simulink model "model"  (R2014a)
(part 1 of 5)
settings: Solver=VariableStepAuto  StartTime=0.0  StopTime=10.0  RelTol=1e-3
libraries: powerlib x1195
settings Model: Creator=lej  LastModifiedBy=leimhofe
settings DataIOCC: SaveFormat=Dataset
settings OptimizationCC: SimCompilerOptimization=off
settings DebuggingCC: MergeDetectMultiDrivingBlocksExec=error  SolverPrmCheckMsg=none  FrameProcessingCompatibilityMsg=error  AllowSymbolicDim=off
settings HardwareCC: ProdBitPerPointer=64  ProdLargestAtomicFloat=Float  ProdIntDivRoundTo=Zero  ProdEndianess=LittleEndian  ProdWordSize=64  ProdHWDeviceType=Intel->x86-64 (Windows64)
settings RTWCC: RTWCompilerOptimization=off
settings GRTTargetCC: GeneratePreprocessorConditionals=Use local settings
settings ConfigComp: CovMetricSettings=dw  CovHtmlReporting=on  CovSaveCumulativeToWorkspaceVar=on  CovSaveSingleToWorkspaceVar=on  CovExternalEMLEnable=off

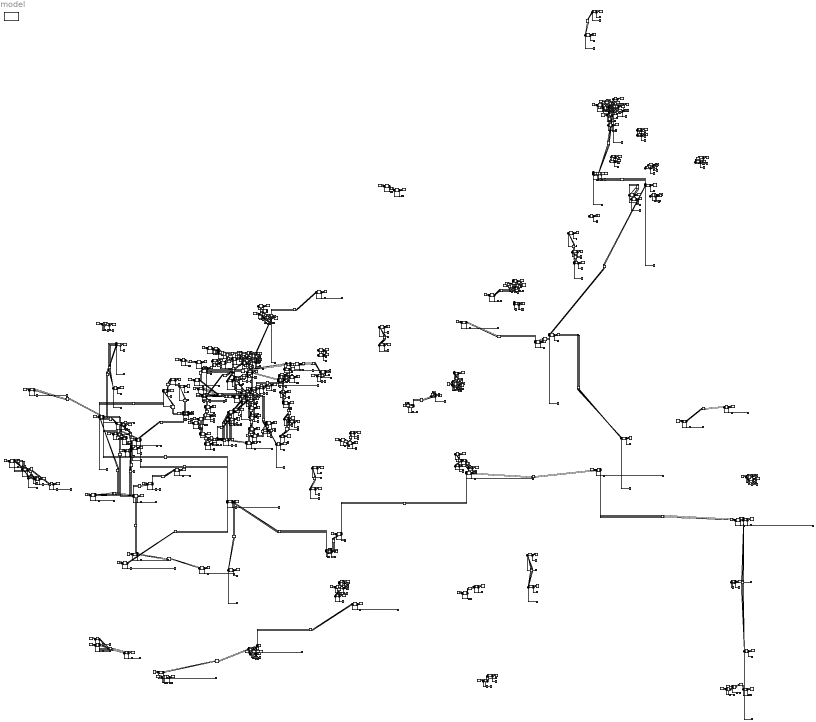
== system model ==
  note: 110000 Volts Power Line
  note: 220000 Volts Power Line
  note: 500000 Volts Power Line
  "110_кВ_\"Лесная_Тормозная\"_CN_242610017_110000_CN_242614771_110000" : powerlib/Elements/Distributed Parameters Line  Phases=3  Frequency=60  Resistance=[0.01273 0.3864]  Inductance="[0.9337e-3  4.1264e-3]"  Capacitance=[12.74e-9 7.751e-9]  Length=5.1805  x1=[0 0 0 0; 0.0001244 0 0 0; 0.0002488 0 0 0; 0.0003733 0 0 0; 0.0004977 0 0 0; 0.0006221 0 0 0]  x2=[0 0 0 0; 0.0001244 0 0 0; 0.0002488 0 0 0; 0.0003733 0 0 0; 0.0004977 0 0 0; 0.0006221 0 0 0]  x3=[0 0 0 0; 0.0001244 0 0 0; 0.0002488 0 0 0; 0.0003733 0 0 0; 0.0004977 0 0 0; 0.0006221 0 0 0]  x4=[0 0 0 0; 0.0001244 0 0 0; 0.0002488 0 0 0; 0.0003733 0 0 0; 0.0004977 0 0 0; 0.0006221 0 0 0]  x5=0  V1=ones(3,3)  V2=ones(3,3)  I1=ones(3,3)  I2=ones(3,3)  nHarmo=1  Measurements=None
  110_кВ_CN_138632781_110000_CN_138722426_110000 : powerlib/Elements/Distributed Parameters Line  Phases=3  Frequency=60  Resistance=[0.01273 0.3864]  Inductance="[0.9337e-3  4.1264e-3]"  Capacitance=[12.74e-9 7.751e-9]  Length=57.9129  x1=[0 0 0 0; 0.0001244 0 0 0; 0.0002488 0 0 0; 0.0003733 0 0 0; 0.0004977 0 0 0; 0.0006221 0 0 0]  x2=[0 0 0 0; 0.0001244 0 0 0; 0.0002488 0 0 0; 0.0003733 0 0 0; 0.0004977 0 0 0; 0.0006221 0 0 0]  x3=[0 0 0 0; 0.0001244 0 0 0; 0.0002488 0 0 0; 0.0003733 0 0 0; 0.0004977 0 0 0; 0.0006221 0 0 0]  x4=[0 0 0 0; 0.0001244 0 0 0; 0.0002488 0 0 0; 0.0003733 0 0 0; 0.0004977 0 0 0; 0.0006221 0 0 0]  x5=0  V1=ones(3,3)  V2=ones(3,3)  I1=ones(3,3)  I2=ones(3,3)  nHarmo=1  Measurements=None
  110_кВ_CN_138632781_110000_CN_140940409_110000 : powerlib/Elements/Distributed Parameters Line  Phases=3  Frequency=60  Resistance=[0.01273 0.3864]  Inductance="[0.9337e-3  4.1264e-3]"  Capacitance=[12.74e-9 7.751e-9]  Length=56.8666  x1=[0 0 0 0; 0.0001244 0 0 0; 0.0002488 0 0 0; 0.0003733 0 0 0; 0.0004977 0 0 0; 0.0006221 0 0 0]  x2=[0 0 0 0; 0.0001244 0 0 0; 0.0002488 0 0 0; 0.0003733 0 0 0; 0.0004977 0 0 0; 0.0006221 0 0 0]  x3=[0 0 0 0; 0.0001244 0 0 0; 0.0002488 0 0 0; 0.0003733 0 0 0; 0.0004977 0 0 0; 0.0006221 0 0 0]  x4=[0 0 0 0; 0.0001244 0 0 0; 0.0002488 0 0 0; 0.0003733 0 0 0; 0.0004977 0 0 0; 0.0006221 0 0 0]  x5=0  V1=ones(3,3)  V2=ones(3,3)  I1=ones(3,3)  I2=ones(3,3)  nHarmo=1  Measurements=None
  110_кВ_CN_138632781_110000_CN_140944227_110000 : powerlib/Elements/Distributed Parameters Line  Phases=3  Frequency=60  Resistance=[0.01273 0.3864]  Inductance="[0.9337e-3  4.1264e-3]"  Capacitance=[12.74e-9 7.751e-9]  Length=80.834  x1=[0 0 0 0; 0.0001244 0 0 0; 0.0002488 0 0 0; 0.0003733 0 0 0; 0.0004977 0 0 0; 0.0006221 0 0 0]  x2=[0 0 0 0; 0.0001244 0 0 0; 0.0002488 0 0 0; 0.0003733 0 0 0; 0.0004977 0 0 0; 0.0006221 0 0 0]  x3=[0 0 0 0; 0.0001244 0 0 0; 0.0002488 0 0 0; 0.0003733 0 0 0; 0.0004977 0 0 0; 0.0006221 0 0 0]  x4=[0 0 0 0; 0.0001244 0 0 0; 0.0002488 0 0 0; 0.0003733 0 0 0; 0.0004977 0 0 0; 0.0006221 0 0 0]  x5=0  V1=ones(3,3)  V2=ones(3,3)  I1=ones(3,3)  I2=ones(3,3)  nHarmo=1  Measurements=None
  110_кВ_CN_138632781_110000_CN_181334375_110000 : powerlib/Elements/Distributed Parameters Line  Phases=3  Frequency=60  Resistance=[0.01273 0.3864]  Inductance="[0.9337e-3  4.1264e-3]"  Capacitance=[12.74e-9 7.751e-9]  Length=34.1326  x1=[0 0 0 0; 0.0001244 0 0 0; 0.0002488 0 0 0; 0.0003733 0 0 0; 0.0004977 0 0 0; 0.0006221 0 0 0]  x2=[0 0 0 0; 0.0001244 0 0 0; 0.0002488 0 0 0; 0.0003733 0 0 0; 0.0004977 0 0 0; 0.0006221 0 0 0]  x3=[0 0 0 0; 0.0001244 0 0 0; 0.0002488 0 0 0; 0.0003733 0 0 0; 0.0004977 0 0 0; 0.0006221 0 0 0]  x4=[0 0 0 0; 0.0001244 0 0 0; 0.0002488 0 0 0; 0.0003733 0 0 0; 0.0004977 0 0 0; 0.0006221 0 0 0]  x5=0  V1=ones(3,3)  V2=ones(3,3)  I1=ones(3,3)  I2=ones(3,3)  nHarmo=1  Measurements=None
  G_104227388_НкТЭЦ_2 : powerlib/Electrical Sources/Three-Phase Source  Voltage=220000  PhaseAngle=0  Frequency=60  InternalConnection=Yg  SpecifyImpedance=on  Resistance=0.8929  Inductance=16.58e-3  ShortCircuitLevel=100e6  BaseVoltage=220000  XRratio=7  BusType=swing  Pref=0  Qref=0  Qmin=-inf  Qmax=inf
  G_104227390_ТЭЦ_2 : powerlib/Electrical Sources/Three-Phase Source  Voltage=110000  PhaseAngle=0  Frequency=60  InternalConnection=Yg  SpecifyImpedance=on  Resistance=0.8929  Inductance=16.58e-3  ShortCircuitLevel=100e6  BaseVoltage=110000  XRratio=7  BusType=swing  Pref=0  Qref=0  Qmin=-inf  Qmax=inf
  G_107881747_Йошкар_Олинская_ТЭЦ_(ТЭЦ_2) : powerlib/Electrical Sources/Three-Phase Source  Voltage=110000  PhaseAngle=0  Frequency=60  InternalConnection=Yg  SpecifyImpedance=on  Resistance=0.8929  Inductance=16.58e-3  ShortCircuitLevel=100e6  BaseVoltage=110000  XRratio=7  BusType=swing  Pref=195000000  Qref=0  Qmin=-inf  Qmax=inf
  G_220103258_Зауральская_ТЭЦ : powerlib/Electrical Sources/Three-Phase Source  Voltage=110000  PhaseAngle=0  Frequency=60  InternalConnection=Yg  SpecifyImpedance=on  Resistance=0.8929  Inductance=16.58e-3  ShortCircuitLevel=100e6  BaseVoltage=110000  XRratio=7  BusType=swing  Pref=0  Qref=0  Qmin=-inf  Qmax=inf
  G_245072101_Жигулёвская_ГЭС : powerlib/Electrical Sources/Three-Phase Source  Voltage=110000  PhaseAngle=0  Frequency=60  InternalConnection=Yg  SpecifyImpedance=on  Resistance=0.8929  Inductance=16.58e-3  ShortCircuitLevel=100e6  BaseVoltage=110000  XRratio=7  BusType=swing  Pref=2404000000  Qref=0  Qmin=-inf  Qmax=inf
  G_273327356_Воткинская_ГЭС : powerlib/Electrical Sources/Three-Phase Source  Voltage=110000  PhaseAngle=0  Frequency=60  InternalConnection=Yg  SpecifyImpedance=on  Resistance=0.8929  Inductance=16.58e-3  ShortCircuitLevel=100e6  BaseVoltage=110000  XRratio=7  BusType=swing  Pref=1020000000  Qref=0  Qmin=-inf  Qmax=inf
  G_48906740_Балаковская_АЭС : powerlib/Electrical Sources/Three-Phase Source  Voltage=500000  PhaseAngle=0  Frequency=60  InternalConnection=Yg  SpecifyImpedance=on  Resistance=0.8929  Inductance=16.58e-3  ShortCircuitLevel=100e6  BaseVoltage=500000  XRratio=7  BusType=swing  Pref=4000000000  Qref=0  Qmin=-inf  Qmax=inf
  G_62191058_Татарская_АЭС : powerlib/Electrical Sources/Three-Phase Source  Voltage=110000  PhaseAngle=0  Frequency=60  InternalConnection=Yg  SpecifyImpedance=on  Resistance=0.8929  Inductance=16.58e-3  ShortCircuitLevel=100e6  BaseVoltage=110000  XRratio=7  BusType=swing  Pref=0  Qref=0  Qmin=-inf  Qmax=inf
  G_83478009_Пермская_ГРЭС : powerlib/Electrical Sources/Three-Phase Source  Voltage=220000  PhaseAngle=0  Frequency=60  InternalConnection=Yg  SpecifyImpedance=on  Resistance=0.8929  Inductance=16.58e-3  ShortCircuitLevel=100e6  BaseVoltage=220000  XRratio=7  BusType=swing  Pref=2400000000  Qref=0  Qmin=-inf  Qmax=inf
  L_{51601242,51711248,53366641,53566695,55334100,55334115,56048772,57948286,58880346,67498838,70186926..70186927,82459148,90682372,90868997,93482493,93482528,94214974,94242892,97060032,97060037,97124768,97124903,97145033,100584516,102447718,103877395,103877470,104554513,106289362,106289442,107692183,107942401,107943661,108403292,108913072,109525394,109525404,109525418,109525439,110255218,110370987,112681450,113994637,115651649,116695174,116695201,120823877,121218185,136761822,137714986,138632781,138722426,140940409,140944227,145399632,157080628,158349331,160723975,161082145,165640869,171977680,172508720,172819864,176642248,176838936,176859804,180390411,180786877,181334375,183273018,190492574,191841753,192426717,192432406..192432407,193928464,194431022,197887411,198002186,207204995,207206840,207740804,208425687,211578632,218733056,218733818,218733820,219889824,222133214,226052064,226054226,226055229,226055643,227673096,229841888,234246987,236703070,238317576,238549570,241262030,242610017,242614771,242619649,242932802,242972920,242973735,243068515,243069892,243075861,243154612,243531233,243820930,244847744,245404985,247403714,250911823,252815157..252815158,262366241..262366242,277905349..277905350,279258960,279778884,279846258,279846262,279919300,279919302,279978581..279978583,279978585..279978588,280247938,280247940,280247942,280247955,280247957,280247962,280247964,280247969,281834842,281834847,281879365,281879368,283379848,286921936,287462706,290776375,290777752,291372085..291372086,292068563,292328535,305832833,307428692,308883878,310752804,311468947,313773131,313773134,315675920,319459210,319459220,320965592,327245366,327245371,327245584,329997654,330006647,330052123,337947383,351596015} (176 alike) : powerlib/Elements/Three-Phase Series RLC Load  LConnTagsString=A|B|C  Configuration=Y (grounded)  NominalVoltage=110000  NominalFrequency=60  ActivePower=100000  InductivePower=100  CapacitivePower=100  Measurements=None  LoadType=constant Z
  L_{48949159,51711046,62194541,72288676,82458858,89430545,92419131,93292147,93494543,93494546,93508340,95488500,95488527,96563667,96826924,103735794,113585698,121048356,128036424,132783542,137376045,158349339,171147802,211405161,224208787,224261932,229942593,232164616,240018999,274213600,274937610,274998912,276080500,305832836,305893253,306106528,327138157,327226015,327226025,327325460,327816066,328463572} (42 alike) : powerlib/Elements/Three-Phase Series RLC Load  LConnTagsString=A|B|C  Configuration=Y (grounded)  NominalVoltage=220000  NominalFrequency=60  ActivePower=100000  InductivePower=100  CapacitivePower=100  Measurements=None  LoadType=constant Z
  L_{53015400,82459105,82967790,88028486,90273320,92325642,99190583,110601218,113767652,114285735,131490223,131508245,136586702,150285837,169556579,193513250,219112646,219655813,227835712,229649869,363144177,376942192} (22 alike) : powerlib/Elements/Three-Phase Series RLC Load  LConnTagsString=A|B|C  Configuration=Y (grounded)  NominalVoltage=500000  NominalFrequency=60  ActivePower=100000  InductivePower=100  CapacitivePower=100  Measurements=None  LoadType=constant Z
  T_100584516__ : powerlib/Elements/Three-Phase Transformer (Two Windings)  Winding1Connection=Yg  UNITS=pu  NominalPower=[ 250e6 , 60 ]  Winding1=[110000,0.002,0.08]  Winding2Connection=Yg  Winding2=[110000,0.002,0.08]  SetSaturation=off  Rm=500  Lm=500  Saturation=[ 0,0 ; 0.0024,1.2 ; 1.0,1.52 ]  Hysteresis=off  DataFile='hysteresis'  SetInitialFlux=off  InitialFluxes=[ 0.8 , -0.8 , 0.7 ]  Measurements=None  MoreParameters=off  BreakLoop=off  DataType=off  TransfoNumber=1
  T_102447718__ : powerlib/Elements/Three-Phase Transformer (Two Windings)  Winding1Connection=Yg  UNITS=pu  NominalPower=[ 250e6 , 60 ]  Winding1=[110000,0.002,0.08]  Winding2Connection=Yg  Winding2=[110000,0.002,0.08]  SetSaturation=off  Rm=500  Lm=500  Saturation=[ 0,0 ; 0.0024,1.2 ; 1.0,1.52 ]  Hysteresis=off  DataFile='hysteresis'  SetInitialFlux=off  InitialFluxes=[ 0.8 , -0.8 , 0.7 ]  Measurements=None  MoreParameters=off  BreakLoop=off  DataType=off  TransfoNumber=1
  T_103735794_220000_Центролит : powerlib/Elements/Three-Phase Transformer (Two Windings)  Winding1Connection=Yg  UNITS=pu  NominalPower=[ 250e6 , 60 ]  Winding1=[220000,0.002,0.08]  Winding2Connection=Yg  Winding2=[220000,0.002,0.08]  SetSaturation=off  Rm=500  Lm=500  Saturation=[ 0,0 ; 0.0024,1.2 ; 1.0,1.52 ]  Hysteresis=off  DataFile='hysteresis'  SetInitialFlux=off  InitialFluxes=[ 0.8 , -0.8 , 0.7 ]  Measurements=None  MoreParameters=off  BreakLoop=off  DataType=off  TransfoNumber=1
  T_103877395__ : powerlib/Elements/Three-Phase Transformer (Two Windings)  Winding1Connection=Yg  UNITS=pu  NominalPower=[ 250e6 , 60 ]  Winding1=[110000,0.002,0.08]  Winding2Connection=Yg  Winding2=[110000,0.002,0.08]  SetSaturation=off  Rm=500  Lm=500  Saturation=[ 0,0 ; 0.0024,1.2 ; 1.0,1.52 ]  Hysteresis=off  DataFile='hysteresis'  SetInitialFlux=off  InitialFluxes=[ 0.8 , -0.8 , 0.7 ]  Measurements=None  MoreParameters=off  BreakLoop=off  DataType=off  TransfoNumber=1
  T_103877470__ : powerlib/Elements/Three-Phase Transformer (Two Windings)  Winding1Connection=Yg  UNITS=pu  NominalPower=[ 250e6 , 60 ]  Winding1=[110000,0.002,0.08]  Winding2Connection=Yg  Winding2=[110000,0.002,0.08]  SetSaturation=off  Rm=500  Lm=500  Saturation=[ 0,0 ; 0.0024,1.2 ; 1.0,1.52 ]  Hysteresis=off  DataFile='hysteresis'  SetInitialFlux=off  InitialFluxes=[ 0.8 , -0.8 , 0.7 ]  Measurements=None  MoreParameters=off  BreakLoop=off  DataType=off  TransfoNumber=1
  T_104554513__ : powerlib/Elements/Three-Phase Transformer (Two Windings)  Winding1Connection=Yg  UNITS=pu  NominalPower=[ 250e6 , 60 ]  Winding1=[110000,0.002,0.08]  Winding2Connection=Yg  Winding2=[110000,0.002,0.08]  SetSaturation=off  Rm=500  Lm=500  Saturation=[ 0,0 ; 0.0024,1.2 ; 1.0,1.52 ]  Hysteresis=off  DataFile='hysteresis'  SetInitialFlux=off  InitialFluxes=[ 0.8 , -0.8 , 0.7 ]  Measurements=None  MoreParameters=off  BreakLoop=off  DataType=off  TransfoNumber=1
  T_106289362__ : powerlib/Elements/Three-Phase Transformer (Two Windings)  Winding1Connection=Yg  UNITS=pu  NominalPower=[ 250e6 , 60 ]  Winding1=[110000,0.002,0.08]  Winding2Connection=Yg  Winding2=[110000,0.002,0.08]  SetSaturation=off  Rm=500  Lm=500  Saturation=[ 0,0 ; 0.0024,1.2 ; 1.0,1.52 ]  Hysteresis=off  DataFile='hysteresis'  SetInitialFlux=off  InitialFluxes=[ 0.8 , -0.8 , 0.7 ]  Measurements=None  MoreParameters=off  BreakLoop=off  DataType=off  TransfoNumber=1
  T_106289442__ : powerlib/Elements/Three-Phase Transformer (Two Windings)  Winding1Connection=Yg  UNITS=pu  NominalPower=[ 250e6 , 60 ]  Winding1=[110000,0.002,0.08]  Winding2Connection=Yg  Winding2=[110000,0.002,0.08]  SetSaturation=off  Rm=500  Lm=500  Saturation=[ 0,0 ; 0.0024,1.2 ; 1.0,1.52 ]  Hysteresis=off  DataFile='hysteresis'  SetInitialFlux=off  InitialFluxes=[ 0.8 , -0.8 , 0.7 ]  Measurements=None  MoreParameters=off  BreakLoop=off  DataType=off  TransfoNumber=1
  T_107692183_220000_ПС_Чигашево_220_110кВ : powerlib/Elements/Three-Phase Transformer (Two Windings)  Winding1Connection=Yg  UNITS=pu  NominalPower=[ 250e6 , 60 ]  Winding1=[220000,0.002,0.08]  Winding2Connection=Yg  Winding2=[110000,0.002,0.08]  SetSaturation=off  Rm=500  Lm=500  Saturation=[ 0,0 ; 0.0024,1.2 ; 1.0,1.52 ]  Hysteresis=off  DataFile='hysteresis'  SetInitialFlux=off  InitialFluxes=[ 0.8 , -0.8 , 0.7 ]  Measurements=None  MoreParameters=off  BreakLoop=off  DataType=off  TransfoNumber=1
  T_107942401__ : powerlib/Elements/Three-Phase Transformer (Two Windings)  Winding1Connection=Yg  UNITS=pu  NominalPower=[ 250e6 , 60 ]  Winding1=[110000,0.002,0.08]  Winding2Connection=Yg  Winding2=[110000,0.002,0.08]  SetSaturation=off  Rm=500  Lm=500  Saturation=[ 0,0 ; 0.0024,1.2 ; 1.0,1.52 ]  Hysteresis=off  DataFile='hysteresis'  SetInitialFlux=off  InitialFluxes=[ 0.8 , -0.8 , 0.7 ]  Measurements=None  MoreParameters=off  BreakLoop=off  DataType=off  TransfoNumber=1
  T_107943661_110000_Медведевский_электроучасток : powerlib/Elements/Three-Phase Transformer (Two Windings)  Winding1Connection=Yg  UNITS=pu  NominalPower=[ 250e6 , 60 ]  Winding1=[110000,0.002,0.08]  Winding2Connection=Yg  Winding2=[110000,0.002,0.08]  SetSaturation=off  Rm=500  Lm=500  Saturation=[ 0,0 ; 0.0024,1.2 ; 1.0,1.52 ]  Hysteresis=off  DataFile='hysteresis'  SetInitialFlux=off  InitialFluxes=[ 0.8 , -0.8 , 0.7 ]  Measurements=None  MoreParameters=off  BreakLoop=off  DataType=off  TransfoNumber=1
  T_108403292__ : powerlib/Elements/Three-Phase Transformer (Two Windings)  Winding1Connection=Yg  UNITS=pu  NominalPower=[ 250e6 , 60 ]  Winding1=[110000,0.002,0.08]  Winding2Connection=Yg  Winding2=[110000,0.002,0.08]  SetSaturation=off  Rm=500  Lm=500  Saturation=[ 0,0 ; 0.0024,1.2 ; 1.0,1.52 ]  Hysteresis=off  DataFile='hysteresis'  SetInitialFlux=off  InitialFluxes=[ 0.8 , -0.8 , 0.7 ]  Measurements=None  MoreParameters=off  BreakLoop=off  DataType=off  TransfoNumber=1
  T_108913072_110000;10000_Подстанция : powerlib/Elements/Three-Phase Transformer (Two Windings)  Winding1Connection=Yg  UNITS=pu  NominalPower=[ 250e6 , 60 ]  Winding1=[110000,0.002,0.08]  Winding2Connection=Yg  Winding2=[110000,0.002,0.08]  SetSaturation=off  Rm=500  Lm=500  Saturation=[ 0,0 ; 0.0024,1.2 ; 1.0,1.52 ]  Hysteresis=off  DataFile='hysteresis'  SetInitialFlux=off  InitialFluxes=[ 0.8 , -0.8 , 0.7 ]  Measurements=None  MoreParameters=off  BreakLoop=off  DataType=off  TransfoNumber=1
  T_109525394_220000_ПС_220_кВ_Калийная : powerlib/Elements/Three-Phase Transformer (Two Windings)  Winding1Connection=Yg  UNITS=pu  NominalPower=[ 250e6 , 60 ]  Winding1=[110000,0.002,0.08]  Winding2Connection=Yg  Winding2=[110000,0.002,0.08]  SetSaturation=off  Rm=500  Lm=500  Saturation=[ 0,0 ; 0.0024,1.2 ; 1.0,1.52 ]  Hysteresis=off  DataFile='hysteresis'  SetInitialFlux=off  InitialFluxes=[ 0.8 , -0.8 , 0.7 ]  Measurements=None  MoreParameters=off  BreakLoop=off  DataType=off  TransfoNumber=1
  T_109525404__ : powerlib/Elements/Three-Phase Transformer (Two Windings)  Winding1Connection=Yg  UNITS=pu  NominalPower=[ 250e6 , 60 ]  Winding1=[110000,0.002,0.08]  Winding2Connection=Yg  Winding2=[110000,0.002,0.08]  SetSaturation=off  Rm=500  Lm=500  Saturation=[ 0,0 ; 0.0024,1.2 ; 1.0,1.52 ]  Hysteresis=off  DataFile='hysteresis'  SetInitialFlux=off  InitialFluxes=[ 0.8 , -0.8 , 0.7 ]  Measurements=None  MoreParameters=off  BreakLoop=off  DataType=off  TransfoNumber=1
  T_109525418_220000_Подстанция_220_кВ_Титан : powerlib/Elements/Three-Phase Transformer (Two Windings)  Winding1Connection=Yg  UNITS=pu  NominalPower=[ 250e6 , 60 ]  Winding1=[110000,0.002,0.08]  Winding2Connection=Yg  Winding2=[110000,0.002,0.08]  SetSaturation=off  Rm=500  Lm=500  Saturation=[ 0,0 ; 0.0024,1.2 ; 1.0,1.52 ]  Hysteresis=off  DataFile='hysteresis'  SetInitialFlux=off  InitialFluxes=[ 0.8 , -0.8 , 0.7 ]  Measurements=None  MoreParameters=off  BreakLoop=off  DataType=off  TransfoNumber=1
  T_109525439__ : powerlib/Elements/Three-Phase Transformer (Two Windings)  Winding1Connection=Yg  UNITS=pu  NominalPower=[ 250e6 , 60 ]  Winding1=[110000,0.002,0.08]  Winding2Connection=Yg  Winding2=[110000,0.002,0.08]  SetSaturation=off  Rm=500  Lm=500  Saturation=[ 0,0 ; 0.0024,1.2 ; 1.0,1.52 ]  Hysteresis=off  DataFile='hysteresis'  SetInitialFlux=off  InitialFluxes=[ 0.8 , -0.8 , 0.7 ]  Measurements=None  MoreParameters=off  BreakLoop=off  DataType=off  TransfoNumber=1
  T_110255218__ПС_Кожино_110_35кВ : powerlib/Elements/Three-Phase Transformer (Two Windings)  Winding1Connection=Yg  UNITS=pu  NominalPower=[ 250e6 , 60 ]  Winding1=[110000,0.002,0.08]  Winding2Connection=Yg  Winding2=[110000,0.002,0.08]  SetSaturation=off  Rm=500  Lm=500  Saturation=[ 0,0 ; 0.0024,1.2 ; 1.0,1.52 ]  Hysteresis=off  DataFile='hysteresis'  SetInitialFlux=off  InitialFluxes=[ 0.8 , -0.8 , 0.7 ]  Measurements=None  MoreParameters=off  BreakLoop=off  DataType=off  TransfoNumber=1
  T_110370987__ПС_Краснооктябрьск_110_10кВ : powerlib/Elements/Three-Phase Transformer (Two Windings)  Winding1Connection=Yg  UNITS=pu  NominalPower=[ 250e6 , 60 ]  Winding1=[110000,0.002,0.08]  Winding2Connection=Yg  Winding2=[110000,0.002,0.08]  SetSaturation=off  Rm=500  Lm=500  Saturation=[ 0,0 ; 0.0024,1.2 ; 1.0,1.52 ]  Hysteresis=off  DataFile='hysteresis'  SetInitialFlux=off  InitialFluxes=[ 0.8 , -0.8 , 0.7 ]  Measurements=None  MoreParameters=off  BreakLoop=off  DataType=off  TransfoNumber=1
  T_110601218_500000_ : powerlib/Elements/Three-Phase Transformer (Two Windings)  Winding1Connection=Yg  UNITS=pu  NominalPower=[ 250e6 , 60 ]  Winding1=[500000,0.002,0.08]  Winding2Connection=Yg  Winding2=[500000,0.002,0.08]  SetSaturation=off  Rm=500  Lm=500  Saturation=[ 0,0 ; 0.0024,1.2 ; 1.0,1.52 ]  Hysteresis=off  DataFile='hysteresis'  SetInitialFlux=off  InitialFluxes=[ 0.8 , -0.8 , 0.7 ]  Measurements=None  MoreParameters=off  BreakLoop=off  DataType=off  TransfoNumber=1
  T_112681450_110000_ : powerlib/Elements/Three-Phase Transformer (Two Windings)  Winding1Connection=Yg  UNITS=pu  NominalPower=[ 250e6 , 60 ]  Winding1=[110000,0.002,0.08]  Winding2Connection=Yg  Winding2=[110000,0.002,0.08]  SetSaturation=off  Rm=500  Lm=500  Saturation=[ 0,0 ; 0.0024,1.2 ; 1.0,1.52 ]  Hysteresis=off  DataFile='hysteresis'  SetInitialFlux=off  InitialFluxes=[ 0.8 , -0.8 , 0.7 ]  Measurements=None  MoreParameters=off  BreakLoop=off  DataType=off  TransfoNumber=1
  T_113585698_220000_ПС_220кВ_Рузаевка : powerlib/Elements/Three-Phase Transformer (Two Windings)  Winding1Connection=Yg  UNITS=pu  NominalPower=[ 250e6 , 60 ]  Winding1=[220000,0.002,0.08]  Winding2Connection=Yg  Winding2=[220000,0.002,0.08]  SetSaturation=off  Rm=500  Lm=500  Saturation=[ 0,0 ; 0.0024,1.2 ; 1.0,1.52 ]  Hysteresis=off  DataFile='hysteresis'  SetInitialFlux=off  InitialFluxes=[ 0.8 , -0.8 , 0.7 ]  Measurements=None  MoreParameters=off  BreakLoop=off  DataType=off  TransfoNumber=1
  T_113767652_500000_ПС_Кропачево : powerlib/Elements/Three-Phase Transformer (Two Windings)  Winding1Connection=Yg  UNITS=pu  NominalPower=[ 250e6 , 60 ]  Winding1=[500000,0.002,0.08]  Winding2Connection=Yg  Winding2=[500000,0.002,0.08]  SetSaturation=off  Rm=500  Lm=500  Saturation=[ 0,0 ; 0.0024,1.2 ; 1.0,1.52 ]  Hysteresis=off  DataFile='hysteresis'  SetInitialFlux=off  InitialFluxes=[ 0.8 , -0.8 , 0.7 ]  Measurements=None  MoreParameters=off  BreakLoop=off  DataType=off  TransfoNumber=1
  T_113994637__ПС_Буинск : powerlib/Elements/Three-Phase Transformer (Two Windings)  Winding1Connection=Yg  UNITS=pu  NominalPower=[ 250e6 , 60 ]  Winding1=[110000,0.002,0.08]  Winding2Connection=Yg  Winding2=[110000,0.002,0.08]  SetSaturation=off  Rm=500  Lm=500  Saturation=[ 0,0 ; 0.0024,1.2 ; 1.0,1.52 ]  Hysteresis=off  DataFile='hysteresis'  SetInitialFlux=off  InitialFluxes=[ 0.8 , -0.8 , 0.7 ]  Measurements=None  MoreParameters=off  BreakLoop=off  DataType=off  TransfoNumber=1
  T_114285735_500000;220000;10000_ПС_Уфимская : powerlib/Elements/Three-Phase Transformer (Two Windings)  Winding1Connection=Yg  UNITS=pu  NominalPower=[ 250e6 , 60 ]  Winding1=[500000,0.002,0.08]  Winding2Connection=Yg  Winding2=[500000,0.002,0.08]  SetSaturation=off  Rm=500  Lm=500  Saturation=[ 0,0 ; 0.0024,1.2 ; 1.0,1.52 ]  Hysteresis=off  DataFile='hysteresis'  SetInitialFlux=off  InitialFluxes=[ 0.8 , -0.8 , 0.7 ]  Measurements=None  MoreParameters=off  BreakLoop=off  DataType=off  TransfoNumber=1
  T_115651649_110000;10000_ПС_110_10_кВ_Вурманкасы : powerlib/Elements/Three-Phase Transformer (Two Windings)  Winding1Connection=Yg  UNITS=pu  NominalPower=[ 250e6 , 60 ]  Winding1=[110000,0.002,0.08]  Winding2Connection=Yg  Winding2=[110000,0.002,0.08]  SetSaturation=off  Rm=500  Lm=500  Saturation=[ 0,0 ; 0.0024,1.2 ; 1.0,1.52 ]  Hysteresis=off  DataFile='hysteresis'  SetInitialFlux=off  InitialFluxes=[ 0.8 , -0.8 , 0.7 ]  Measurements=None  MoreParameters=off  BreakLoop=off  DataType=off  TransfoNumber=1
  T_116695174_110000_ПС_110_6_кВ_Инструментальная : powerlib/Elements/Three-Phase Transformer (Two Windings)  Winding1Connection=Yg  UNITS=pu  NominalPower=[ 250e6 , 60 ]  Winding1=[110000,0.002,0.08]  Winding2Connection=Yg  Winding2=[110000,0.002,0.08]  SetSaturation=off  Rm=500  Lm=500  Saturation=[ 0,0 ; 0.0024,1.2 ; 1.0,1.52 ]  Hysteresis=off  DataFile='hysteresis'  SetInitialFlux=off  InitialFluxes=[ 0.8 , -0.8 , 0.7 ]  Measurements=None  MoreParameters=off  BreakLoop=off  DataType=off  TransfoNumber=1
  T_116695201_110000_ПС_110_35_6_Воткинск : powerlib/Elements/Three-Phase Transformer (Two Windings)  Winding1Connection=Yg  UNITS=pu  NominalPower=[ 250e6 , 60 ]  Winding1=[110000,0.002,0.08]  Winding2Connection=Yg  Winding2=[110000,0.002,0.08]  SetSaturation=off  Rm=500  Lm=500  Saturation=[ 0,0 ; 0.0024,1.2 ; 1.0,1.52 ]  Hysteresis=off  DataFile='hysteresis'  SetInitialFlux=off  InitialFluxes=[ 0.8 , -0.8 , 0.7 ]  Measurements=None  MoreParameters=off  BreakLoop=off  DataType=off  TransfoNumber=1
  T_120823877__ПС_Федоровская : powerlib/Elements/Three-Phase Transformer (Two Windings)  Winding1Connection=Yg  UNITS=pu  NominalPower=[ 250e6 , 60 ]  Winding1=[110000,0.002,0.08]  Winding2Connection=Yg  Winding2=[110000,0.002,0.08]  SetSaturation=off  Rm=500  Lm=500  Saturation=[ 0,0 ; 0.0024,1.2 ; 1.0,1.52 ]  Hysteresis=off  DataFile='hysteresis'  SetInitialFlux=off  InitialFluxes=[ 0.8 , -0.8 , 0.7 ]  Measurements=None  MoreParameters=off  BreakLoop=off  DataType=off  TransfoNumber=1
  "T_121048356_220000_ПС_220кВ_\"Бобыльская\"" : powerlib/Elements/Three-Phase Transformer (Two Windings)  Winding1Connection=Yg  UNITS=pu  NominalPower=[ 250e6 , 60 ]  Winding1=[220000,0.002,0.08]  Winding2Connection=Yg  Winding2=[220000,0.002,0.08]  SetSaturation=off  Rm=500  Lm=500  Saturation=[ 0,0 ; 0.0024,1.2 ; 1.0,1.52 ]  Hysteresis=off  DataFile='hysteresis'  SetInitialFlux=off  InitialFluxes=[ 0.8 , -0.8 , 0.7 ]  Measurements=None  MoreParameters=off  BreakLoop=off  DataType=off  TransfoNumber=1
  T_121218185_220000;110000;10000_ПС_220_110_10_кВ_Тюрлема : powerlib/Elements/Three-Phase Transformer (Two Windings)  Winding1Connection=Yg  UNITS=pu  NominalPower=[ 250e6 , 60 ]  Winding1=[220000,0.002,0.08]  Winding2Connection=Yg  Winding2=[110000,0.002,0.08]  SetSaturation=off  Rm=500  Lm=500  Saturation=[ 0,0 ; 0.0024,1.2 ; 1.0,1.52 ]  Hysteresis=off  DataFile='hysteresis'  SetInitialFlux=off  InitialFluxes=[ 0.8 , -0.8 , 0.7 ]  Measurements=None  MoreParameters=off  BreakLoop=off  DataType=off  TransfoNumber=1
  T_128036424_500000;220000_Северная : powerlib/Elements/Three-Phase Transformer (Two Windings)  Winding1Connection=Yg  UNITS=pu  NominalPower=[ 250e6 , 60 ]  Winding1=[500000,0.002,0.08]  Winding2Connection=Yg  Winding2=[220000,0.002,0.08]  SetSaturation=off  Rm=500  Lm=500  Saturation=[ 0,0 ; 0.0024,1.2 ; 1.0,1.52 ]  Hysteresis=off  DataFile='hysteresis'  SetInitialFlux=off  InitialFluxes=[ 0.8 , -0.8 , 0.7 ]  Measurements=None  MoreParameters=off  BreakLoop=off  DataType=off  TransfoNumber=1
  T_131490223__ПС_Вешкайма : powerlib/Elements/Three-Phase Transformer (Two Windings)  Winding1Connection=Yg  UNITS=pu  NominalPower=[ 250e6 , 60 ]  Winding1=[500000,0.002,0.08]  Winding2Connection=Yg  Winding2=[500000,0.002,0.08]  SetSaturation=off  Rm=500  Lm=500  Saturation=[ 0,0 ; 0.0024,1.2 ; 1.0,1.52 ]  Hysteresis=off  DataFile='hysteresis'  SetInitialFlux=off  InitialFluxes=[ 0.8 , -0.8 , 0.7 ]  Measurements=None  MoreParameters=off  BreakLoop=off  DataType=off  TransfoNumber=1
  T_131508245_500000_ПС_Ключики : powerlib/Elements/Three-Phase Transformer (Two Windings)  Winding1Connection=Yg  UNITS=pu  NominalPower=[ 250e6 , 60 ]  Winding1=[500000,0.002,0.08]  Winding2Connection=Yg  Winding2=[500000,0.002,0.08]  SetSaturation=off  Rm=500  Lm=500  Saturation=[ 0,0 ; 0.0024,1.2 ; 1.0,1.52 ]  Hysteresis=off  DataFile='hysteresis'  SetInitialFlux=off  InitialFluxes=[ 0.8 , -0.8 , 0.7 ]  Measurements=None  MoreParameters=off  BreakLoop=off  DataType=off  TransfoNumber=1
  T_132783542_220000_ПС_Волжская : powerlib/Elements/Three-Phase Transformer (Two Windings)  Winding1Connection=Yg  UNITS=pu  NominalPower=[ 250e6 , 60 ]  Winding1=[220000,0.002,0.08]  Winding2Connection=Yg  Winding2=[220000,0.002,0.08]  SetSaturation=off  Rm=500  Lm=500  Saturation=[ 0,0 ; 0.0024,1.2 ; 1.0,1.52 ]  Hysteresis=off  DataFile='hysteresis'  SetInitialFlux=off  InitialFluxes=[ 0.8 , -0.8 , 0.7 ]  Measurements=None  MoreParameters=off  BreakLoop=off  DataType=off  TransfoNumber=1
  T_136586702_500000;220000;110000_ПС_Азот : powerlib/Elements/Three-Phase Transformer (Two Windings)  Winding1Connection=Yg  UNITS=pu  NominalPower=[ 250e6 , 60 ]  Winding1=[500000,0.002,0.08]  Winding2Connection=Yg  Winding2=[500000,0.002,0.08]  SetSaturation=off  Rm=500  Lm=500  Saturation=[ 0,0 ; 0.0024,1.2 ; 1.0,1.52 ]  Hysteresis=off  DataFile='hysteresis'  SetInitialFlux=off  InitialFluxes=[ 0.8 , -0.8 , 0.7 ]  Measurements=None  MoreParameters=off  BreakLoop=off  DataType=off  TransfoNumber=1
  T_136761822_110000_ : powerlib/Elements/Three-Phase Transformer (Two Windings)  Winding1Connection=Yg  UNITS=pu  NominalPower=[ 250e6 , 60 ]  Winding1=[110000,0.002,0.08]  Winding2Connection=Yg  Winding2=[110000,0.002,0.08]  SetSaturation=off  Rm=500  Lm=500  Saturation=[ 0,0 ; 0.0024,1.2 ; 1.0,1.52 ]  Hysteresis=off  DataFile='hysteresis'  SetInitialFlux=off  InitialFluxes=[ 0.8 , -0.8 , 0.7 ]  Measurements=None  MoreParameters=off  BreakLoop=off  DataType=off  TransfoNumber=1
  T_137376045__ : powerlib/Elements/Three-Phase Transformer (Two Windings)  Winding1Connection=Yg  UNITS=pu  NominalPower=[ 250e6 , 60 ]  Winding1=[220000,0.002,0.08]  Winding2Connection=Yg  Winding2=[220000,0.002,0.08]  SetSaturation=off  Rm=500  Lm=500  Saturation=[ 0,0 ; 0.0024,1.2 ; 1.0,1.52 ]  Hysteresis=off  DataFile='hysteresis'  SetInitialFlux=off  InitialFluxes=[ 0.8 , -0.8 , 0.7 ]  Measurements=None  MoreParameters=off  BreakLoop=off  DataType=off  TransfoNumber=1
  T_137714986__ : powerlib/Elements/Three-Phase Transformer (Two Windings)  Winding1Connection=Yg  UNITS=pu  NominalPower=[ 250e6 , 60 ]  Winding1=[110000,0.002,0.08]  Winding2Connection=Yg  Winding2=[110000,0.002,0.08]  SetSaturation=off  Rm=500  Lm=500  Saturation=[ 0,0 ; 0.0024,1.2 ; 1.0,1.52 ]  Hysteresis=off  DataFile='hysteresis'  SetInitialFlux=off  InitialFluxes=[ 0.8 , -0.8 , 0.7 ]  Measurements=None  MoreParameters=off  BreakLoop=off  DataType=off  TransfoNumber=1
  "T_138632781_220000;110000;10000_ПС_220_110_10_кВ_\"Сасово\"" : powerlib/Elements/Three-Phase Transformer (Two Windings)  Winding1Connection=Yg  UNITS=pu  NominalPower=[ 250e6 , 60 ]  Winding1=[110000,0.002,0.08]  Winding2Connection=Yg  Winding2=[110000,0.002,0.08]  SetSaturation=off  Rm=500  Lm=500  Saturation=[ 0,0 ; 0.0024,1.2 ; 1.0,1.52 ]  Hysteresis=off  DataFile='hysteresis'  SetInitialFlux=off  InitialFluxes=[ 0.8 , -0.8 , 0.7 ]  Measurements=None  MoreParameters=off  BreakLoop=off  DataType=off  TransfoNumber=1
  "T_138722426__ПС_110_10кВ_\"Вад\"" : powerlib/Elements/Three-Phase Transformer (Two Windings)  Winding1Connection=Yg  UNITS=pu  NominalPower=[ 250e6 , 60 ]  Winding1=[110000,0.002,0.08]  Winding2Connection=Yg  Winding2=[110000,0.002,0.08]  SetSaturation=off  Rm=500  Lm=500  Saturation=[ 0,0 ; 0.0024,1.2 ; 1.0,1.52 ]  Hysteresis=off  DataFile='hysteresis'  SetInitialFlux=off  InitialFluxes=[ 0.8 , -0.8 , 0.7 ]  Measurements=None  MoreParameters=off  BreakLoop=off  DataType=off  TransfoNumber=1
  "T_140940409_110000;10000_ПС_110_10_кВ_\"Свобода\"" : powerlib/Elements/Three-Phase Transformer (Two Windings)  Winding1Connection=Yg  UNITS=pu  NominalPower=[ 250e6 , 60 ]  Winding1=[110000,0.002,0.08]  Winding2Connection=Yg  Winding2=[110000,0.002,0.08]  SetSaturation=off  Rm=500  Lm=500  Saturation=[ 0,0 ; 0.0024,1.2 ; 1.0,1.52 ]  Hysteresis=off  DataFile='hysteresis'  SetInitialFlux=off  InitialFluxes=[ 0.8 , -0.8 , 0.7 ]  Measurements=None  MoreParameters=off  BreakLoop=off  DataType=off  TransfoNumber=1
  T_140944227__ : powerlib/Elements/Three-Phase Transformer (Two Windings)  Winding1Connection=Yg  UNITS=pu  NominalPower=[ 250e6 , 60 ]  Winding1=[110000,0.002,0.08]  Winding2Connection=Yg  Winding2=[110000,0.002,0.08]  SetSaturation=off  Rm=500  Lm=500  Saturation=[ 0,0 ; 0.0024,1.2 ; 1.0,1.52 ]  Hysteresis=off  DataFile='hysteresis'  SetInitialFlux=off  InitialFluxes=[ 0.8 , -0.8 , 0.7 ]  Measurements=None  MoreParameters=off  BreakLoop=off  DataType=off  TransfoNumber=1
  T_145399632__ : powerlib/Elements/Three-Phase Transformer (Two Windings)  Winding1Connection=Yg  UNITS=pu  NominalPower=[ 250e6 , 60 ]  Winding1=[110000,0.002,0.08]  Winding2Connection=Yg  Winding2=[110000,0.002,0.08]  SetSaturation=off  Rm=500  Lm=500  Saturation=[ 0,0 ; 0.0024,1.2 ; 1.0,1.52 ]  Hysteresis=off  DataFile='hysteresis'  SetInitialFlux=off  InitialFluxes=[ 0.8 , -0.8 , 0.7 ]  Measurements=None  MoreParameters=off  BreakLoop=off  DataType=off  TransfoNumber=1
  T_150285837_500000;220000;110000_ПС_Бекетово : powerlib/Elements/Three-Phase Transformer (Two Windings)  Winding1Connection=Yg  UNITS=pu  NominalPower=[ 250e6 , 60 ]  Winding1=[500000,0.002,0.08]  Winding2Connection=Yg  Winding2=[500000,0.002,0.08]  SetSaturation=off  Rm=500  Lm=500  Saturation=[ 0,0 ; 0.0024,1.2 ; 1.0,1.52 ]  Hysteresis=off  DataFile='hysteresis'  SetInitialFlux=off  InitialFluxes=[ 0.8 , -0.8 , 0.7 ]  Measurements=None  MoreParameters=off  BreakLoop=off  DataType=off  TransfoNumber=1
  T_157080628__ : powerlib/Elements/Three-Phase Transformer (Two Windings)  Winding1Connection=Yg  UNITS=pu  NominalPower=[ 250e6 , 60 ]  Winding1=[110000,0.002,0.08]  Winding2Connection=Yg  Winding2=[110000,0.002,0.08]  SetSaturation=off  Rm=500  Lm=500  Saturation=[ 0,0 ; 0.0024,1.2 ; 1.0,1.52 ]  Hysteresis=off  DataFile='hysteresis'  SetInitialFlux=off  InitialFluxes=[ 0.8 , -0.8 , 0.7 ]  Measurements=None  MoreParameters=off  BreakLoop=off  DataType=off  TransfoNumber=1
  T_158349331__ : powerlib/Elements/Three-Phase Transformer (Two Windings)  Winding1Connection=Yg  UNITS=pu  NominalPower=[ 250e6 , 60 ]  Winding1=[110000,0.002,0.08]  Winding2Connection=Yg  Winding2=[110000,0.002,0.08]  SetSaturation=off  Rm=500  Lm=500  Saturation=[ 0,0 ; 0.0024,1.2 ; 1.0,1.52 ]  Hysteresis=off  DataFile='hysteresis'  SetInitialFlux=off  InitialFluxes=[ 0.8 , -0.8 , 0.7 ]  Measurements=None  MoreParameters=off  BreakLoop=off  DataType=off  TransfoNumber=1
  T_158349339_220000_Подстанция_220_кВ_Космос : powerlib/Elements/Three-Phase Transformer (Two Windings)  Winding1Connection=Yg  UNITS=pu  NominalPower=[ 250e6 , 60 ]  Winding1=[220000,0.002,0.08]  Winding2Connection=Yg  Winding2=[220000,0.002,0.08]  SetSaturation=off  Rm=500  Lm=500  Saturation=[ 0,0 ; 0.0024,1.2 ; 1.0,1.52 ]  Hysteresis=off  DataFile='hysteresis'  SetInitialFlux=off  InitialFluxes=[ 0.8 , -0.8 , 0.7 ]  Measurements=None  MoreParameters=off  BreakLoop=off  DataType=off  TransfoNumber=1
  T_160723975_110000;35000;10000_ПС_110_35_10_кВ_Чапаевская : powerlib/Elements/Three-Phase Transformer (Two Windings)  Winding1Connection=Yg  UNITS=pu  NominalPower=[ 250e6 , 60 ]  Winding1=[110000,0.002,0.08]  Winding2Connection=Yg  Winding2=[110000,0.002,0.08]  SetSaturation=off  Rm=500  Lm=500  Saturation=[ 0,0 ; 0.0024,1.2 ; 1.0,1.52 ]  Hysteresis=off  DataFile='hysteresis'  SetInitialFlux=off  InitialFluxes=[ 0.8 , -0.8 , 0.7 ]  Measurements=None  MoreParameters=off  BreakLoop=off  DataType=off  TransfoNumber=1
  T_161082145_220000_ПС_220_кВ_Томыловская : powerlib/Elements/Three-Phase Transformer (Two Windings)  Winding1Connection=Yg  UNITS=pu  NominalPower=[ 250e6 , 60 ]  Winding1=[220000,0.002,0.08]  Winding2Connection=Yg  Winding2=[110000,0.002,0.08]  SetSaturation=off  Rm=500  Lm=500  Saturation=[ 0,0 ; 0.0024,1.2 ; 1.0,1.52 ]  Hysteresis=off  DataFile='hysteresis'  SetInitialFlux=off  InitialFluxes=[ 0.8 , -0.8 , 0.7 ]  Measurements=None  MoreParameters=off  BreakLoop=off  DataType=off  TransfoNumber=1
  T_165640869__ : powerlib/Elements/Three-Phase Transformer (Two Windings)  Winding1Connection=Yg  UNITS=pu  NominalPower=[ 250e6 , 60 ]  Winding1=[110000,0.002,0.08]  Winding2Connection=Yg  Winding2=[110000,0.002,0.08]  SetSaturation=off  Rm=500  Lm=500  Saturation=[ 0,0 ; 0.0024,1.2 ; 1.0,1.52 ]  Hysteresis=off  DataFile='hysteresis'  SetInitialFlux=off  InitialFluxes=[ 0.8 , -0.8 , 0.7 ]  Measurements=None  MoreParameters=off  BreakLoop=off  DataType=off  TransfoNumber=1
  T_169556579__ПC_Приваловская_500_кВ : powerlib/Elements/Three-Phase Transformer (Two Windings)  Winding1Connection=Yg  UNITS=pu  NominalPower=[ 250e6 , 60 ]  Winding1=[500000,0.002,0.08]  Winding2Connection=Yg  Winding2=[500000,0.002,0.08]  SetSaturation=off  Rm=500  Lm=500  Saturation=[ 0,0 ; 0.0024,1.2 ; 1.0,1.52 ]  Hysteresis=off  DataFile='hysteresis'  SetInitialFlux=off  InitialFluxes=[ 0.8 , -0.8 , 0.7 ]  Measurements=None  MoreParameters=off  BreakLoop=off  DataType=off  TransfoNumber=1
  T_171147802__ : powerlib/Elements/Three-Phase Transformer (Two Windings)  Winding1Connection=Yg  UNITS=pu  NominalPower=[ 250e6 , 60 ]  Winding1=[220000,0.002,0.08]  Winding2Connection=Yg  Winding2=[220000,0.002,0.08]  SetSaturation=off  Rm=500  Lm=500  Saturation=[ 0,0 ; 0.0024,1.2 ; 1.0,1.52 ]  Hysteresis=off  DataFile='hysteresis'  SetInitialFlux=off  InitialFluxes=[ 0.8 , -0.8 , 0.7 ]  Measurements=None  MoreParameters=off  BreakLoop=off  DataType=off  TransfoNumber=1
  T_171977680__ПС_Апастово : powerlib/Elements/Three-Phase Transformer (Two Windings)  Winding1Connection=Yg  UNITS=pu  NominalPower=[ 250e6 , 60 ]  Winding1=[110000,0.002,0.08]  Winding2Connection=Yg  Winding2=[110000,0.002,0.08]  SetSaturation=off  Rm=500  Lm=500  Saturation=[ 0,0 ; 0.0024,1.2 ; 1.0,1.52 ]  Hysteresis=off  DataFile='hysteresis'  SetInitialFlux=off  InitialFluxes=[ 0.8 , -0.8 , 0.7 ]  Measurements=None  MoreParameters=off  BreakLoop=off  DataType=off  TransfoNumber=1
  T_172508720_110000_ПС_110_10_Успенка : powerlib/Elements/Three-Phase Transformer (Two Windings)  Winding1Connection=Yg  UNITS=pu  NominalPower=[ 250e6 , 60 ]  Winding1=[110000,0.002,0.08]  Winding2Connection=Yg  Winding2=[110000,0.002,0.08]  SetSaturation=off  Rm=500  Lm=500  Saturation=[ 0,0 ; 0.0024,1.2 ; 1.0,1.52 ]  Hysteresis=off  DataFile='hysteresis'  SetInitialFlux=off  InitialFluxes=[ 0.8 , -0.8 , 0.7 ]  Measurements=None  MoreParameters=off  BreakLoop=off  DataType=off  TransfoNumber=1
  T_172819864__Содовая_1_110_35_6 : powerlib/Elements/Three-Phase Transformer (Two Windings)  Winding1Connection=Yg  UNITS=pu  NominalPower=[ 250e6 , 60 ]  Winding1=[110000,0.002,0.08]  Winding2Connection=Yg  Winding2=[110000,0.002,0.08]  SetSaturation=off  Rm=500  Lm=500  Saturation=[ 0,0 ; 0.0024,1.2 ; 1.0,1.52 ]  Hysteresis=off  DataFile='hysteresis'  SetInitialFlux=off  InitialFluxes=[ 0.8 , -0.8 , 0.7 ]  Measurements=None  MoreParameters=off  BreakLoop=off  DataType=off  TransfoNumber=1
  T_176642248__Елшанка_2 : powerlib/Elements/Three-Phase Transformer (Two Windings)  Winding1Connection=Yg  UNITS=pu  NominalPower=[ 250e6 , 60 ]  Winding1=[110000,0.002,0.08]  Winding2Connection=Yg  Winding2=[110000,0.002,0.08]  SetSaturation=off  Rm=500  Lm=500  Saturation=[ 0,0 ; 0.0024,1.2 ; 1.0,1.52 ]  Hysteresis=off  DataFile='hysteresis'  SetInitialFlux=off  InitialFluxes=[ 0.8 , -0.8 , 0.7 ]  Measurements=None  MoreParameters=off  BreakLoop=off  DataType=off  TransfoNumber=1
  T_176838936__ПС_Каратун : powerlib/Elements/Three-Phase Transformer (Two Windings)  Winding1Connection=Yg  UNITS=pu  NominalPower=[ 250e6 , 60 ]  Winding1=[110000,0.002,0.08]  Winding2Connection=Yg  Winding2=[110000,0.002,0.08]  SetSaturation=off  Rm=500  Lm=500  Saturation=[ 0,0 ; 0.0024,1.2 ; 1.0,1.52 ]  Hysteresis=off  DataFile='hysteresis'  SetInitialFlux=off  InitialFluxes=[ 0.8 , -0.8 , 0.7 ]  Measurements=None  MoreParameters=off  BreakLoop=off  DataType=off  TransfoNumber=1
  T_176859804__Жасминная : powerlib/Elements/Three-Phase Transformer (Two Windings)  Winding1Connection=Yg  UNITS=pu  NominalPower=[ 250e6 , 60 ]  Winding1=[110000,0.002,0.08]  Winding2Connection=Yg  Winding2=[110000,0.002,0.08]  SetSaturation=off  Rm=500  Lm=500  Saturation=[ 0,0 ; 0.0024,1.2 ; 1.0,1.52 ]  Hysteresis=off  DataFile='hysteresis'  SetInitialFlux=off  InitialFluxes=[ 0.8 , -0.8 , 0.7 ]  Measurements=None  MoreParameters=off  BreakLoop=off  DataType=off  TransfoNumber=1
  T_180390411__ПС_Бугульма : powerlib/Elements/Three-Phase Transformer (Two Windings)  Winding1Connection=Yg  UNITS=pu  NominalPower=[ 250e6 , 60 ]  Winding1=[110000,0.002,0.08]  Winding2Connection=Yg  Winding2=[110000,0.002,0.08]  SetSaturation=off  Rm=500  Lm=500  Saturation=[ 0,0 ; 0.0024,1.2 ; 1.0,1.52 ]  Hysteresis=off  DataFile='hysteresis'  SetInitialFlux=off  InitialFluxes=[ 0.8 , -0.8 , 0.7 ]  Measurements=None  MoreParameters=off  BreakLoop=off  DataType=off  TransfoNumber=1
  T_180786877__ПС_Алат : powerlib/Elements/Three-Phase Transformer (Two Windings)  Winding1Connection=Yg  UNITS=pu  NominalPower=[ 250e6 , 60 ]  Winding1=[110000,0.002,0.08]  Winding2Connection=Yg  Winding2=[110000,0.002,0.08]  SetSaturation=off  Rm=500  Lm=500  Saturation=[ 0,0 ; 0.0024,1.2 ; 1.0,1.52 ]  Hysteresis=off  DataFile='hysteresis'  SetInitialFlux=off  InitialFluxes=[ 0.8 , -0.8 , 0.7 ]  Measurements=None  MoreParameters=off  BreakLoop=off  DataType=off  TransfoNumber=1
  "T_181334375__ПС_110_10кВ_\"Кустаревка\"" : powerlib/Elements/Three-Phase Transformer (Two Windings)  Winding1Connection=Yg  UNITS=pu  NominalPower=[ 250e6 , 60 ]  Winding1=[110000,0.002,0.08]  Winding2Connection=Yg  Winding2=[110000,0.002,0.08]  SetSaturation=off  Rm=500  Lm=500  Saturation=[ 0,0 ; 0.0024,1.2 ; 1.0,1.52 ]  Hysteresis=off  DataFile='hysteresis'  SetInitialFlux=off  InitialFluxes=[ 0.8 , -0.8 , 0.7 ]  Measurements=None  MoreParameters=off  BreakLoop=off  DataType=off  TransfoNumber=1
  T_183273018__ПС_Салманы : powerlib/Elements/Three-Phase Transformer (Two Windings)  Winding1Connection=Yg  UNITS=pu  NominalPower=[ 250e6 , 60 ]  Winding1=[110000,0.002,0.08]  Winding2Connection=Yg  Winding2=[110000,0.002,0.08]  SetSaturation=off  Rm=500  Lm=500  Saturation=[ 0,0 ; 0.0024,1.2 ; 1.0,1.52 ]  Hysteresis=off  DataFile='hysteresis'  SetInitialFlux=off  InitialFluxes=[ 0.8 , -0.8 , 0.7 ]  Measurements=None  MoreParameters=off  BreakLoop=off  DataType=off  TransfoNumber=1
  T_190492574__ : powerlib/Elements/Three-Phase Transformer (Two Windings)  Winding1Connection=Yg  UNITS=pu  NominalPower=[ 250e6 , 60 ]  Winding1=[110000,0.002,0.08]  Winding2Connection=Yg  Winding2=[110000,0.002,0.08]  SetSaturation=off  Rm=500  Lm=500  Saturation=[ 0,0 ; 0.0024,1.2 ; 1.0,1.52 ]  Hysteresis=off  DataFile='hysteresis'  SetInitialFlux=off  InitialFluxes=[ 0.8 , -0.8 , 0.7 ]  Measurements=None  MoreParameters=off  BreakLoop=off  DataType=off  TransfoNumber=1
  T_191841753__ПС_Свияжск : powerlib/Elements/Three-Phase Transformer (Two Windings)  Winding1Connection=Yg  UNITS=pu  NominalPower=[ 250e6 , 60 ]  Winding1=[110000,0.002,0.08]  Winding2Connection=Yg  Winding2=[110000,0.002,0.08]  SetSaturation=off  Rm=500  Lm=500  Saturation=[ 0,0 ; 0.0024,1.2 ; 1.0,1.52 ]  Hysteresis=off  DataFile='hysteresis'  SetInitialFlux=off  InitialFluxes=[ 0.8 , -0.8 , 0.7 ]  Measurements=None  MoreParameters=off  BreakLoop=off  DataType=off  TransfoNumber=1
  T_192426717_110000_ПС_Люзень : powerlib/Elements/Three-Phase Transformer (Two Windings)  Winding1Connection=Yg  UNITS=pu  NominalPower=[ 250e6 , 60 ]  Winding1=[110000,0.002,0.08]  Winding2Connection=Yg  Winding2=[110000,0.002,0.08]  SetSaturation=off  Rm=500  Lm=500  Saturation=[ 0,0 ; 0.0024,1.2 ; 1.0,1.52 ]  Hysteresis=off  DataFile='hysteresis'  SetInitialFlux=off  InitialFluxes=[ 0.8 , -0.8 , 0.7 ]  Measurements=None  MoreParameters=off  BreakLoop=off  DataType=off  TransfoNumber=1
  T_192432406__ : powerlib/Elements/Three-Phase Transformer (Two Windings)  Winding1Connection=Yg  UNITS=pu  NominalPower=[ 250e6 , 60 ]  Winding1=[110000,0.002,0.08]  Winding2Connection=Yg  Winding2=[110000,0.002,0.08]  SetSaturation=off  Rm=500  Lm=500  Saturation=[ 0,0 ; 0.0024,1.2 ; 1.0,1.52 ]  Hysteresis=off  DataFile='hysteresis'  SetInitialFlux=off  InitialFluxes=[ 0.8 , -0.8 , 0.7 ]  Measurements=None  MoreParameters=off  BreakLoop=off  DataType=off  TransfoNumber=1
  T_192432407__ : powerlib/Elements/Three-Phase Transformer (Two Windings)  Winding1Connection=Yg  UNITS=pu  NominalPower=[ 250e6 , 60 ]  Winding1=[110000,0.002,0.08]  Winding2Connection=Yg  Winding2=[110000,0.002,0.08]  SetSaturation=off  Rm=500  Lm=500  Saturation=[ 0,0 ; 0.0024,1.2 ; 1.0,1.52 ]  Hysteresis=off  DataFile='hysteresis'  SetInitialFlux=off  InitialFluxes=[ 0.8 , -0.8 , 0.7 ]  Measurements=None  MoreParameters=off  BreakLoop=off  DataType=off  TransfoNumber=1
  T_193513250__ : powerlib/Elements/Three-Phase Transformer (Two Windings)  Winding1Connection=Yg  UNITS=pu  NominalPower=[ 250e6 , 60 ]  Winding1=[500000,0.002,0.08]  Winding2Connection=Yg  Winding2=[500000,0.002,0.08]  SetSaturation=off  Rm=500  Lm=500  Saturation=[ 0,0 ; 0.0024,1.2 ; 1.0,1.52 ]  Hysteresis=off  DataFile='hysteresis'  SetInitialFlux=off  InitialFluxes=[ 0.8 , -0.8 , 0.7 ]  Measurements=None  MoreParameters=off  BreakLoop=off  DataType=off  TransfoNumber=1
  T_193928464__ПС_КПД : powerlib/Elements/Three-Phase Transformer (Two Windings)  Winding1Connection=Yg  UNITS=pu  NominalPower=[ 250e6 , 60 ]  Winding1=[110000,0.002,0.08]  Winding2Connection=Yg  Winding2=[110000,0.002,0.08]  SetSaturation=off  Rm=500  Lm=500  Saturation=[ 0,0 ; 0.0024,1.2 ; 1.0,1.52 ]  Hysteresis=off  DataFile='hysteresis'  SetInitialFlux=off  InitialFluxes=[ 0.8 , -0.8 , 0.7 ]  Measurements=None  MoreParameters=off  BreakLoop=off  DataType=off  TransfoNumber=1
  T_194431022_110000;35000;10000_ПС_110_35_10_кВ_Яльчики : powerlib/Elements/Three-Phase Transformer (Two Windings)  Winding1Connection=Yg  UNITS=pu  NominalPower=[ 250e6 , 60 ]  Winding1=[110000,0.002,0.08]  Winding2Connection=Yg  Winding2=[110000,0.002,0.08]  SetSaturation=off  Rm=500  Lm=500  Saturation=[ 0,0 ; 0.0024,1.2 ; 1.0,1.52 ]  Hysteresis=off  DataFile='hysteresis'  SetInitialFlux=off  InitialFluxes=[ 0.8 , -0.8 , 0.7 ]  Measurements=None  MoreParameters=off  BreakLoop=off  DataType=off  TransfoNumber=1
  T_197887411_110000;35000;10000_ПС_110_35_10_кВ_Атлашево : powerlib/Elements/Three-Phase Transformer (Two Windings)  Winding1Connection=Yg  UNITS=pu  NominalPower=[ 250e6 , 60 ]  Winding1=[110000,0.002,0.08]  Winding2Connection=Yg  Winding2=[110000,0.002,0.08]  SetSaturation=off  Rm=500  Lm=500  Saturation=[ 0,0 ; 0.0024,1.2 ; 1.0,1.52 ]  Hysteresis=off  DataFile='hysteresis'  SetInitialFlux=off  InitialFluxes=[ 0.8 , -0.8 , 0.7 ]  Measurements=None  MoreParameters=off  BreakLoop=off  DataType=off  TransfoNumber=1
  T_198002186_110000;10000_ПС_110_10_кВ_Бройлерная : powerlib/Elements/Three-Phase Transformer (Two Windings)  Winding1Connection=Yg  UNITS=pu  NominalPower=[ 250e6 , 60 ]  Winding1=[110000,0.002,0.08]  Winding2Connection=Yg  Winding2=[110000,0.002,0.08]  SetSaturation=off  Rm=500  Lm=500  Saturation=[ 0,0 ; 0.0024,1.2 ; 1.0,1.52 ]  Hysteresis=off  DataFile='hysteresis'  SetInitialFlux=off  InitialFluxes=[ 0.8 , -0.8 , 0.7 ]  Measurements=None  MoreParameters=off  BreakLoop=off  DataType=off  TransfoNumber=1
  T_207204995_220000;110000;6000_ПС_Венец_220_110_6_кВ : powerlib/Elements/Three-Phase Transformer (Two Windings)  Winding1Connection=Yg  UNITS=pu  NominalPower=[ 250e6 , 60 ]  Winding1=[220000,0.002,0.08]  Winding2Connection=Yg  Winding2=[110000,0.002,0.08]  SetSaturation=off  Rm=500  Lm=500  Saturation=[ 0,0 ; 0.0024,1.2 ; 1.0,1.52 ]  Hysteresis=off  DataFile='hysteresis'  SetInitialFlux=off  InitialFluxes=[ 0.8 , -0.8 , 0.7 ]  Measurements=None  MoreParameters=off  BreakLoop=off  DataType=off  TransfoNumber=1
  T_207206840__Тяговая_подстанция : powerlib/Elements/Three-Phase Transformer (Two Windings)  Winding1Connection=Yg  UNITS=pu  NominalPower=[ 250e6 , 60 ]  Winding1=[110000,0.002,0.08]  Winding2Connection=Yg  Winding2=[110000,0.002,0.08]  SetSaturation=off  Rm=500  Lm=500  Saturation=[ 0,0 ; 0.0024,1.2 ; 1.0,1.52 ]  Hysteresis=off  DataFile='hysteresis'  SetInitialFlux=off  InitialFluxes=[ 0.8 , -0.8 , 0.7 ]  Measurements=None  MoreParameters=off  BreakLoop=off  DataType=off  TransfoNumber=1
  T_207740804_110000;10000_ПС_110_10_кВ_Дружба : powerlib/Elements/Three-Phase Transformer (Two Windings)  Winding1Connection=Yg  UNITS=pu  NominalPower=[ 250e6 , 60 ]  Winding1=[110000,0.002,0.08]  Winding2Connection=Yg  Winding2=[110000,0.002,0.08]  SetSaturation=off  Rm=500  Lm=500  Saturation=[ 0,0 ; 0.0024,1.2 ; 1.0,1.52 ]  Hysteresis=off  DataFile='hysteresis'  SetInitialFlux=off  InitialFluxes=[ 0.8 , -0.8 , 0.7 ]  Measurements=None  MoreParameters=off  BreakLoop=off  DataType=off  TransfoNumber=1
  T_208425687_110000;35000;10000_ПС_110_35_10_кВ_Комсомольская : powerlib/Elements/Three-Phase Transformer (Two Windings)  Winding1Connection=Yg  UNITS=pu  NominalPower=[ 250e6 , 60 ]  Winding1=[110000,0.002,0.08]  Winding2Connection=Yg  Winding2=[110000,0.002,0.08]  SetSaturation=off  Rm=500  Lm=500  Saturation=[ 0,0 ; 0.0024,1.2 ; 1.0,1.52 ]  Hysteresis=off  DataFile='hysteresis'  SetInitialFlux=off  InitialFluxes=[ 0.8 , -0.8 , 0.7 ]  Measurements=None  MoreParameters=off  BreakLoop=off  DataType=off  TransfoNumber=1
  T_211405161_220000_Пенза_1 : powerlib/Elements/Three-Phase Transformer (Two Windings)  Winding1Connection=Yg  UNITS=pu  NominalPower=[ 250e6 , 60 ]  Winding1=[220000,0.002,0.08]  Winding2Connection=Yg  Winding2=[220000,0.002,0.08]  SetSaturation=off  Rm=500  Lm=500  Saturation=[ 0,0 ; 0.0024,1.2 ; 1.0,1.52 ]  Hysteresis=off  DataFile='hysteresis'  SetInitialFlux=off  InitialFluxes=[ 0.8 , -0.8 , 0.7 ]  Measurements=None  MoreParameters=off  BreakLoop=off  DataType=off  TransfoNumber=1
  T_211578632_110000_ПС_СИЛЬВИНИТ : powerlib/Elements/Three-Phase Transformer (Two Windings)  Winding1Connection=Yg  UNITS=pu  NominalPower=[ 250e6 , 60 ]  Winding1=[110000,0.002,0.08]  Winding2Connection=Yg  Winding2=[110000,0.002,0.08]  SetSaturation=off  Rm=500  Lm=500  Saturation=[ 0,0 ; 0.0024,1.2 ; 1.0,1.52 ]  Hysteresis=off  DataFile='hysteresis'  SetInitialFlux=off  InitialFluxes=[ 0.8 , -0.8 , 0.7 ]  Measurements=None  MoreParameters=off  BreakLoop=off  DataType=off  TransfoNumber=1
  T_218733056__ : powerlib/Elements/Three-Phase Transformer (Two Windings)  Winding1Connection=Yg  UNITS=pu  NominalPower=[ 250e6 , 60 ]  Winding1=[110000,0.002,0.08]  Winding2Connection=Yg  Winding2=[110000,0.002,0.08]  SetSaturation=off  Rm=500  Lm=500  Saturation=[ 0,0 ; 0.0024,1.2 ; 1.0,1.52 ]  Hysteresis=off  DataFile='hysteresis'  SetInitialFlux=off  InitialFluxes=[ 0.8 , -0.8 , 0.7 ]  Measurements=None  MoreParameters=off  BreakLoop=off  DataType=off  TransfoNumber=1
  T_218733818__ : powerlib/Elements/Three-Phase Transformer (Two Windings)  Winding1Connection=Yg  UNITS=pu  NominalPower=[ 250e6 , 60 ]  Winding1=[110000,0.002,0.08]  Winding2Connection=Yg  Winding2=[110000,0.002,0.08]  SetSaturation=off  Rm=500  Lm=500  Saturation=[ 0,0 ; 0.0024,1.2 ; 1.0,1.52 ]  Hysteresis=off  DataFile='hysteresis'  SetInitialFlux=off  InitialFluxes=[ 0.8 , -0.8 , 0.7 ]  Measurements=None  MoreParameters=off  BreakLoop=off  DataType=off  TransfoNumber=1
  T_218733820__ : powerlib/Elements/Three-Phase Transformer (Two Windings)  Winding1Connection=Yg  UNITS=pu  NominalPower=[ 250e6 , 60 ]  Winding1=[110000,0.002,0.08]  Winding2Connection=Yg  Winding2=[110000,0.002,0.08]  SetSaturation=off  Rm=500  Lm=500  Saturation=[ 0,0 ; 0.0024,1.2 ; 1.0,1.52 ]  Hysteresis=off  DataFile='hysteresis'  SetInitialFlux=off  InitialFluxes=[ 0.8 , -0.8 , 0.7 ]  Measurements=None  MoreParameters=off  BreakLoop=off  DataType=off  TransfoNumber=1
  T_219112646__ : powerlib/Elements/Three-Phase Transformer (Two Windings)  Winding1Connection=Yg  UNITS=pu  NominalPower=[ 250e6 , 60 ]  Winding1=[500000,0.002,0.08]  Winding2Connection=Yg  Winding2=[500000,0.002,0.08]  SetSaturation=off  Rm=500  Lm=500  Saturation=[ 0,0 ; 0.0024,1.2 ; 1.0,1.52 ]  Hysteresis=off  DataFile='hysteresis'  SetInitialFlux=off  InitialFluxes=[ 0.8 , -0.8 , 0.7 ]  Measurements=None  MoreParameters=off  BreakLoop=off  DataType=off  TransfoNumber=1
  T_219655813_500000;220000;110000_ПС_Буйская : powerlib/Elements/Three-Phase Transformer (Two Windings)  Winding1Connection=Yg  UNITS=pu  NominalPower=[ 250e6 , 60 ]  Winding1=[500000,0.002,0.08]  Winding2Connection=Yg  Winding2=[500000,0.002,0.08]  SetSaturation=off  Rm=500  Lm=500  Saturation=[ 0,0 ; 0.0024,1.2 ; 1.0,1.52 ]  Hysteresis=off  DataFile='hysteresis'  SetInitialFlux=off  InitialFluxes=[ 0.8 , -0.8 , 0.7 ]  Measurements=None  MoreParameters=off  BreakLoop=off  DataType=off  TransfoNumber=1
  T_219889824_110000;35000;6000_ПС_110_35_6_кВ_Алатырь : powerlib/Elements/Three-Phase Transformer (Two Windings)  Winding1Connection=Yg  UNITS=pu  NominalPower=[ 250e6 , 60 ]  Winding1=[110000,0.002,0.08]  Winding2Connection=Yg  Winding2=[110000,0.002,0.08]  SetSaturation=off  Rm=500  Lm=500  Saturation=[ 0,0 ; 0.0024,1.2 ; 1.0,1.52 ]  Hysteresis=off  DataFile='hysteresis'  SetInitialFlux=off  InitialFluxes=[ 0.8 , -0.8 , 0.7 ]  Measurements=None  MoreParameters=off  BreakLoop=off  DataType=off  TransfoNumber=1
  T_222133214_110000;10000_ПС_110_10_кВ_Семеновская : powerlib/Elements/Three-Phase Transformer (Two Windings)  Winding1Connection=Yg  UNITS=pu  NominalPower=[ 250e6 , 60 ]  Winding1=[110000,0.002,0.08]  Winding2Connection=Yg  Winding2=[110000,0.002,0.08]  SetSaturation=off  Rm=500  Lm=500  Saturation=[ 0,0 ; 0.0024,1.2 ; 1.0,1.52 ]  Hysteresis=off  DataFile='hysteresis'  SetInitialFlux=off  InitialFluxes=[ 0.8 , -0.8 , 0.7 ]  Measurements=None  MoreParameters=off  BreakLoop=off  DataType=off  TransfoNumber=1
  T_224208787_220000_ПС_Дубники : powerlib/Elements/Three-Phase Transformer (Two Windings)  Winding1Connection=Yg  UNITS=pu  NominalPower=[ 250e6 , 60 ]  Winding1=[220000,0.002,0.08]  Winding2Connection=Yg  Winding2=[220000,0.002,0.08]  SetSaturation=off  Rm=500  Lm=500  Saturation=[ 0,0 ; 0.0024,1.2 ; 1.0,1.52 ]  Hysteresis=off  DataFile='hysteresis'  SetInitialFlux=off  InitialFluxes=[ 0.8 , -0.8 , 0.7 ]  Measurements=None  MoreParameters=off  BreakLoop=off  DataType=off  TransfoNumber=1
  T_224261932__Аткарская : powerlib/Elements/Three-Phase Transformer (Two Windings)  Winding1Connection=Yg  UNITS=pu  NominalPower=[ 250e6 , 60 ]  Winding1=[220000,0.002,0.08]  Winding2Connection=Yg  Winding2=[220000,0.002,0.08]  SetSaturation=off  Rm=500  Lm=500  Saturation=[ 0,0 ; 0.0024,1.2 ; 1.0,1.52 ]  Hysteresis=off  DataFile='hysteresis'  SetInitialFlux=off  InitialFluxes=[ 0.8 , -0.8 , 0.7 ]  Measurements=None  MoreParameters=off  BreakLoop=off  DataType=off  TransfoNumber=1
  T_226052064_110000;10000_ПС_110_10_кВ_Шоркистры : powerlib/Elements/Three-Phase Transformer (Two Windings)  Winding1Connection=Yg  UNITS=pu  NominalPower=[ 250e6 , 60 ]  Winding1=[110000,0.002,0.08]  Winding2Connection=Yg  Winding2=[110000,0.002,0.08]  SetSaturation=off  Rm=500  Lm=500  Saturation=[ 0,0 ; 0.0024,1.2 ; 1.0,1.52 ]  Hysteresis=off  DataFile='hysteresis'  SetInitialFlux=off  InitialFluxes=[ 0.8 , -0.8 , 0.7 ]  Measurements=None  MoreParameters=off  BreakLoop=off  DataType=off  TransfoNumber=1
  T_226054226_110000;10000_ПС_110_10_кВ_Кибечи : powerlib/Elements/Three-Phase Transformer (Two Windings)  Winding1Connection=Yg  UNITS=pu  NominalPower=[ 250e6 , 60 ]  Winding1=[110000,0.002,0.08]  Winding2Connection=Yg  Winding2=[110000,0.002,0.08]  SetSaturation=off  Rm=500  Lm=500  Saturation=[ 0,0 ; 0.0024,1.2 ; 1.0,1.52 ]  Hysteresis=off  DataFile='hysteresis'  SetInitialFlux=off  InitialFluxes=[ 0.8 , -0.8 , 0.7 ]  Measurements=None  MoreParameters=off  BreakLoop=off  DataType=off  TransfoNumber=1
  T_226055229_110000;10000_ПС_110_10_кВ_Козловка : powerlib/Elements/Three-Phase Transformer (Two Windings)  Winding1Connection=Yg  UNITS=pu  NominalPower=[ 250e6 , 60 ]  Winding1=[110000,0.002,0.08]  Winding2Connection=Yg  Winding2=[110000,0.002,0.08]  SetSaturation=off  Rm=500  Lm=500  Saturation=[ 0,0 ; 0.0024,1.2 ; 1.0,1.52 ]  Hysteresis=off  DataFile='hysteresis'  SetInitialFlux=off  InitialFluxes=[ 0.8 , -0.8 , 0.7 ]  Measurements=None  MoreParameters=off  BreakLoop=off  DataType=off  TransfoNumber=1
  T_226055643__ : powerlib/Elements/Three-Phase Transformer (Two Windings)  Winding1Connection=Yg  UNITS=pu  NominalPower=[ 250e6 , 60 ]  Winding1=[110000,0.002,0.08]  Winding2Connection=Yg  Winding2=[110000,0.002,0.08]  SetSaturation=off  Rm=500  Lm=500  Saturation=[ 0,0 ; 0.0024,1.2 ; 1.0,1.52 ]  Hysteresis=off  DataFile='hysteresis'  SetInitialFlux=off  InitialFluxes=[ 0.8 , -0.8 , 0.7 ]  Measurements=None  MoreParameters=off  BreakLoop=off  DataType=off  TransfoNumber=1
  T_227673096_110000;10000_ПС_110_10кВ_Алтышево : powerlib/Elements/Three-Phase Transformer (Two Windings)  Winding1Connection=Yg  UNITS=pu  NominalPower=[ 250e6 , 60 ]  Winding1=[110000,0.002,0.08]  Winding2Connection=Yg  Winding2=[110000,0.002,0.08]  SetSaturation=off  Rm=500  Lm=500  Saturation=[ 0,0 ; 0.0024,1.2 ; 1.0,1.52 ]  Hysteresis=off  DataFile='hysteresis'  SetInitialFlux=off  InitialFluxes=[ 0.8 , -0.8 , 0.7 ]  Measurements=None  MoreParameters=off  BreakLoop=off  DataType=off  TransfoNumber=1
  T_227835712_500000;220000_ПС_500_кВ_Красноармейская : powerlib/Elements/Three-Phase Transformer (Two Windings)  Winding1Connection=Yg  UNITS=pu  NominalPower=[ 250e6 , 60 ]  Winding1=[500000,0.002,0.08]  Winding2Connection=Yg  Winding2=[500000,0.002,0.08]  SetSaturation=off  Rm=500  Lm=500  Saturation=[ 0,0 ; 0.0024,1.2 ; 1.0,1.52 ]  Hysteresis=off  DataFile='hysteresis'  SetInitialFlux=off  InitialFluxes=[ 0.8 , -0.8 , 0.7 ]  Measurements=None  MoreParameters=off  BreakLoop=off  DataType=off  TransfoNumber=1
  T_229649869_500000_ПС_500_кВ_Удмуртская : powerlib/Elements/Three-Phase Transformer (Two Windings)  Winding1Connection=Yg  UNITS=pu  NominalPower=[ 250e6 , 60 ]  Winding1=[500000,0.002,0.08]  Winding2Connection=Yg  Winding2=[500000,0.002,0.08]  SetSaturation=off  Rm=500  Lm=500  Saturation=[ 0,0 ; 0.0024,1.2 ; 1.0,1.52 ]  Hysteresis=off  DataFile='hysteresis'  SetInitialFlux=off  InitialFluxes=[ 0.8 , -0.8 , 0.7 ]  Measurements=None  MoreParameters=off  BreakLoop=off  DataType=off  TransfoNumber=1
  T_229841888__ПС_Нурлаты : powerlib/Elements/Three-Phase Transformer (Two Windings)  Winding1Connection=Yg  UNITS=pu  NominalPower=[ 250e6 , 60 ]  Winding1=[110000,0.002,0.08]  Winding2Connection=Yg  Winding2=[110000,0.002,0.08]  SetSaturation=off  Rm=500  Lm=500  Saturation=[ 0,0 ; 0.0024,1.2 ; 1.0,1.52 ]  Hysteresis=off  DataFile='hysteresis'  SetInitialFlux=off  InitialFluxes=[ 0.8 , -0.8 , 0.7 ]  Measurements=None  MoreParameters=off  BreakLoop=off  DataType=off  TransfoNumber=1
  T_229942593__ : powerlib/Elements/Three-Phase Transformer (Two Windings)  Winding1Connection=Yg  UNITS=pu  NominalPower=[ 250e6 , 60 ]  Winding1=[220000,0.002,0.08]  Winding2Connection=Yg  Winding2=[220000,0.002,0.08]  SetSaturation=off  Rm=500  Lm=500  Saturation=[ 0,0 ; 0.0024,1.2 ; 1.0,1.52 ]  Hysteresis=off  DataFile='hysteresis'  SetInitialFlux=off  InitialFluxes=[ 0.8 , -0.8 , 0.7 ]  Measurements=None  MoreParameters=off  BreakLoop=off  DataType=off  TransfoNumber=1
  T_232164616__ : powerlib/Elements/Three-Phase Transformer (Two Windings)  Winding1Connection=Yg  UNITS=pu  NominalPower=[ 250e6 , 60 ]  Winding1=[220000,0.002,0.08]  Winding2Connection=Yg  Winding2=[220000,0.002,0.08]  SetSaturation=off  Rm=500  Lm=500  Saturation=[ 0,0 ; 0.0024,1.2 ; 1.0,1.52 ]  Hysteresis=off  DataFile='hysteresis'  SetInitialFlux=off  InitialFluxes=[ 0.8 , -0.8 , 0.7 ]  Measurements=None  MoreParameters=off  BreakLoop=off  DataType=off  TransfoNumber=1
  T_234246987_110000;10000_ПС_110_10_кВ_Луч : powerlib/Elements/Three-Phase Transformer (Two Windings)  Winding1Connection=Yg  UNITS=pu  NominalPower=[ 250e6 , 60 ]  Winding1=[110000,0.002,0.08]  Winding2Connection=Yg  Winding2=[110000,0.002,0.08]  SetSaturation=off  Rm=500  Lm=500  Saturation=[ 0,0 ; 0.0024,1.2 ; 1.0,1.52 ]  Hysteresis=off  DataFile='hysteresis'  SetInitialFlux=off  InitialFluxes=[ 0.8 , -0.8 , 0.7 ]  Measurements=None  MoreParameters=off  BreakLoop=off  DataType=off  TransfoNumber=1
  T_236703070__ПС_Дубъязы : powerlib/Elements/Three-Phase Transformer (Two Windings)  Winding1Connection=Yg  UNITS=pu  NominalPower=[ 250e6 , 60 ]  Winding1=[110000,0.002,0.08]  Winding2Connection=Yg  Winding2=[110000,0.002,0.08]  SetSaturation=off  Rm=500  Lm=500  Saturation=[ 0,0 ; 0.0024,1.2 ; 1.0,1.52 ]  Hysteresis=off  DataFile='hysteresis'  SetInitialFlux=off  InitialFluxes=[ 0.8 , -0.8 , 0.7 ]  Measurements=None  MoreParameters=off  BreakLoop=off  DataType=off  TransfoNumber=1
  T_238317576__ : powerlib/Elements/Three-Phase Transformer (Two Windings)  Winding1Connection=Yg  UNITS=pu  NominalPower=[ 250e6 , 60 ]  Winding1=[110000,0.002,0.08]  Winding2Connection=Yg  Winding2=[110000,0.002,0.08]  SetSaturation=off  Rm=500  Lm=500  Saturation=[ 0,0 ; 0.0024,1.2 ; 1.0,1.52 ]  Hysteresis=off  DataFile='hysteresis'  SetInitialFlux=off  InitialFluxes=[ 0.8 , -0.8 , 0.7 ]  Measurements=None  MoreParameters=off  BreakLoop=off  DataType=off  TransfoNumber=1
  T_238549570__ПС_Алкино : powerlib/Elements/Three-Phase Transformer (Two Windings)  Winding1Connection=Yg  UNITS=pu  NominalPower=[ 250e6 , 60 ]  Winding1=[110000,0.002,0.08]  Winding2Connection=Yg  Winding2=[110000,0.002,0.08]  SetSaturation=off  Rm=500  Lm=500  Saturation=[ 0,0 ; 0.0024,1.2 ; 1.0,1.52 ]  Hysteresis=off  DataFile='hysteresis'  SetInitialFlux=off  InitialFluxes=[ 0.8 , -0.8 , 0.7 ]  Measurements=None  MoreParameters=off  BreakLoop=off  DataType=off  TransfoNumber=1
  T_240018999__ : powerlib/Elements/Three-Phase Transformer (Two Windings)  Winding1Connection=Yg  UNITS=pu  NominalPower=[ 250e6 , 60 ]  Winding1=[220000,0.002,0.08]  Winding2Connection=Yg  Winding2=[220000,0.002,0.08]  SetSaturation=off  Rm=500  Lm=500  Saturation=[ 0,0 ; 0.0024,1.2 ; 1.0,1.52 ]  Hysteresis=off  DataFile='hysteresis'  SetInitialFlux=off  InitialFluxes=[ 0.8 , -0.8 , 0.7 ]  Measurements=None  MoreParameters=off  BreakLoop=off  DataType=off  TransfoNumber=1
  T_241262030_110000;35000;10000_ПС_110_35_10_кВ_Цивильск : powerlib/Elements/Three-Phase Transformer (Two Windings)  Winding1Connection=Yg  UNITS=pu  NominalPower=[ 250e6 , 60 ]  Winding1=[110000,0.002,0.08]  Winding2Connection=Yg  Winding2=[110000,0.002,0.08]  SetSaturation=off  Rm=500  Lm=500  Saturation=[ 0,0 ; 0.0024,1.2 ; 1.0,1.52 ]  Hysteresis=off  DataFile='hysteresis'  SetInitialFlux=off  InitialFluxes=[ 0.8 , -0.8 , 0.7 ]  Measurements=None  MoreParameters=off  BreakLoop=off  DataType=off  TransfoNumber=1
  T_242610017_110000;35000;10000_ПС_110_35_10_кВ_Лесная : powerlib/Elements/Three-Phase Transformer (Two Windings)  Winding1Connection=Yg  UNITS=pu  NominalPower=[ 250e6 , 60 ]  Winding1=[110000,0.002,0.08]  Winding2Connection=Yg  Winding2=[110000,0.002,0.08]  SetSaturation=off  Rm=500  Lm=500  Saturation=[ 0,0 ; 0.0024,1.2 ; 1.0,1.52 ]  Hysteresis=off  DataFile='hysteresis'  SetInitialFlux=off  InitialFluxes=[ 0.8 , -0.8 , 0.7 ]  Measurements=None  MoreParameters=off  BreakLoop=off  DataType=off  TransfoNumber=1
  T_242614771_110000;6000_ПС_110_6_кВ_Тормозная : powerlib/Elements/Three-Phase Transformer (Two Windings)  Winding1Connection=Yg  UNITS=pu  NominalPower=[ 250e6 , 60 ]  Winding1=[110000,0.002,0.08]  Winding2Connection=Yg  Winding2=[110000,0.002,0.08]  SetSaturation=off  Rm=500  Lm=500  Saturation=[ 0,0 ; 0.0024,1.2 ; 1.0,1.52 ]  Hysteresis=off  DataFile='hysteresis'  SetInitialFlux=off  InitialFluxes=[ 0.8 , -0.8 , 0.7 ]  Measurements=None  MoreParameters=off  BreakLoop=off  DataType=off  TransfoNumber=1
  T_242619649_110000;10000_ПС_110_10_кВ_Чагаси : powerlib/Elements/Three-Phase Transformer (Two Windings)  Winding1Connection=Yg  UNITS=pu  NominalPower=[ 250e6 , 60 ]  Winding1=[110000,0.002,0.08]  Winding2Connection=Yg  Winding2=[110000,0.002,0.08]  SetSaturation=off  Rm=500  Lm=500  Saturation=[ 0,0 ; 0.0024,1.2 ; 1.0,1.52 ]  Hysteresis=off  DataFile='hysteresis'  SetInitialFlux=off  InitialFluxes=[ 0.8 , -0.8 , 0.7 ]  Measurements=None  MoreParameters=off  BreakLoop=off  DataType=off  TransfoNumber=1
  T_242932802_110000;10000_ПС_110_10_кВ_Оросительная : powerlib/Elements/Three-Phase Transformer (Two Windings)  Winding1Connection=Yg  UNITS=pu  NominalPower=[ 250e6 , 60 ]  Winding1=[110000,0.002,0.08]  Winding2Connection=Yg  Winding2=[110000,0.002,0.08]  SetSaturation=off  Rm=500  Lm=500  Saturation=[ 0,0 ; 0.0024,1.2 ; 1.0,1.52 ]  Hysteresis=off  DataFile='hysteresis'  SetInitialFlux=off  InitialFluxes=[ 0.8 , -0.8 , 0.7 ]  Measurements=None  MoreParameters=off  BreakLoop=off  DataType=off  TransfoNumber=1
  T_242972920_110000;10000_ПС_110_10_кВ_Заволжская : powerlib/Elements/Three-Phase Transformer (Two Windings)  Winding1Connection=Yg  UNITS=pu  NominalPower=[ 250e6 , 60 ]  Winding1=[110000,0.002,0.08]  Winding2Connection=Yg  Winding2=[110000,0.002,0.08]  SetSaturation=off  Rm=500  Lm=500  Saturation=[ 0,0 ; 0.0024,1.2 ; 1.0,1.52 ]  Hysteresis=off  DataFile='hysteresis'  SetInitialFlux=off  InitialFluxes=[ 0.8 , -0.8 , 0.7 ]  Measurements=None  MoreParameters=off  BreakLoop=off  DataType=off  TransfoNumber=1
  T_242973735_110000;10000_ПС_110_10_кВ_Яндоба : powerlib/Elements/Three-Phase Transformer (Two Windings)  Winding1Connection=Yg  UNITS=pu  NominalPower=[ 250e6 , 60 ]  Winding1=[110000,0.002,0.08]  Winding2Connection=Yg  Winding2=[110000,0.002,0.08]  SetSaturation=off  Rm=500  Lm=500  Saturation=[ 0,0 ; 0.0024,1.2 ; 1.0,1.52 ]  Hysteresis=off  DataFile='hysteresis'  SetInitialFlux=off  InitialFluxes=[ 0.8 , -0.8 , 0.7 ]  Measurements=None  MoreParameters=off  BreakLoop=off  DataType=off  TransfoNumber=1
  T_243068515_110000;10000_ПС_110_10_кВ_Маяк : powerlib/Elements/Three-Phase Transformer (Two Windings)  Winding1Connection=Yg  UNITS=pu  NominalPower=[ 250e6 , 60 ]  Winding1=[110000,0.002,0.08]  Winding2Connection=Yg  Winding2=[110000,0.002,0.08]  SetSaturation=off  Rm=500  Lm=500  Saturation=[ 0,0 ; 0.0024,1.2 ; 1.0,1.52 ]  Hysteresis=off  DataFile='hysteresis'  SetInitialFlux=off  InitialFluxes=[ 0.8 , -0.8 , 0.7 ]  Measurements=None  MoreParameters=off  BreakLoop=off  DataType=off  TransfoNumber=1
  T_243069892_110000;35000;10000_ПС_110_35_10_кВ_Урмары : powerlib/Elements/Three-Phase Transformer (Two Windings)  Winding1Connection=Yg  UNITS=pu  NominalPower=[ 250e6 , 60 ]  Winding1=[110000,0.002,0.08]  Winding2Connection=Yg  Winding2=[110000,0.002,0.08]  SetSaturation=off  Rm=500  Lm=500  Saturation=[ 0,0 ; 0.0024,1.2 ; 1.0,1.52 ]  Hysteresis=off  DataFile='hysteresis'  SetInitialFlux=off  InitialFluxes=[ 0.8 , -0.8 , 0.7 ]  Measurements=None  MoreParameters=off  BreakLoop=off  DataType=off  TransfoNumber=1
  T_243075861_110000;6000_ПС_110_6_кВ_Южная : powerlib/Elements/Three-Phase Transformer (Two Windings)  Winding1Connection=Yg  UNITS=pu  NominalPower=[ 250e6 , 60 ]  Winding1=[110000,0.002,0.08]  Winding2Connection=Yg  Winding2=[110000,0.002,0.08]  SetSaturation=off  Rm=500  Lm=500  Saturation=[ 0,0 ; 0.0024,1.2 ; 1.0,1.52 ]  Hysteresis=off  DataFile='hysteresis'  SetInitialFlux=off  InitialFluxes=[ 0.8 , -0.8 , 0.7 ]  Measurements=None  MoreParameters=off  BreakLoop=off  DataType=off  TransfoNumber=1
  T_243154612__ : powerlib/Elements/Three-Phase Transformer (Two Windings)  Winding1Connection=Yg  UNITS=pu  NominalPower=[ 250e6 , 60 ]  Winding1=[110000,0.002,0.08]  Winding2Connection=Yg  Winding2=[110000,0.002,0.08]  SetSaturation=off  Rm=500  Lm=500  Saturation=[ 0,0 ; 0.0024,1.2 ; 1.0,1.52 ]  Hysteresis=off  DataFile='hysteresis'  SetInitialFlux=off  InitialFluxes=[ 0.8 , -0.8 , 0.7 ]  Measurements=None  MoreParameters=off  BreakLoop=off  DataType=off  TransfoNumber=1
  T_243531233__ПС_Малмыж : powerlib/Elements/Three-Phase Transformer (Two Windings)  Winding1Connection=Yg  UNITS=pu  NominalPower=[ 250e6 , 60 ]  Winding1=[110000,0.002,0.08]  Winding2Connection=Yg  Winding2=[110000,0.002,0.08]  SetSaturation=off  Rm=500  Lm=500  Saturation=[ 0,0 ; 0.0024,1.2 ; 1.0,1.52 ]  Hysteresis=off  DataFile='hysteresis'  SetInitialFlux=off  InitialFluxes=[ 0.8 , -0.8 , 0.7 ]  Measurements=None  MoreParameters=off  BreakLoop=off  DataType=off  TransfoNumber=1
  T_243820930__ : powerlib/Elements/Three-Phase Transformer (Two Windings)  Winding1Connection=Yg  UNITS=pu  NominalPower=[ 250e6 , 60 ]  Winding1=[110000,0.002,0.08]  Winding2Connection=Yg  Winding2=[110000,0.002,0.08]  SetSaturation=off  Rm=500  Lm=500  Saturation=[ 0,0 ; 0.0024,1.2 ; 1.0,1.52 ]  Hysteresis=off  DataFile='hysteresis'  SetInitialFlux=off  InitialFluxes=[ 0.8 , -0.8 , 0.7 ]  Measurements=None  MoreParameters=off  BreakLoop=off  DataType=off  TransfoNumber=1
  T_244847744__ : powerlib/Elements/Three-Phase Transformer (Two Windings)  Winding1Connection=Yg  UNITS=pu  NominalPower=[ 250e6 , 60 ]  Winding1=[110000,0.002,0.08]  Winding2Connection=Yg  Winding2=[110000,0.002,0.08]  SetSaturation=off  Rm=500  Lm=500  Saturation=[ 0,0 ; 0.0024,1.2 ; 1.0,1.52 ]  Hysteresis=off  DataFile='hysteresis'  SetInitialFlux=off  InitialFluxes=[ 0.8 , -0.8 , 0.7 ]  Measurements=None  MoreParameters=off  BreakLoop=off  DataType=off  TransfoNumber=1
  T_245404985_110000_ПС_Уньва : powerlib/Elements/Three-Phase Transformer (Two Windings)  Winding1Connection=Yg  UNITS=pu  NominalPower=[ 250e6 , 60 ]  Winding1=[110000,0.002,0.08]  Winding2Connection=Yg  Winding2=[110000,0.002,0.08]  SetSaturation=off  Rm=500  Lm=500  Saturation=[ 0,0 ; 0.0024,1.2 ; 1.0,1.52 ]  Hysteresis=off  DataFile='hysteresis'  SetInitialFlux=off  InitialFluxes=[ 0.8 , -0.8 , 0.7 ]  Measurements=None  MoreParameters=off  BreakLoop=off  DataType=off  TransfoNumber=1
  T_247403714__ПС_Сардек : powerlib/Elements/Three-Phase Transformer (Two Windings)  Winding1Connection=Yg  UNITS=pu  NominalPower=[ 250e6 , 60 ]  Winding1=[110000,0.002,0.08]  Winding2Connection=Yg  Winding2=[110000,0.002,0.08]  SetSaturation=off  Rm=500  Lm=500  Saturation=[ 0,0 ; 0.0024,1.2 ; 1.0,1.52 ]  Hysteresis=off  DataFile='hysteresis'  SetInitialFlux=off  InitialFluxes=[ 0.8 , -0.8 , 0.7 ]  Measurements=None  MoreParameters=off  BreakLoop=off  DataType=off  TransfoNumber=1
  T_250911823__ПС_Б_Матаки : powerlib/Elements/Three-Phase Transformer (Two Windings)  Winding1Connection=Yg  UNITS=pu  NominalPower=[ 250e6 , 60 ]  Winding1=[110000,0.002,0.08]  Winding2Connection=Yg  Winding2=[110000,0.002,0.08]  SetSaturation=off  Rm=500  Lm=500  Saturation=[ 0,0 ; 0.0024,1.2 ; 1.0,1.52 ]  Hysteresis=off  DataFile='hysteresis'  SetInitialFlux=off  InitialFluxes=[ 0.8 , -0.8 , 0.7 ]  Measurements=None  MoreParameters=off  BreakLoop=off  DataType=off  TransfoNumber=1
  T_252815157__ : powerlib/Elements/Three-Phase Transformer (Two Windings)  Winding1Connection=Yg  UNITS=pu  NominalPower=[ 250e6 , 60 ]  Winding1=[110000,0.002,0.08]  Winding2Connection=Yg  Winding2=[110000,0.002,0.08]  SetSaturation=off  Rm=500  Lm=500  Saturation=[ 0,0 ; 0.0024,1.2 ; 1.0,1.52 ]  Hysteresis=off  DataFile='hysteresis'  SetInitialFlux=off  InitialFluxes=[ 0.8 , -0.8 , 0.7 ]  Measurements=None  MoreParameters=off  BreakLoop=off  DataType=off  TransfoNumber=1
  T_252815158_110000;35000;10000_ : powerlib/Elements/Three-Phase Transformer (Two Windings)  Winding1Connection=Yg  UNITS=pu  NominalPower=[ 250e6 , 60 ]  Winding1=[110000,0.002,0.08]  Winding2Connection=Yg  Winding2=[110000,0.002,0.08]  SetSaturation=off  Rm=500  Lm=500  Saturation=[ 0,0 ; 0.0024,1.2 ; 1.0,1.52 ]  Hysteresis=off  DataFile='hysteresis'  SetInitialFlux=off  InitialFluxes=[ 0.8 , -0.8 , 0.7 ]  Measurements=None  MoreParameters=off  BreakLoop=off  DataType=off  TransfoNumber=1
  T_262366241_110000;10000_ПС_110_10_кВ_Сугуты : powerlib/Elements/Three-Phase Transformer (Two Windings)  Winding1Connection=Yg  UNITS=pu  NominalPower=[ 250e6 , 60 ]  Winding1=[110000,0.002,0.08]  Winding2Connection=Yg  Winding2=[110000,0.002,0.08]  SetSaturation=off  Rm=500  Lm=500  Saturation=[ 0,0 ; 0.0024,1.2 ; 1.0,1.52 ]  Hysteresis=off  DataFile='hysteresis'  SetInitialFlux=off  InitialFluxes=[ 0.8 , -0.8 , 0.7 ]  Measurements=None  MoreParameters=off  BreakLoop=off  DataType=off  TransfoNumber=1
  T_262366242_110000;35000;10000_ПС_110_35_10_кВ_Батырево : powerlib/Elements/Three-Phase Transformer (Two Windings)  Winding1Connection=Yg  UNITS=pu  NominalPower=[ 250e6 , 60 ]  Winding1=[110000,0.002,0.08]  Winding2Connection=Yg  Winding2=[110000,0.002,0.08]  SetSaturation=off  Rm=500  Lm=500  Saturation=[ 0,0 ; 0.0024,1.2 ; 1.0,1.52 ]  Hysteresis=off  DataFile='hysteresis'  SetInitialFlux=off  InitialFluxes=[ 0.8 , -0.8 , 0.7 ]  Measurements=None  MoreParameters=off  BreakLoop=off  DataType=off  TransfoNumber=1
  T_274213600_220000_ПС_Студенец : powerlib/Elements/Three-Phase Transformer (Two Windings)  Winding1Connection=Yg  UNITS=pu  NominalPower=[ 250e6 , 60 ]  Winding1=[220000,0.002,0.08]  Winding2Connection=Yg  Winding2=[220000,0.002,0.08]  SetSaturation=off  Rm=500  Lm=500  Saturation=[ 0,0 ; 0.0024,1.2 ; 1.0,1.52 ]  Hysteresis=off  DataFile='hysteresis'  SetInitialFlux=off  InitialFluxes=[ 0.8 , -0.8 , 0.7 ]  Measurements=None  MoreParameters=off  BreakLoop=off  DataType=off  TransfoNumber=1
  T_274937610_220000_ПС_220_кВ_Головная : powerlib/Elements/Three-Phase Transformer (Two Windings)  Winding1Connection=Yg  UNITS=pu  NominalPower=[ 250e6 , 60 ]  Winding1=[220000,0.002,0.08]  Winding2Connection=Yg  Winding2=[220000,0.002,0.08]  SetSaturation=off  Rm=500  Lm=500  Saturation=[ 0,0 ; 0.0024,1.2 ; 1.0,1.52 ]  Hysteresis=off  DataFile='hysteresis'  SetInitialFlux=off  InitialFluxes=[ 0.8 , -0.8 , 0.7 ]  Measurements=None  MoreParameters=off  BreakLoop=off  DataType=off  TransfoNumber=1
  T_274998912_220000_Мокша : powerlib/Elements/Three-Phase Transformer (Two Windings)  Winding1Connection=Yg  UNITS=pu  NominalPower=[ 250e6 , 60 ]  Winding1=[220000,0.002,0.08]  Winding2Connection=Yg  Winding2=[220000,0.002,0.08]  SetSaturation=off  Rm=500  Lm=500  Saturation=[ 0,0 ; 0.0024,1.2 ; 1.0,1.52 ]  Hysteresis=off  DataFile='hysteresis'  SetInitialFlux=off  InitialFluxes=[ 0.8 , -0.8 , 0.7 ]  Measurements=None  MoreParameters=off  BreakLoop=off  DataType=off  TransfoNumber=1
  T_276080500_220000_Комсомольская : powerlib/Elements/Three-Phase Transformer (Two Windings)  Winding1Connection=Yg  UNITS=pu  NominalPower=[ 250e6 , 60 ]  Winding1=[220000,0.002,0.08]  Winding2Connection=Yg  Winding2=[220000,0.002,0.08]  SetSaturation=off  Rm=500  Lm=500  Saturation=[ 0,0 ; 0.0024,1.2 ; 1.0,1.52 ]  Hysteresis=off  DataFile='hysteresis'  SetInitialFlux=off  InitialFluxes=[ 0.8 , -0.8 , 0.7 ]  Measurements=None  MoreParameters=off  BreakLoop=off  DataType=off  TransfoNumber=1
  T_277905349_110000;10000_Андреевка : powerlib/Elements/Three-Phase Transformer (Two Windings)  Winding1Connection=Yg  UNITS=pu  NominalPower=[ 250e6 , 60 ]  Winding1=[110000,0.002,0.08]  Winding2Connection=Yg  Winding2=[110000,0.002,0.08]  SetSaturation=off  Rm=500  Lm=500  Saturation=[ 0,0 ; 0.0024,1.2 ; 1.0,1.52 ]  Hysteresis=off  DataFile='hysteresis'  SetInitialFlux=off  InitialFluxes=[ 0.8 , -0.8 , 0.7 ]  Measurements=None  MoreParameters=off  BreakLoop=off  DataType=off  TransfoNumber=1
  T_277905350_220000;110000_Сергач : powerlib/Elements/Three-Phase Transformer (Two Windings)  Winding1Connection=Yg  UNITS=pu  NominalPower=[ 250e6 , 60 ]  Winding1=[220000,0.002,0.08]  Winding2Connection=Yg  Winding2=[110000,0.002,0.08]  SetSaturation=off  Rm=500  Lm=500  Saturation=[ 0,0 ; 0.0024,1.2 ; 1.0,1.52 ]  Hysteresis=off  DataFile='hysteresis'  SetInitialFlux=off  InitialFluxes=[ 0.8 , -0.8 , 0.7 ]  Measurements=None  MoreParameters=off  BreakLoop=off  DataType=off  TransfoNumber=1
  T_279258960_110000;35000;10000_ПС_110_35_10_кВ_Красноармейская : powerlib/Elements/Three-Phase Transformer (Two Windings)  Winding1Connection=Yg  UNITS=pu  NominalPower=[ 250e6 , 60 ]  Winding1=[110000,0.002,0.08]  Winding2Connection=Yg  Winding2=[110000,0.002,0.08]  SetSaturation=off  Rm=500  Lm=500  Saturation=[ 0,0 ; 0.0024,1.2 ; 1.0,1.52 ]  Hysteresis=off  DataFile='hysteresis'  SetInitialFlux=off  InitialFluxes=[ 0.8 , -0.8 , 0.7 ]  Measurements=None  MoreParameters=off  BreakLoop=off  DataType=off  TransfoNumber=1
  T_279778884_110000;10000_ПС_110_10_кВ_Слава : powerlib/Elements/Three-Phase Transformer (Two Windings)  Winding1Connection=Yg  UNITS=pu  NominalPower=[ 250e6 , 60 ]  Winding1=[110000,0.002,0.08]  Winding2Connection=Yg  Winding2=[110000,0.002,0.08]  SetSaturation=off  Rm=500  Lm=500  Saturation=[ 0,0 ; 0.0024,1.2 ; 1.0,1.52 ]  Hysteresis=off  DataFile='hysteresis'  SetInitialFlux=off  InitialFluxes=[ 0.8 , -0.8 , 0.7 ]  Measurements=None  MoreParameters=off  BreakLoop=off  DataType=off  TransfoNumber=1
  T_279846258_110000;10000_ПС_110_10_кВ_Ачаксы : powerlib/Elements/Three-Phase Transformer (Two Windings)  Winding1Connection=Yg  UNITS=pu  NominalPower=[ 250e6 , 60 ]  Winding1=[110000,0.002,0.08]  Winding2Connection=Yg  Winding2=[110000,0.002,0.08]  SetSaturation=off  Rm=500  Lm=500  Saturation=[ 0,0 ; 0.0024,1.2 ; 1.0,1.52 ]  Hysteresis=off  DataFile='hysteresis'  SetInitialFlux=off  InitialFluxes=[ 0.8 , -0.8 , 0.7 ]  Measurements=None  MoreParameters=off  BreakLoop=off  DataType=off  TransfoNumber=1
  T_279846262_110000;10000_ПС_110_10_кВ_Атнашево : powerlib/Elements/Three-Phase Transformer (Two Windings)  Winding1Connection=Yg  UNITS=pu  NominalPower=[ 250e6 , 60 ]  Winding1=[110000,0.002,0.08]  Winding2Connection=Yg  Winding2=[110000,0.002,0.08]  SetSaturation=off  Rm=500  Lm=500  Saturation=[ 0,0 ; 0.0024,1.2 ; 1.0,1.52 ]  Hysteresis=off  DataFile='hysteresis'  SetInitialFlux=off  InitialFluxes=[ 0.8 , -0.8 , 0.7 ]  Measurements=None  MoreParameters=off  BreakLoop=off  DataType=off  TransfoNumber=1
  T_279919300_110000;35000;10000_ПС_110_35_10_кВ_Шемурша : powerlib/Elements/Three-Phase Transformer (Two Windings)  Winding1Connection=Yg  UNITS=pu  NominalPower=[ 250e6 , 60 ]  Winding1=[110000,0.002,0.08]  Winding2Connection=Yg  Winding2=[110000,0.002,0.08]  SetSaturation=off  Rm=500  Lm=500  Saturation=[ 0,0 ; 0.0024,1.2 ; 1.0,1.52 ]  Hysteresis=off  DataFile='hysteresis'  SetInitialFlux=off  InitialFluxes=[ 0.8 , -0.8 , 0.7 ]  Measurements=None  MoreParameters=off  BreakLoop=off  DataType=off  TransfoNumber=1
  T_279919302_110000;10000_ПС_110_10_кВ_Первомайская : powerlib/Elements/Three-Phase Transformer (Two Windings)  Winding1Connection=Yg  UNITS=pu  NominalPower=[ 250e6 , 60 ]  Winding1=[110000,0.002,0.08]  Winding2Connection=Yg  Winding2=[110000,0.002,0.08]  SetSaturation=off  Rm=500  Lm=500  Saturation=[ 0,0 ; 0.0024,1.2 ; 1.0,1.52 ]  Hysteresis=off  DataFile='hysteresis'  SetInitialFlux=off  InitialFluxes=[ 0.8 , -0.8 , 0.7 ]  Measurements=None  MoreParameters=off  BreakLoop=off  DataType=off  TransfoNumber=1
  T_279978581_110000;10000_ПС_110_10_кВ_Кувакино : powerlib/Elements/Three-Phase Transformer (Two Windings)  Winding1Connection=Yg  UNITS=pu  NominalPower=[ 250e6 , 60 ]  Winding1=[110000,0.002,0.08]  Winding2Connection=Yg  Winding2=[110000,0.002,0.08]  SetSaturation=off  Rm=500  Lm=500  Saturation=[ 0,0 ; 0.0024,1.2 ; 1.0,1.52 ]  Hysteresis=off  DataFile='hysteresis'  SetInitialFlux=off  InitialFluxes=[ 0.8 , -0.8 , 0.7 ]  Measurements=None  MoreParameters=off  BreakLoop=off  DataType=off  TransfoNumber=1
  T_279978582_110000;35000;10000_ПС_110_35_10_кВ_Порецкая : powerlib/Elements/Three-Phase Transformer (Two Windings)  Winding1Connection=Yg  UNITS=pu  NominalPower=[ 250e6 , 60 ]  Winding1=[110000,0.002,0.08]  Winding2Connection=Yg  Winding2=[110000,0.002,0.08]  SetSaturation=off  Rm=500  Lm=500  Saturation=[ 0,0 ; 0.0024,1.2 ; 1.0,1.52 ]  Hysteresis=off  DataFile='hysteresis'  SetInitialFlux=off  InitialFluxes=[ 0.8 , -0.8 , 0.7 ]  Measurements=None  MoreParameters=off  BreakLoop=off  DataType=off  TransfoNumber=1
  T_279978583_110000;10000_ПС_110_10_кВ_Кожевенная : powerlib/Elements/Three-Phase Transformer (Two Windings)  Winding1Connection=Yg  UNITS=pu  NominalPower=[ 250e6 , 60 ]  Winding1=[110000,0.002,0.08]  Winding2Connection=Yg  Winding2=[110000,0.002,0.08]  SetSaturation=off  Rm=500  Lm=500  Saturation=[ 0,0 ; 0.0024,1.2 ; 1.0,1.52 ]  Hysteresis=off  DataFile='hysteresis'  SetInitialFlux=off  InitialFluxes=[ 0.8 , -0.8 , 0.7 ]  Measurements=None  MoreParameters=off  BreakLoop=off  DataType=off  TransfoNumber=1
  T_279978585_110000;10000_ПС_110_10_кВ_Буинск : powerlib/Elements/Three-Phase Transformer (Two Windings)  Winding1Connection=Yg  UNITS=pu  NominalPower=[ 250e6 , 60 ]  Winding1=[110000,0.002,0.08]  Winding2Connection=Yg  Winding2=[110000,0.002,0.08]  SetSaturation=off  Rm=500  Lm=500  Saturation=[ 0,0 ; 0.0024,1.2 ; 1.0,1.52 ]  Hysteresis=off  DataFile='hysteresis'  SetInitialFlux=off  InitialFluxes=[ 0.8 , -0.8 , 0.7 ]  Measurements=None  MoreParameters=off  BreakLoop=off  DataType=off  TransfoNumber=1
  T_279978586_110000;10000_ПС_110_10_кВ_Ибреси : powerlib/Elements/Three-Phase Transformer (Two Windings)  Winding1Connection=Yg  UNITS=pu  NominalPower=[ 250e6 , 60 ]  Winding1=[110000,0.002,0.08]  Winding2Connection=Yg  Winding2=[110000,0.002,0.08]  SetSaturation=off  Rm=500  Lm=500  Saturation=[ 0,0 ; 0.0024,1.2 ; 1.0,1.52 ]  Hysteresis=off  DataFile='hysteresis'  SetInitialFlux=off  InitialFluxes=[ 0.8 , -0.8 , 0.7 ]  Measurements=None  MoreParameters=off  BreakLoop=off  DataType=off  TransfoNumber=1
  T_279978587_110000;10000_ПС_110_10_кВ_Рассвет : powerlib/Elements/Three-Phase Transformer (Two Windings)  Winding1Connection=Yg  UNITS=pu  NominalPower=[ 250e6 , 60 ]  Winding1=[110000,0.002,0.08]  Winding2Connection=Yg  Winding2=[110000,0.002,0.08]  SetSaturation=off  Rm=500  Lm=500  Saturation=[ 0,0 ; 0.0024,1.2 ; 1.0,1.52 ]  Hysteresis=off  DataFile='hysteresis'  SetInitialFlux=off  InitialFluxes=[ 0.8 , -0.8 , 0.7 ]  Measurements=None  MoreParameters=off  BreakLoop=off  DataType=off  TransfoNumber=1
  T_279978588_110000;10000_ПС_110_10_кВ_Алгаши : powerlib/Elements/Three-Phase Transformer (Two Windings)  Winding1Connection=Yg  UNITS=pu  NominalPower=[ 250e6 , 60 ]  Winding1=[110000,0.002,0.08]  Winding2Connection=Yg  Winding2=[110000,0.002,0.08]  SetSaturation=off  Rm=500  Lm=500  Saturation=[ 0,0 ; 0.0024,1.2 ; 1.0,1.52 ]  Hysteresis=off  DataFile='hysteresis'  SetInitialFlux=off  InitialFluxes=[ 0.8 , -0.8 , 0.7 ]  Measurements=None  MoreParameters=off  BreakLoop=off  DataType=off  TransfoNumber=1
  T_280247938__ : powerlib/Elements/Three-Phase Transformer (Two Windings)  Winding1Connection=Yg  UNITS=pu  NominalPower=[ 250e6 , 60 ]  Winding1=[110000,0.002,0.08]  Winding2Connection=Yg  Winding2=[110000,0.002,0.08]  SetSaturation=off  Rm=500  Lm=500  Saturation=[ 0,0 ; 0.0024,1.2 ; 1.0,1.52 ]  Hysteresis=off  DataFile='hysteresis'  SetInitialFlux=off  InitialFluxes=[ 0.8 , -0.8 , 0.7 ]  Measurements=None  MoreParameters=off  BreakLoop=off  DataType=off  TransfoNumber=1
  T_280247940_110000;10000_ПС_110_10_кВ_Саланчики : powerlib/Elements/Three-Phase Transformer (Two Windings)  Winding1Connection=Yg  UNITS=pu  NominalPower=[ 250e6 , 60 ]  Winding1=[110000,0.002,0.08]  Winding2Connection=Yg  Winding2=[110000,0.002,0.08]  SetSaturation=off  Rm=500  Lm=500  Saturation=[ 0,0 ; 0.0024,1.2 ; 1.0,1.52 ]  Hysteresis=off  DataFile='hysteresis'  SetInitialFlux=off  InitialFluxes=[ 0.8 , -0.8 , 0.7 ]  Measurements=None  MoreParameters=off  BreakLoop=off  DataType=off  TransfoNumber=1
  T_280247942_110000;35000;10000_ПС_110_35_10_кВ_Красночетайская : powerlib/Elements/Three-Phase Transformer (Two Windings)  Winding1Connection=Yg  UNITS=pu  NominalPower=[ 250e6 , 60 ]  Winding1=[110000,0.002,0.08]  Winding2Connection=Yg  Winding2=[110000,0.002,0.08]  SetSaturation=off  Rm=500  Lm=500  Saturation=[ 0,0 ; 0.0024,1.2 ; 1.0,1.52 ]  Hysteresis=off  DataFile='hysteresis'  SetInitialFlux=off  InitialFluxes=[ 0.8 , -0.8 , 0.7 ]  Measurements=None  MoreParameters=off  BreakLoop=off  DataType=off  TransfoNumber=1
  T_280247955_110000;35000;10000_ПС_110_35_10_кВ_Кукшум : powerlib/Elements/Three-Phase Transformer (Two Windings)  Winding1Connection=Yg  UNITS=pu  NominalPower=[ 250e6 , 60 ]  Winding1=[110000,0.002,0.08]  Winding2Connection=Yg  Winding2=[110000,0.002,0.08]  SetSaturation=off  Rm=500  Lm=500  Saturation=[ 0,0 ; 0.0024,1.2 ; 1.0,1.52 ]  Hysteresis=off  DataFile='hysteresis'  SetInitialFlux=off  InitialFluxes=[ 0.8 , -0.8 , 0.7 ]  Measurements=None  MoreParameters=off  BreakLoop=off  DataType=off  TransfoNumber=1
  T_280247957_110000;35000;10000_ПС_110_35_10_кВ_ЯМЗ : powerlib/Elements/Three-Phase Transformer (Two Windings)  Winding1Connection=Yg  UNITS=pu  NominalPower=[ 250e6 , 60 ]  Winding1=[110000,0.002,0.08]  Winding2Connection=Yg  Winding2=[110000,0.002,0.08]  SetSaturation=off  Rm=500  Lm=500  Saturation=[ 0,0 ; 0.0024,1.2 ; 1.0,1.52 ]  Hysteresis=off  DataFile='hysteresis'  SetInitialFlux=off  InitialFluxes=[ 0.8 , -0.8 , 0.7 ]  Measurements=None  MoreParameters=off  BreakLoop=off  DataType=off  TransfoNumber=1
  T_280247962_110000;10000_ПС_110_10_кВ_Нискасы : powerlib/Elements/Three-Phase Transformer (Two Windings)  Winding1Connection=Yg  UNITS=pu  NominalPower=[ 250e6 , 60 ]  Winding1=[110000,0.002,0.08]  Winding2Connection=Yg  Winding2=[110000,0.002,0.08]  SetSaturation=off  Rm=500  Lm=500  Saturation=[ 0,0 ; 0.0024,1.2 ; 1.0,1.52 ]  Hysteresis=off  DataFile='hysteresis'  SetInitialFlux=off  InitialFluxes=[ 0.8 , -0.8 , 0.7 ]  Measurements=None  MoreParameters=off  BreakLoop=off  DataType=off  TransfoNumber=1
  T_280247964_110000;10000_ПС_110_10_кВ_Сундырь : powerlib/Elements/Three-Phase Transformer (Two Windings)  Winding1Connection=Yg  UNITS=pu  NominalPower=[ 250e6 , 60 ]  Winding1=[110000,0.002,0.08]  Winding2Connection=Yg  Winding2=[110000,0.002,0.08]  SetSaturation=off  Rm=500  Lm=500  Saturation=[ 0,0 ; 0.0024,1.2 ; 1.0,1.52 ]  Hysteresis=off  DataFile='hysteresis'  SetInitialFlux=off  InitialFluxes=[ 0.8 , -0.8 , 0.7 ]  Measurements=None  MoreParameters=off  BreakLoop=off  DataType=off  TransfoNumber=1
  T_280247969_110000;35000;10000_ПС_110_35_10_кВ_Моргауши : powerlib/Elements/Three-Phase Transformer (Two Windings)  Winding1Connection=Yg  UNITS=pu  NominalPower=[ 250e6 , 60 ]  Winding1=[110000,0.002,0.08]  Winding2Connection=Yg  Winding2=[110000,0.002,0.08]  SetSaturation=off  Rm=500  Lm=500  Saturation=[ 0,0 ; 0.0024,1.2 ; 1.0,1.52 ]  Hysteresis=off  DataFile='hysteresis'  SetInitialFlux=off  InitialFluxes=[ 0.8 , -0.8 , 0.7 ]  Measurements=None  MoreParameters=off  BreakLoop=off  DataType=off  TransfoNumber=1
  T_281834842_110000;35000;10000_ПС_110_35_10_кВ_Катраси : powerlib/Elements/Three-Phase Transformer (Two Windings)  Winding1Connection=Yg  UNITS=pu  NominalPower=[ 250e6 , 60 ]  Winding1=[110000,0.002,0.08]  Winding2Connection=Yg  Winding2=[110000,0.002,0.08]  SetSaturation=off  Rm=500  Lm=500  Saturation=[ 0,0 ; 0.0024,1.2 ; 1.0,1.52 ]  Hysteresis=off  DataFile='hysteresis'  SetInitialFlux=off  InitialFluxes=[ 0.8 , -0.8 , 0.7 ]  Measurements=None  MoreParameters=off  BreakLoop=off  DataType=off  TransfoNumber=1
  T_281834847_110000;35000;10000_ПС_110_35_10_кВ_Кугеси : powerlib/Elements/Three-Phase Transformer (Two Windings)  Winding1Connection=Yg  UNITS=pu  NominalPower=[ 250e6 , 60 ]  Winding1=[110000,0.002,0.08]  Winding2Connection=Yg  Winding2=[110000,0.002,0.08]  SetSaturation=off  Rm=500  Lm=500  Saturation=[ 0,0 ; 0.0024,1.2 ; 1.0,1.52 ]  Hysteresis=off  DataFile='hysteresis'  SetInitialFlux=off  InitialFluxes=[ 0.8 , -0.8 , 0.7 ]  Measurements=None  MoreParameters=off  BreakLoop=off  DataType=off  TransfoNumber=1
  T_281879365_110000;10000_ПС_110_10_кВ_Светлая : powerlib/Elements/Three-Phase Transformer (Two Windings)  Winding1Connection=Yg  UNITS=pu  NominalPower=[ 250e6 , 60 ]  Winding1=[110000,0.002,0.08]  Winding2Connection=Yg  Winding2=[110000,0.002,0.08]  SetSaturation=off  Rm=500  Lm=500  Saturation=[ 0,0 ; 0.0024,1.2 ; 1.0,1.52 ]  Hysteresis=off  DataFile='hysteresis'  SetInitialFlux=off  InitialFluxes=[ 0.8 , -0.8 , 0.7 ]  Measurements=None  MoreParameters=off  BreakLoop=off  DataType=off  TransfoNumber=1
  T_281879368_110000;10000_ПС_110_10_кВ_Радуга : powerlib/Elements/Three-Phase Transformer (Two Windings)  Winding1Connection=Yg  UNITS=pu  NominalPower=[ 250e6 , 60 ]  Winding1=[110000,0.002,0.08]  Winding2Connection=Yg  Winding2=[110000,0.002,0.08]  SetSaturation=off  Rm=500  Lm=500  Saturation=[ 0,0 ; 0.0024,1.2 ; 1.0,1.52 ]  Hysteresis=off  DataFile='hysteresis'  SetInitialFlux=off  InitialFluxes=[ 0.8 , -0.8 , 0.7 ]  Measurements=None  MoreParameters=off  BreakLoop=off  DataType=off  TransfoNumber=1
  T_283379848_220000_ПС_220_кВ_Сива : powerlib/Elements/Three-Phase Transformer (Two Windings)  Winding1Connection=Yg  UNITS=pu  NominalPower=[ 250e6 , 60 ]  Winding1=[110000,0.002,0.08]  Winding2Connection=Yg  Winding2=[110000,0.002,0.08]  SetSaturation=off  Rm=500  Lm=500  Saturation=[ 0,0 ; 0.0024,1.2 ; 1.0,1.52 ]  Hysteresis=off  DataFile='hysteresis'  SetInitialFlux=off  InitialFluxes=[ 0.8 , -0.8 , 0.7 ]  Measurements=None  MoreParameters=off  BreakLoop=off  DataType=off  TransfoNumber=1
  T_286921936__ : powerlib/Elements/Three-Phase Transformer (Two Windings)  Winding1Connection=Yg  UNITS=pu  NominalPower=[ 250e6 , 60 ]  Winding1=[110000,0.002,0.08]  Winding2Connection=Yg  Winding2=[110000,0.002,0.08]  SetSaturation=off  Rm=500  Lm=500  Saturation=[ 0,0 ; 0.0024,1.2 ; 1.0,1.52 ]  Hysteresis=off  DataFile='hysteresis'  SetInitialFlux=off  InitialFluxes=[ 0.8 , -0.8 , 0.7 ]  Measurements=None  MoreParameters=off  BreakLoop=off  DataType=off  TransfoNumber=1
  T_287462706_110000_110_КВ_Тёплая_Гора : powerlib/Elements/Three-Phase Transformer (Two Windings)  Winding1Connection=Yg  UNITS=pu  NominalPower=[ 250e6 , 60 ]  Winding1=[110000,0.002,0.08]  Winding2Connection=Yg  Winding2=[110000,0.002,0.08]  SetSaturation=off  Rm=500  Lm=500  Saturation=[ 0,0 ; 0.0024,1.2 ; 1.0,1.52 ]  Hysteresis=off  DataFile='hysteresis'  SetInitialFlux=off  InitialFluxes=[ 0.8 , -0.8 , 0.7 ]  Measurements=None  MoreParameters=off  BreakLoop=off  DataType=off  TransfoNumber=1
  T_290776375_110000_ПС_ЗАГОТОВКА : powerlib/Elements/Three-Phase Transformer (Two Windings)  Winding1Connection=Yg  UNITS=pu  NominalPower=[ 250e6 , 60 ]  Winding1=[110000,0.002,0.08]  Winding2Connection=Yg  Winding2=[110000,0.002,0.08]  SetSaturation=off  Rm=500  Lm=500  Saturation=[ 0,0 ; 0.0024,1.2 ; 1.0,1.52 ]  Hysteresis=off  DataFile='hysteresis'  SetInitialFlux=off  InitialFluxes=[ 0.8 , -0.8 , 0.7 ]  Measurements=None  MoreParameters=off  BreakLoop=off  DataType=off  TransfoNumber=1
  T_290777752_110000_ГРЕМЯЧАЯ_I : powerlib/Elements/Three-Phase Transformer (Two Windings)  Winding1Connection=Yg  UNITS=pu  NominalPower=[ 250e6 , 60 ]  Winding1=[110000,0.002,0.08]  Winding2Connection=Yg  Winding2=[110000,0.002,0.08]  SetSaturation=off  Rm=500  Lm=500  Saturation=[ 0,0 ; 0.0024,1.2 ; 1.0,1.52 ]  Hysteresis=off  DataFile='hysteresis'  SetInitialFlux=off  InitialFluxes=[ 0.8 , -0.8 , 0.7 ]  Measurements=None  MoreParameters=off  BreakLoop=off  DataType=off  TransfoNumber=1
  T_291372085_110000_пс_Кутамыш : powerlib/Elements/Three-Phase Transformer (Two Windings)  Winding1Connection=Yg  UNITS=pu  NominalPower=[ 250e6 , 60 ]  Winding1=[110000,0.002,0.08]  Winding2Connection=Yg  Winding2=[110000,0.002,0.08]  SetSaturation=off  Rm=500  Lm=500  Saturation=[ 0,0 ; 0.0024,1.2 ; 1.0,1.52 ]  Hysteresis=off  DataFile='hysteresis'  SetInitialFlux=off  InitialFluxes=[ 0.8 , -0.8 , 0.7 ]  Measurements=None  MoreParameters=off  BreakLoop=off  DataType=off  TransfoNumber=1
  T_291372086_110000_пс_Села_110_10кВ : powerlib/Elements/Three-Phase Transformer (Two Windings)  Winding1Connection=Yg  UNITS=pu  NominalPower=[ 250e6 , 60 ]  Winding1=[110000,0.002,0.08]  Winding2Connection=Yg  Winding2=[110000,0.002,0.08]  SetSaturation=off  Rm=500  Lm=500  Saturation=[ 0,0 ; 0.0024,1.2 ; 1.0,1.52 ]  Hysteresis=off  DataFile='hysteresis'  SetInitialFlux=off  InitialFluxes=[ 0.8 , -0.8 , 0.7 ]  Measurements=None  MoreParameters=off  BreakLoop=off  DataType=off  TransfoNumber=1
  T_292068563_110000;35000;10000_ПС_110_35_10_кВ_Еласы : powerlib/Elements/Three-Phase Transformer (Two Windings)  Winding1Connection=Yg  UNITS=pu  NominalPower=[ 250e6 , 60 ]  Winding1=[110000,0.002,0.08]  Winding2Connection=Yg  Winding2=[110000,0.002,0.08]  SetSaturation=off  Rm=500  Lm=500  Saturation=[ 0,0 ; 0.0024,1.2 ; 1.0,1.52 ]  Hysteresis=off  DataFile='hysteresis'  SetInitialFlux=off  InitialFluxes=[ 0.8 , -0.8 , 0.7 ]  Measurements=None  MoreParameters=off  BreakLoop=off  DataType=off  TransfoNumber=1
  T_292328535_110000;10000_ПС_110_10_кВ_Виловатово : powerlib/Elements/Three-Phase Transformer (Two Windings)  Winding1Connection=Yg  UNITS=pu  NominalPower=[ 250e6 , 60 ]  Winding1=[110000,0.002,0.08]  Winding2Connection=Yg  Winding2=[110000,0.002,0.08]  SetSaturation=off  Rm=500  Lm=500  Saturation=[ 0,0 ; 0.0024,1.2 ; 1.0,1.52 ]  Hysteresis=off  DataFile='hysteresis'  SetInitialFlux=off  InitialFluxes=[ 0.8 , -0.8 , 0.7 ]  Measurements=None  MoreParameters=off  BreakLoop=off  DataType=off  TransfoNumber=1
  "T_305832833_110000_ПС_110_10кВ_\"Мадаево\"" : powerlib/Elements/Three-Phase Transformer (Two Windings)  Winding1Connection=Yg  UNITS=pu  NominalPower=[ 250e6 , 60 ]  Winding1=[110000,0.002,0.08]  Winding2Connection=Yg  Winding2=[110000,0.002,0.08]  SetSaturation=off  Rm=500  Lm=500  Saturation=[ 0,0 ; 0.0024,1.2 ; 1.0,1.52 ]  Hysteresis=off  DataFile='hysteresis'  SetInitialFlux=off  InitialFluxes=[ 0.8 , -0.8 , 0.7 ]  Measurements=None  MoreParameters=off  BreakLoop=off  DataType=off  TransfoNumber=1
  T_305832836_220000_Лукояновская : powerlib/Elements/Three-Phase Transformer (Two Windings)  Winding1Connection=Yg  UNITS=pu  NominalPower=[ 250e6 , 60 ]  Winding1=[220000,0.002,0.08]  Winding2Connection=Yg  Winding2=[220000,0.002,0.08]  SetSaturation=off  Rm=500  Lm=500  Saturation=[ 0,0 ; 0.0024,1.2 ; 1.0,1.52 ]  Hysteresis=off  DataFile='hysteresis'  SetInitialFlux=off  InitialFluxes=[ 0.8 , -0.8 , 0.7 ]  Measurements=None  MoreParameters=off  BreakLoop=off  DataType=off  TransfoNumber=1
  T_305893253_220000;10000_ПС_Абашево_220_10_кВ : powerlib/Elements/Three-Phase Transformer (Two Windings)  Winding1Connection=Yg  UNITS=pu  NominalPower=[ 250e6 , 60 ]  Winding1=[220000,0.002,0.08]  Winding2Connection=Yg  Winding2=[220000,0.002,0.08]  SetSaturation=off  Rm=500  Lm=500  Saturation=[ 0,0 ; 0.0024,1.2 ; 1.0,1.52 ]  Hysteresis=off  DataFile='hysteresis'  SetInitialFlux=off  InitialFluxes=[ 0.8 , -0.8 , 0.7 ]  Measurements=None  MoreParameters=off  BreakLoop=off  DataType=off  TransfoNumber=1
  T_306106528__Екатериновка_газовая : powerlib/Elements/Three-Phase Transformer (Two Windings)  Winding1Connection=Yg  UNITS=pu  NominalPower=[ 250e6 , 60 ]  Winding1=[220000,0.002,0.08]  Winding2Connection=Yg  Winding2=[220000,0.002,0.08]  SetSaturation=off  Rm=500  Lm=500  Saturation=[ 0,0 ; 0.0024,1.2 ; 1.0,1.52 ]  Hysteresis=off  DataFile='hysteresis'  SetInitialFlux=off  InitialFluxes=[ 0.8 , -0.8 , 0.7 ]  Measurements=None  MoreParameters=off  BreakLoop=off  DataType=off  TransfoNumber=1
  T_307428692__Сибирь : powerlib/Elements/Three-Phase Transformer (Two Windings)  Winding1Connection=Yg  UNITS=pu  NominalPower=[ 250e6 , 60 ]  Winding1=[110000,0.002,0.08]  Winding2Connection=Yg  Winding2=[110000,0.002,0.08]  SetSaturation=off  Rm=500  Lm=500  Saturation=[ 0,0 ; 0.0024,1.2 ; 1.0,1.52 ]  Hysteresis=off  DataFile='hysteresis'  SetInitialFlux=off  InitialFluxes=[ 0.8 , -0.8 , 0.7 ]  Measurements=None  MoreParameters=off  BreakLoop=off  DataType=off  TransfoNumber=1
  T_308883878__ : powerlib/Elements/Three-Phase Transformer (Two Windings)  Winding1Connection=Yg  UNITS=pu  NominalPower=[ 250e6 , 60 ]  Winding1=[110000,0.002,0.08]  Winding2Connection=Yg  Winding2=[110000,0.002,0.08]  SetSaturation=off  Rm=500  Lm=500  Saturation=[ 0,0 ; 0.0024,1.2 ; 1.0,1.52 ]  Hysteresis=off  DataFile='hysteresis'  SetInitialFlux=off  InitialFluxes=[ 0.8 , -0.8 , 0.7 ]  Measurements=None  MoreParameters=off  BreakLoop=off  DataType=off  TransfoNumber=1
  T_310752804_110000;35000;10000_ПС_«Чапаевская»_110_35_10_кВ : powerlib/Elements/Three-Phase Transformer (Two Windings)  Winding1Connection=Yg  UNITS=pu  NominalPower=[ 250e6 , 60 ]  Winding1=[110000,0.002,0.08]  Winding2Connection=Yg  Winding2=[110000,0.002,0.08]  SetSaturation=off  Rm=500  Lm=500  Saturation=[ 0,0 ; 0.0024,1.2 ; 1.0,1.52 ]  Hysteresis=off  DataFile='hysteresis'  SetInitialFlux=off  InitialFluxes=[ 0.8 , -0.8 , 0.7 ]  Measurements=None  MoreParameters=off  BreakLoop=off  DataType=off  TransfoNumber=1
  T_311468947__ОРУ_ТЭЦ_3 : powerlib/Elements/Three-Phase Transformer (Two Windings)  Winding1Connection=Yg  UNITS=pu  NominalPower=[ 250e6 , 60 ]  Winding1=[110000,0.002,0.08]  Winding2Connection=Yg  Winding2=[110000,0.002,0.08]  SetSaturation=off  Rm=500  Lm=500  Saturation=[ 0,0 ; 0.0024,1.2 ; 1.0,1.52 ]  Hysteresis=off  DataFile='hysteresis'  SetInitialFlux=off  InitialFluxes=[ 0.8 , -0.8 , 0.7 ]  Measurements=None  MoreParameters=off  BreakLoop=off  DataType=off  TransfoNumber=1
  T_313773131__ : powerlib/Elements/Three-Phase Transformer (Two Windings)  Winding1Connection=Yg  UNITS=pu  NominalPower=[ 250e6 , 60 ]  Winding1=[110000,0.002,0.08]  Winding2Connection=Yg  Winding2=[110000,0.002,0.08]  SetSaturation=off  Rm=500  Lm=500  Saturation=[ 0,0 ; 0.0024,1.2 ; 1.0,1.52 ]  Hysteresis=off  DataFile='hysteresis'  SetInitialFlux=off  InitialFluxes=[ 0.8 , -0.8 , 0.7 ]  Measurements=None  MoreParameters=off  BreakLoop=off  DataType=off  TransfoNumber=1
  T_313773134_110000;35000;6000_ПС_110_35_6_кВ_Порт : powerlib/Elements/Three-Phase Transformer (Two Windings)  Winding1Connection=Yg  UNITS=pu  NominalPower=[ 250e6 , 60 ]  Winding1=[110000,0.002,0.08]  Winding2Connection=Yg  Winding2=[110000,0.002,0.08]  SetSaturation=off  Rm=500  Lm=500  Saturation=[ 0,0 ; 0.0024,1.2 ; 1.0,1.52 ]  Hysteresis=off  DataFile='hysteresis'  SetInitialFlux=off  InitialFluxes=[ 0.8 , -0.8 , 0.7 ]  Measurements=None  MoreParameters=off  BreakLoop=off  DataType=off  TransfoNumber=1
  T_315675920_110000;10000_ПС_Покров_Майдан_110_10_кВ : powerlib/Elements/Three-Phase Transformer (Two Windings)  Winding1Connection=Yg  UNITS=pu  NominalPower=[ 250e6 , 60 ]  Winding1=[110000,0.002,0.08]  Winding2Connection=Yg  Winding2=[110000,0.002,0.08]  SetSaturation=off  Rm=500  Lm=500  Saturation=[ 0,0 ; 0.0024,1.2 ; 1.0,1.52 ]  Hysteresis=off  DataFile='hysteresis'  SetInitialFlux=off  InitialFluxes=[ 0.8 , -0.8 , 0.7 ]  Measurements=None  MoreParameters=off  BreakLoop=off  DataType=off  TransfoNumber=1
  T_319459210__ : powerlib/Elements/Three-Phase Transformer (Two Windings)  Winding1Connection=Yg  UNITS=pu  NominalPower=[ 250e6 , 60 ]  Winding1=[110000,0.002,0.08]  Winding2Connection=Yg  Winding2=[110000,0.002,0.08]  SetSaturation=off  Rm=500  Lm=500  Saturation=[ 0,0 ; 0.0024,1.2 ; 1.0,1.52 ]  Hysteresis=off  DataFile='hysteresis'  SetInitialFlux=off  InitialFluxes=[ 0.8 , -0.8 , 0.7 ]  Measurements=None  MoreParameters=off  BreakLoop=off  DataType=off  TransfoNumber=1
  T_319459220_110000;10000_Перемская : powerlib/Elements/Three-Phase Transformer (Two Windings)  Winding1Connection=Yg  UNITS=pu  NominalPower=[ 250e6 , 60 ]  Winding1=[110000,0.002,0.08]  Winding2Connection=Yg  Winding2=[110000,0.002,0.08]  SetSaturation=off  Rm=500  Lm=500  Saturation=[ 0,0 ; 0.0024,1.2 ; 1.0,1.52 ]  Hysteresis=off  DataFile='hysteresis'  SetInitialFlux=off  InitialFluxes=[ 0.8 , -0.8 , 0.7 ]  Measurements=None  MoreParameters=off  BreakLoop=off  DataType=off  TransfoNumber=1
  T_320965592__ : powerlib/Elements/Three-Phase Transformer (Two Windings)  Winding1Connection=Yg  UNITS=pu  NominalPower=[ 250e6 , 60 ]  Winding1=[110000,0.002,0.08]  Winding2Connection=Yg  Winding2=[110000,0.002,0.08]  SetSaturation=off  Rm=500  Lm=500  Saturation=[ 0,0 ; 0.0024,1.2 ; 1.0,1.52 ]  Hysteresis=off  DataFile='hysteresis'  SetInitialFlux=off  InitialFluxes=[ 0.8 , -0.8 , 0.7 ]  Measurements=None  MoreParameters=off  BreakLoop=off  DataType=off  TransfoNumber=1
  "T_327138157_220000_ПС_220кВ_\"Пильна\"" : powerlib/Elements/Three-Phase Transformer (Two Windings)  Winding1Connection=Yg  UNITS=pu  NominalPower=[ 250e6 , 60 ]  Winding1=[220000,0.002,0.08]  Winding2Connection=Yg  Winding2=[220000,0.002,0.08]  SetSaturation=off  Rm=500  Lm=500  Saturation=[ 0,0 ; 0.0024,1.2 ; 1.0,1.52 ]  Hysteresis=off  DataFile='hysteresis'  SetInitialFlux=off  InitialFluxes=[ 0.8 , -0.8 , 0.7 ]  Measurements=None  MoreParameters=off  BreakLoop=off  DataType=off  TransfoNumber=1
  T_327226015_220000_Починковская_2 : powerlib/Elements/Three-Phase Transformer (Two Windings)  Winding1Connection=Yg  UNITS=pu  NominalPower=[ 250e6 , 60 ]  Winding1=[220000,0.002,0.08]  Winding2Connection=Yg  Winding2=[220000,0.002,0.08]  SetSaturation=off  Rm=500  Lm=500  Saturation=[ 0,0 ; 0.0024,1.2 ; 1.0,1.52 ]  Hysteresis=off  DataFile='hysteresis'  SetInitialFlux=off  InitialFluxes=[ 0.8 , -0.8 , 0.7 ]  Measurements=None  MoreParameters=off  BreakLoop=off  DataType=off  TransfoNumber=1
  T_327226025_220000_Починковская_1 : powerlib/Elements/Three-Phase Transformer (Two Windings)  Winding1Connection=Yg  UNITS=pu  NominalPower=[ 250e6 , 60 ]  Winding1=[220000,0.002,0.08]  Winding2Connection=Yg  Winding2=[220000,0.002,0.08]  SetSaturation=off  Rm=500  Lm=500  Saturation=[ 0,0 ; 0.0024,1.2 ; 1.0,1.52 ]  Hysteresis=off  DataFile='hysteresis'  SetInitialFlux=off  InitialFluxes=[ 0.8 , -0.8 , 0.7 ]  Measurements=None  MoreParameters=off  BreakLoop=off  DataType=off  TransfoNumber=1
  "T_327245366_110000_ПС_110_10кВ_\"Разино\"" : powerlib/Elements/Three-Phase Transformer (Two Windings)  Winding1Connection=Yg  UNITS=pu  NominalPower=[ 250e6 , 60 ]  Winding1=[110000,0.002,0.08]  Winding2Connection=Yg  Winding2=[110000,0.002,0.08]  SetSaturation=off  Rm=500  Lm=500  Saturation=[ 0,0 ; 0.0024,1.2 ; 1.0,1.52 ]  Hysteresis=off  DataFile='hysteresis'  SetInitialFlux=off  InitialFluxes=[ 0.8 , -0.8 , 0.7 ]  Measurements=None  MoreParameters=off  BreakLoop=off  DataType=off  TransfoNumber=1
  "T_327245371_110000_ПС_110_35_10кВ_\"Починки_110\"" : powerlib/Elements/Three-Phase Transformer (Two Windings)  Winding1Connection=Yg  UNITS=pu  NominalPower=[ 250e6 , 60 ]  Winding1=[110000,0.002,0.08]  Winding2Connection=Yg  Winding2=[110000,0.002,0.08]  SetSaturation=off  Rm=500  Lm=500  Saturation=[ 0,0 ; 0.0024,1.2 ; 1.0,1.52 ]  Hysteresis=off  DataFile='hysteresis'  SetInitialFlux=off  InitialFluxes=[ 0.8 , -0.8 , 0.7 ]  Measurements=None  MoreParameters=off  BreakLoop=off  DataType=off  TransfoNumber=1
  "T_327245584_110000_ПС_110_10кВ_\"Лукоянов_110\"" : powerlib/Elements/Three-Phase Transformer (Two Windings)  Winding1Connection=Yg  UNITS=pu  NominalPower=[ 250e6 , 60 ]  Winding1=[110000,0.002,0.08]  Winding2Connection=Yg  Winding2=[110000,0.002,0.08]  SetSaturation=off  Rm=500  Lm=500  Saturation=[ 0,0 ; 0.0024,1.2 ; 1.0,1.52 ]  Hysteresis=off  DataFile='hysteresis'  SetInitialFlux=off  InitialFluxes=[ 0.8 , -0.8 , 0.7 ]  Measurements=None  MoreParameters=off  BreakLoop=off  DataType=off  TransfoNumber=1
  T_327325460_220000_Кудьма : powerlib/Elements/Three-Phase Transformer (Two Windings)  Winding1Connection=Yg  UNITS=pu  NominalPower=[ 250e6 , 60 ]  Winding1=[220000,0.002,0.08]  Winding2Connection=Yg  Winding2=[220000,0.002,0.08]  SetSaturation=off  Rm=500  Lm=500  Saturation=[ 0,0 ; 0.0024,1.2 ; 1.0,1.52 ]  Hysteresis=off  DataFile='hysteresis'  SetInitialFlux=off  InitialFluxes=[ 0.8 , -0.8 , 0.7 ]  Measurements=None  MoreParameters=off  BreakLoop=off  DataType=off  TransfoNumber=1
  T_327816066_220000_Кузнецк : powerlib/Elements/Three-Phase Transformer (Two Windings)  Winding1Connection=Yg  UNITS=pu  NominalPower=[ 250e6 , 60 ]  Winding1=[220000,0.002,0.08]  Winding2Connection=Yg  Winding2=[220000,0.002,0.08]  SetSaturation=off  Rm=500  Lm=500  Saturation=[ 0,0 ; 0.0024,1.2 ; 1.0,1.52 ]  Hysteresis=off  DataFile='hysteresis'  SetInitialFlux=off  InitialFluxes=[ 0.8 , -0.8 , 0.7 ]  Measurements=None  MoreParameters=off  BreakLoop=off  DataType=off  TransfoNumber=1
  T_328463572__ : powerlib/Elements/Three-Phase Transformer (Two Windings)  Winding1Connection=Yg  UNITS=pu  NominalPower=[ 250e6 , 60 ]  Winding1=[220000,0.002,0.08]  Winding2Connection=Yg  Winding2=[220000,0.002,0.08]  SetSaturation=off  Rm=500  Lm=500  Saturation=[ 0,0 ; 0.0024,1.2 ; 1.0,1.52 ]  Hysteresis=off  DataFile='hysteresis'  SetInitialFlux=off  InitialFluxes=[ 0.8 , -0.8 , 0.7 ]  Measurements=None  MoreParameters=off  BreakLoop=off  DataType=off  TransfoNumber=1
  T_329997654_110000_ : powerlib/Elements/Three-Phase Transformer (Two Windings)  Winding1Connection=Yg  UNITS=pu  NominalPower=[ 250e6 , 60 ]  Winding1=[110000,0.002,0.08]  Winding2Connection=Yg  Winding2=[110000,0.002,0.08]  SetSaturation=off  Rm=500  Lm=500  Saturation=[ 0,0 ; 0.0024,1.2 ; 1.0,1.52 ]  Hysteresis=off  DataFile='hysteresis'  SetInitialFlux=off  InitialFluxes=[ 0.8 , -0.8 , 0.7 ]  Measurements=None  MoreParameters=off  BreakLoop=off  DataType=off  TransfoNumber=1
  T_330006647_110000_ : powerlib/Elements/Three-Phase Transformer (Two Windings)  Winding1Connection=Yg  UNITS=pu  NominalPower=[ 250e6 , 60 ]  Winding1=[110000,0.002,0.08]  Winding2Connection=Yg  Winding2=[110000,0.002,0.08]  SetSaturation=off  Rm=500  Lm=500  Saturation=[ 0,0 ; 0.0024,1.2 ; 1.0,1.52 ]  Hysteresis=off  DataFile='hysteresis'  SetInitialFlux=off  InitialFluxes=[ 0.8 , -0.8 , 0.7 ]  Measurements=None  MoreParameters=off  BreakLoop=off  DataType=off  TransfoNumber=1
  T_330052123_110000_ПС_110_6_кВ_Прудовая : powerlib/Elements/Three-Phase Transformer (Two Windings)  Winding1Connection=Yg  UNITS=pu  NominalPower=[ 250e6 , 60 ]  Winding1=[110000,0.002,0.08]  Winding2Connection=Yg  Winding2=[110000,0.002,0.08]  SetSaturation=off  Rm=500  Lm=500  Saturation=[ 0,0 ; 0.0024,1.2 ; 1.0,1.52 ]  Hysteresis=off  DataFile='hysteresis'  SetInitialFlux=off  InitialFluxes=[ 0.8 , -0.8 , 0.7 ]  Measurements=None  MoreParameters=off  BreakLoop=off  DataType=off  TransfoNumber=1
  T_337947383__ : powerlib/Elements/Three-Phase Transformer (Two Windings)  Winding1Connection=Yg  UNITS=pu  NominalPower=[ 250e6 , 60 ]  Winding1=[110000,0.002,0.08]  Winding2Connection=Yg  Winding2=[110000,0.002,0.08]  SetSaturation=off  Rm=500  Lm=500  Saturation=[ 0,0 ; 0.0024,1.2 ; 1.0,1.52 ]  Hysteresis=off  DataFile='hysteresis'  SetInitialFlux=off  InitialFluxes=[ 0.8 , -0.8 , 0.7 ]  Measurements=None  MoreParameters=off  BreakLoop=off  DataType=off  TransfoNumber=1
  T_351596015__ПС_Ромодан : powerlib/Elements/Three-Phase Transformer (Two Windings)  Winding1Connection=Yg  UNITS=pu  NominalPower=[ 250e6 , 60 ]  Winding1=[110000,0.002,0.08]  Winding2Connection=Yg  Winding2=[110000,0.002,0.08]  SetSaturation=off  Rm=500  Lm=500  Saturation=[ 0,0 ; 0.0024,1.2 ; 1.0,1.52 ]  Hysteresis=off  DataFile='hysteresis'  SetInitialFlux=off  InitialFluxes=[ 0.8 , -0.8 , 0.7 ]  Measurements=None  MoreParameters=off  BreakLoop=off  DataType=off  TransfoNumber=1
  T_363144177__ОРУ_500_кВ_ИрГРЭС___1 : powerlib/Elements/Three-Phase Transformer (Two Windings)  Winding1Connection=Yg  UNITS=pu  NominalPower=[ 250e6 , 60 ]  Winding1=[500000,0.002,0.08]  Winding2Connection=Yg  Winding2=[500000,0.002,0.08]  SetSaturation=off  Rm=500  Lm=500  Saturation=[ 0,0 ; 0.0024,1.2 ; 1.0,1.52 ]  Hysteresis=off  DataFile='hysteresis'  SetInitialFlux=off  InitialFluxes=[ 0.8 , -0.8 , 0.7 ]  Measurements=None  MoreParameters=off  BreakLoop=off  DataType=off  TransfoNumber=1
  T_376942192__ : powerlib/Elements/Three-Phase Transformer (Two Windings)  Winding1Connection=Yg  UNITS=pu  NominalPower=[ 250e6 , 60 ]  Winding1=[500000,0.002,0.08]  Winding2Connection=Yg  Winding2=[500000,0.002,0.08]  SetSaturation=off  Rm=500  Lm=500  Saturation=[ 0,0 ; 0.0024,1.2 ; 1.0,1.52 ]  Hysteresis=off  DataFile='hysteresis'  SetInitialFlux=off  InitialFluxes=[ 0.8 , -0.8 , 0.7 ]  Measurements=None  MoreParameters=off  BreakLoop=off  DataType=off  TransfoNumber=1
  T_48949159_220000;35000_ : powerlib/Elements/Three-Phase Transformer (Two Windings)  Winding1Connection=Yg  UNITS=pu  NominalPower=[ 250e6 , 60 ]  Winding1=[220000,0.002,0.08]  Winding2Connection=Yg  Winding2=[220000,0.002,0.08]  SetSaturation=off  Rm=500  Lm=500  Saturation=[ 0,0 ; 0.0024,1.2 ; 1.0,1.52 ]  Hysteresis=off  DataFile='hysteresis'  SetInitialFlux=off  InitialFluxes=[ 0.8 , -0.8 , 0.7 ]  Measurements=None  MoreParameters=off  BreakLoop=off  DataType=off  TransfoNumber=1
  "T_51601242_220000;110000;fixme_ПС_220_кВ_\"Центральная\"" : powerlib/Elements/Three-Phase Transformer (Two Windings)  Winding1Connection=Yg  UNITS=pu  NominalPower=[ 250e6 , 60 ]  Winding1=[110000,0.002,0.08]  Winding2Connection=Yg  Winding2=[110000,0.002,0.08]  SetSaturation=off  Rm=500  Lm=500  Saturation=[ 0,0 ; 0.0024,1.2 ; 1.0,1.52 ]  Hysteresis=off  DataFile='hysteresis'  SetInitialFlux=off  InitialFluxes=[ 0.8 , -0.8 , 0.7 ]  Measurements=None  MoreParameters=off  BreakLoop=off  DataType=off  TransfoNumber=1
  T_51711046_220000;110000;fixme_ : powerlib/Elements/Three-Phase Transformer (Two Windings)  Winding1Connection=Yg  UNITS=pu  NominalPower=[ 250e6 , 60 ]  Winding1=[220000,0.002,0.08]  Winding2Connection=Yg  Winding2=[220000,0.002,0.08]  SetSaturation=off  Rm=500  Lm=500  Saturation=[ 0,0 ; 0.0024,1.2 ; 1.0,1.52 ]  Hysteresis=off  DataFile='hysteresis'  SetInitialFlux=off  InitialFluxes=[ 0.8 , -0.8 , 0.7 ]  Measurements=None  MoreParameters=off  BreakLoop=off  DataType=off  TransfoNumber=1
  T_51711248_110000_ : powerlib/Elements/Three-Phase Transformer (Two Windings)  Winding1Connection=Yg  UNITS=pu  NominalPower=[ 250e6 , 60 ]  Winding1=[110000,0.002,0.08]  Winding2Connection=Yg  Winding2=[110000,0.002,0.08]  SetSaturation=off  Rm=500  Lm=500  Saturation=[ 0,0 ; 0.0024,1.2 ; 1.0,1.52 ]  Hysteresis=off  DataFile='hysteresis'  SetInitialFlux=off  InitialFluxes=[ 0.8 , -0.8 , 0.7 ]  Measurements=None  MoreParameters=off  BreakLoop=off  DataType=off  TransfoNumber=1
  T_53015400_500000_ПС_Калино : powerlib/Elements/Three-Phase Transformer (Two Windings)  Winding1Connection=Yg  UNITS=pu  NominalPower=[ 250e6 , 60 ]  Winding1=[500000,0.002,0.08]  Winding2Connection=Yg  Winding2=[500000,0.002,0.08]  SetSaturation=off  Rm=500  Lm=500  Saturation=[ 0,0 ; 0.0024,1.2 ; 1.0,1.52 ]  Hysteresis=off  DataFile='hysteresis'  SetInitialFlux=off  InitialFluxes=[ 0.8 , -0.8 , 0.7 ]  Measurements=None  MoreParameters=off  BreakLoop=off  DataType=off  TransfoNumber=1
  T_53366641_220000;110000;6000_ПС_Канаш_220_110_6_кВ : powerlib/Elements/Three-Phase Transformer (Two Windings)  Winding1Connection=Yg  UNITS=pu  NominalPower=[ 250e6 , 60 ]  Winding1=[220000,0.002,0.08]  Winding2Connection=Yg  Winding2=[110000,0.002,0.08]  SetSaturation=off  Rm=500  Lm=500  Saturation=[ 0,0 ; 0.0024,1.2 ; 1.0,1.52 ]  Hysteresis=off  DataFile='hysteresis'  SetInitialFlux=off  InitialFluxes=[ 0.8 , -0.8 , 0.7 ]  Measurements=None  MoreParameters=off  BreakLoop=off  DataType=off  TransfoNumber=1
  T_53566695__Подстанция_Кизел_(ж_д) : powerlib/Elements/Three-Phase Transformer (Two Windings)  Winding1Connection=Yg  UNITS=pu  NominalPower=[ 250e6 , 60 ]  Winding1=[110000,0.002,0.08]  Winding2Connection=Yg  Winding2=[110000,0.002,0.08]  SetSaturation=off  Rm=500  Lm=500  Saturation=[ 0,0 ; 0.0024,1.2 ; 1.0,1.52 ]  Hysteresis=off  DataFile='hysteresis'  SetInitialFlux=off  InitialFluxes=[ 0.8 , -0.8 , 0.7 ]  Measurements=None  MoreParameters=off  BreakLoop=off  DataType=off  TransfoNumber=1
  T_55334100__ : powerlib/Elements/Three-Phase Transformer (Two Windings)  Winding1Connection=Yg  UNITS=pu  NominalPower=[ 250e6 , 60 ]  Winding1=[110000,0.002,0.08]  Winding2Connection=Yg  Winding2=[110000,0.002,0.08]  SetSaturation=off  Rm=500  Lm=500  Saturation=[ 0,0 ; 0.0024,1.2 ; 1.0,1.52 ]  Hysteresis=off  DataFile='hysteresis'  SetInitialFlux=off  InitialFluxes=[ 0.8 , -0.8 , 0.7 ]  Measurements=None  MoreParameters=off  BreakLoop=off  DataType=off  TransfoNumber=1
  T_55334115__ : powerlib/Elements/Three-Phase Transformer (Two Windings)  Winding1Connection=Yg  UNITS=pu  NominalPower=[ 250e6 , 60 ]  Winding1=[110000,0.002,0.08]  Winding2Connection=Yg  Winding2=[110000,0.002,0.08]  SetSaturation=off  Rm=500  Lm=500  Saturation=[ 0,0 ; 0.0024,1.2 ; 1.0,1.52 ]  Hysteresis=off  DataFile='hysteresis'  SetInitialFlux=off  InitialFluxes=[ 0.8 , -0.8 , 0.7 ]  Measurements=None  MoreParameters=off  BreakLoop=off  DataType=off  TransfoNumber=1
  "T_56048772_220000_Электрическая_подстанция_\"Горная\"" : powerlib/Elements/Three-Phase Transformer (Two Windings)  Winding1Connection=Yg  UNITS=pu  NominalPower=[ 250e6 , 60 ]  Winding1=[110000,0.002,0.08]  Winding2Connection=Yg  Winding2=[110000,0.002,0.08]  SetSaturation=off  Rm=500  Lm=500  Saturation=[ 0,0 ; 0.0024,1.2 ; 1.0,1.52 ]  Hysteresis=off  DataFile='hysteresis'  SetInitialFlux=off  InitialFluxes=[ 0.8 , -0.8 , 0.7 ]  Measurements=None  MoreParameters=off  BreakLoop=off  DataType=off  TransfoNumber=1
  T_57948286_110000;10000_Сазанлей : powerlib/Elements/Three-Phase Transformer (Two Windings)  Winding1Connection=Yg  UNITS=pu  NominalPower=[ 250e6 , 60 ]  Winding1=[110000,0.002,0.08]  Winding2Connection=Yg  Winding2=[110000,0.002,0.08]  SetSaturation=off  Rm=500  Lm=500  Saturation=[ 0,0 ; 0.0024,1.2 ; 1.0,1.52 ]  Hysteresis=off  DataFile='hysteresis'  SetInitialFlux=off  InitialFluxes=[ 0.8 , -0.8 , 0.7 ]  Measurements=None  MoreParameters=off  BreakLoop=off  DataType=off  TransfoNumber=1
  T_58880346_110000;35000;10000_ПС_110_35_10_кВ_Спутник : powerlib/Elements/Three-Phase Transformer (Two Windings)  Winding1Connection=Yg  UNITS=pu  NominalPower=[ 250e6 , 60 ]  Winding1=[110000,0.002,0.08]  Winding2Connection=Yg  Winding2=[110000,0.002,0.08]  SetSaturation=off  Rm=500  Lm=500  Saturation=[ 0,0 ; 0.0024,1.2 ; 1.0,1.52 ]  Hysteresis=off  DataFile='hysteresis'  SetInitialFlux=off  InitialFluxes=[ 0.8 , -0.8 , 0.7 ]  Measurements=None  MoreParameters=off  BreakLoop=off  DataType=off  TransfoNumber=1
  T_62194541_220000_ПС_Магистральная : powerlib/Elements/Three-Phase Transformer (Two Windings)  Winding1Connection=Yg  UNITS=pu  NominalPower=[ 250e6 , 60 ]  Winding1=[220000,0.002,0.08]  Winding2Connection=Yg  Winding2=[220000,0.002,0.08]  SetSaturation=off  Rm=500  Lm=500  Saturation=[ 0,0 ; 0.0024,1.2 ; 1.0,1.52 ]  Hysteresis=off  DataFile='hysteresis'  SetInitialFlux=off  InitialFluxes=[ 0.8 , -0.8 , 0.7 ]  Measurements=None  MoreParameters=off  BreakLoop=off  DataType=off  TransfoNumber=1
  T_67498838__ПС_Заводская : powerlib/Elements/Three-Phase Transformer (Two Windings)  Winding1Connection=Yg  UNITS=pu  NominalPower=[ 250e6 , 60 ]  Winding1=[110000,0.002,0.08]  Winding2Connection=Yg  Winding2=[110000,0.002,0.08]  SetSaturation=off  Rm=500  Lm=500  Saturation=[ 0,0 ; 0.0024,1.2 ; 1.0,1.52 ]  Hysteresis=off  DataFile='hysteresis'  SetInitialFlux=off  InitialFluxes=[ 0.8 , -0.8 , 0.7 ]  Measurements=None  MoreParameters=off  BreakLoop=off  DataType=off  TransfoNumber=1
  T_70186926_110000;fixme_Дубравная : powerlib/Elements/Three-Phase Transformer (Two Windings)  Winding1Connection=Yg  UNITS=pu  NominalPower=[ 250e6 , 60 ]  Winding1=[110000,0.002,0.08]  Winding2Connection=Yg  Winding2=[110000,0.002,0.08]  SetSaturation=off  Rm=500  Lm=500  Saturation=[ 0,0 ; 0.0024,1.2 ; 1.0,1.52 ]  Hysteresis=off  DataFile='hysteresis'  SetInitialFlux=off  InitialFluxes=[ 0.8 , -0.8 , 0.7 ]  Measurements=None  MoreParameters=off  BreakLoop=off  DataType=off  TransfoNumber=1
  T_70186927_110000;fixme_ЗКПД : powerlib/Elements/Three-Phase Transformer (Two Windings)  Winding1Connection=Yg  UNITS=pu  NominalPower=[ 250e6 , 60 ]  Winding1=[110000,0.002,0.08]  Winding2Connection=Yg  Winding2=[110000,0.002,0.08]  SetSaturation=off  Rm=500  Lm=500  Saturation=[ 0,0 ; 0.0024,1.2 ; 1.0,1.52 ]  Hysteresis=off  DataFile='hysteresis'  SetInitialFlux=off  InitialFluxes=[ 0.8 , -0.8 , 0.7 ]  Measurements=None  MoreParameters=off  BreakLoop=off  DataType=off  TransfoNumber=1
  T_72288676_500000_Арзамасская : powerlib/Elements/Three-Phase Transformer (Two Windings)  Winding1Connection=Yg  UNITS=pu  NominalPower=[ 250e6 , 60 ]  Winding1=[500000,0.002,0.08]  Winding2Connection=Yg  Winding2=[220000,0.002,0.08]  SetSaturation=off  Rm=500  Lm=500  Saturation=[ 0,0 ; 0.0024,1.2 ; 1.0,1.52 ]  Hysteresis=off  DataFile='hysteresis'  SetInitialFlux=off  InitialFluxes=[ 0.8 , -0.8 , 0.7 ]  Measurements=None  MoreParameters=off  BreakLoop=off  DataType=off  TransfoNumber=1
  T_82458858_220000_ОРУ_220_кВ : powerlib/Elements/Three-Phase Transformer (Two Windings)  Winding1Connection=Yg  UNITS=pu  NominalPower=[ 250e6 , 60 ]  Winding1=[220000,0.002,0.08]  Winding2Connection=Yg  Winding2=[220000,0.002,0.08]  SetSaturation=off  Rm=500  Lm=500  Saturation=[ 0,0 ; 0.0024,1.2 ; 1.0,1.52 ]  Hysteresis=off  DataFile='hysteresis'  SetInitialFlux=off  InitialFluxes=[ 0.8 , -0.8 , 0.7 ]  Measurements=None  MoreParameters=off  BreakLoop=off  DataType=off  TransfoNumber=1
  T_82459105_500000_ОРУ_500_кВ : powerlib/Elements/Three-Phase Transformer (Two Windings)  Winding1Connection=Yg  UNITS=pu  NominalPower=[ 250e6 , 60 ]  Winding1=[500000,0.002,0.08]  Winding2Connection=Yg  Winding2=[500000,0.002,0.08]  SetSaturation=off  Rm=500  Lm=500  Saturation=[ 0,0 ; 0.0024,1.2 ; 1.0,1.52 ]  Hysteresis=off  DataFile='hysteresis'  SetInitialFlux=off  InitialFluxes=[ 0.8 , -0.8 , 0.7 ]  Measurements=None  MoreParameters=off  BreakLoop=off  DataType=off  TransfoNumber=1
  T_82459148_110000_ОРУ_110_кВ : powerlib/Elements/Three-Phase Transformer (Two Windings)  Winding1Connection=Yg  UNITS=pu  NominalPower=[ 250e6 , 60 ]  Winding1=[110000,0.002,0.08]  Winding2Connection=Yg  Winding2=[110000,0.002,0.08]  SetSaturation=off  Rm=500  Lm=500  Saturation=[ 0,0 ; 0.0024,1.2 ; 1.0,1.52 ]  Hysteresis=off  DataFile='hysteresis'  SetInitialFlux=off  InitialFluxes=[ 0.8 , -0.8 , 0.7 ]  Measurements=None  MoreParameters=off  BreakLoop=off  DataType=off  TransfoNumber=1
  T_82967790__ПС_Пенза_2 : powerlib/Elements/Three-Phase Transformer (Two Windings)  Winding1Connection=Yg  UNITS=pu  NominalPower=[ 250e6 , 60 ]  Winding1=[500000,0.002,0.08]  Winding2Connection=Yg  Winding2=[500000,0.002,0.08]  SetSaturation=off  Rm=500  Lm=500  Saturation=[ 0,0 ; 0.0024,1.2 ; 1.0,1.52 ]  Hysteresis=off  DataFile='hysteresis'  SetInitialFlux=off  InitialFluxes=[ 0.8 , -0.8 , 0.7 ]  Measurements=None  MoreParameters=off  BreakLoop=off  DataType=off  TransfoNumber=1
  "T_88028486_500000_ПС_500_кВ_\"Бугульма\"" : powerlib/Elements/Three-Phase Transformer (Two Windings)  Winding1Connection=Yg  UNITS=pu  NominalPower=[ 250e6 , 60 ]  Winding1=[500000,0.002,0.08]  Winding2Connection=Yg  Winding2=[500000,0.002,0.08]  SetSaturation=off  Rm=500  Lm=500  Saturation=[ 0,0 ; 0.0024,1.2 ; 1.0,1.52 ]  Hysteresis=off  DataFile='hysteresis'  SetInitialFlux=off  InitialFluxes=[ 0.8 , -0.8 , 0.7 ]  Measurements=None  MoreParameters=off  BreakLoop=off  DataType=off  TransfoNumber=1
  T_89430545__ПС_Киндери : powerlib/Elements/Three-Phase Transformer (Two Windings)  Winding1Connection=Yg  UNITS=pu  NominalPower=[ 250e6 , 60 ]  Winding1=[500000,0.002,0.08]  Winding2Connection=Yg  Winding2=[220000,0.002,0.08]  SetSaturation=off  Rm=500  Lm=500  Saturation=[ 0,0 ; 0.0024,1.2 ; 1.0,1.52 ]  Hysteresis=off  DataFile='hysteresis'  SetInitialFlux=off  InitialFluxes=[ 0.8 , -0.8 , 0.7 ]  Measurements=None  MoreParameters=off  BreakLoop=off  DataType=off  TransfoNumber=1
  T_90273320__Курдюм : powerlib/Elements/Three-Phase Transformer (Two Windings)  Winding1Connection=Yg  UNITS=pu  NominalPower=[ 250e6 , 60 ]  Winding1=[500000,0.002,0.08]  Winding2Connection=Yg  Winding2=[500000,0.002,0.08]  SetSaturation=off  Rm=500  Lm=500  Saturation=[ 0,0 ; 0.0024,1.2 ; 1.0,1.52 ]  Hysteresis=off  DataFile='hysteresis'  SetInitialFlux=off  InitialFluxes=[ 0.8 , -0.8 , 0.7 ]  Measurements=None  MoreParameters=off  BreakLoop=off  DataType=off  TransfoNumber=1
  T_90682372__ : powerlib/Elements/Three-Phase Transformer (Two Windings)  Winding1Connection=Yg  UNITS=pu  NominalPower=[ 250e6 , 60 ]  Winding1=[110000,0.002,0.08]  Winding2Connection=Yg  Winding2=[110000,0.002,0.08]  SetSaturation=off  Rm=500  Lm=500  Saturation=[ 0,0 ; 0.0024,1.2 ; 1.0,1.52 ]  Hysteresis=off  DataFile='hysteresis'  SetInitialFlux=off  InitialFluxes=[ 0.8 , -0.8 , 0.7 ]  Measurements=None  MoreParameters=off  BreakLoop=off  DataType=off  TransfoNumber=1
  T_90868997__ : powerlib/Elements/Three-Phase Transformer (Two Windings)  Winding1Connection=Yg  UNITS=pu  NominalPower=[ 250e6 , 60 ]  Winding1=[110000,0.002,0.08]  Winding2Connection=Yg  Winding2=[110000,0.002,0.08]  SetSaturation=off  Rm=500  Lm=500  Saturation=[ 0,0 ; 0.0024,1.2 ; 1.0,1.52 ]  Hysteresis=off  DataFile='hysteresis'  SetInitialFlux=off  InitialFluxes=[ 0.8 , -0.8 , 0.7 ]  Measurements=None  MoreParameters=off  BreakLoop=off  DataType=off  TransfoNumber=1
  T_92325642_500000_Радуга : powerlib/Elements/Three-Phase Transformer (Two Windings)  Winding1Connection=Yg  UNITS=pu  NominalPower=[ 250e6 , 60 ]  Winding1=[500000,0.002,0.08]  Winding2Connection=Yg  Winding2=[500000,0.002,0.08]  SetSaturation=off  Rm=500  Lm=500  Saturation=[ 0,0 ; 0.0024,1.2 ; 1.0,1.52 ]  Hysteresis=off  DataFile='hysteresis'  SetInitialFlux=off  InitialFluxes=[ 0.8 , -0.8 , 0.7 ]  Measurements=None  MoreParameters=off  BreakLoop=off  DataType=off  TransfoNumber=1
  T_92419131_500000_Осиновка : powerlib/Elements/Three-Phase Transformer (Two Windings)  Winding1Connection=Yg  UNITS=pu  NominalPower=[ 250e6 , 60 ]  Winding1=[500000,0.002,0.08]  Winding2Connection=Yg  Winding2=[220000,0.002,0.08]  SetSaturation=off  Rm=500  Lm=500  Saturation=[ 0,0 ; 0.0024,1.2 ; 1.0,1.52 ]  Hysteresis=off  DataFile='hysteresis'  SetInitialFlux=off  InitialFluxes=[ 0.8 , -0.8 , 0.7 ]  Measurements=None  MoreParameters=off  BreakLoop=off  DataType=off  TransfoNumber=1
  T_93292147_500000_ПС_Помары : powerlib/Elements/Three-Phase Transformer (Two Windings)  Winding1Connection=Yg  UNITS=pu  NominalPower=[ 250e6 , 60 ]  Winding1=[500000,0.002,0.08]  Winding2Connection=Yg  Winding2=[220000,0.002,0.08]  SetSaturation=off  Rm=500  Lm=500  Saturation=[ 0,0 ; 0.0024,1.2 ; 1.0,1.52 ]  Hysteresis=off  DataFile='hysteresis'  SetInitialFlux=off  InitialFluxes=[ 0.8 , -0.8 , 0.7 ]  Measurements=None  MoreParameters=off  BreakLoop=off  DataType=off  TransfoNumber=1
  T_93482493__ : powerlib/Elements/Three-Phase Transformer (Two Windings)  Winding1Connection=Yg  UNITS=pu  NominalPower=[ 250e6 , 60 ]  Winding1=[110000,0.002,0.08]  Winding2Connection=Yg  Winding2=[110000,0.002,0.08]  SetSaturation=off  Rm=500  Lm=500  Saturation=[ 0,0 ; 0.0024,1.2 ; 1.0,1.52 ]  Hysteresis=off  DataFile='hysteresis'  SetInitialFlux=off  InitialFluxes=[ 0.8 , -0.8 , 0.7 ]  Measurements=None  MoreParameters=off  BreakLoop=off  DataType=off  TransfoNumber=1
  T_93482528__ : powerlib/Elements/Three-Phase Transformer (Two Windings)  Winding1Connection=Yg  UNITS=pu  NominalPower=[ 250e6 , 60 ]  Winding1=[110000,0.002,0.08]  Winding2Connection=Yg  Winding2=[110000,0.002,0.08]  SetSaturation=off  Rm=500  Lm=500  Saturation=[ 0,0 ; 0.0024,1.2 ; 1.0,1.52 ]  Hysteresis=off  DataFile='hysteresis'  SetInitialFlux=off  InitialFluxes=[ 0.8 , -0.8 , 0.7 ]  Measurements=None  MoreParameters=off  BreakLoop=off  DataType=off  TransfoNumber=1
  T_93494543_220000_Сеченово_1 : powerlib/Elements/Three-Phase Transformer (Two Windings)  Winding1Connection=Yg  UNITS=pu  NominalPower=[ 250e6 , 60 ]  Winding1=[220000,0.002,0.08]  Winding2Connection=Yg  Winding2=[220000,0.002,0.08]  SetSaturation=off  Rm=500  Lm=500  Saturation=[ 0,0 ; 0.0024,1.2 ; 1.0,1.52 ]  Hysteresis=off  DataFile='hysteresis'  SetInitialFlux=off  InitialFluxes=[ 0.8 , -0.8 , 0.7 ]  Measurements=None  MoreParameters=off  BreakLoop=off  DataType=off  TransfoNumber=1
  T_93494546_220000_РП_Сеченово : powerlib/Elements/Three-Phase Transformer (Two Windings)  Winding1Connection=Yg  UNITS=pu  NominalPower=[ 250e6 , 60 ]  Winding1=[220000,0.002,0.08]  Winding2Connection=Yg  Winding2=[220000,0.002,0.08]  SetSaturation=off  Rm=500  Lm=500  Saturation=[ 0,0 ; 0.0024,1.2 ; 1.0,1.52 ]  Hysteresis=off  DataFile='hysteresis'  SetInitialFlux=off  InitialFluxes=[ 0.8 , -0.8 , 0.7 ]  Measurements=None  MoreParameters=off  BreakLoop=off  DataType=off  TransfoNumber=1
  T_93508340_220000_Сеченово_2 : powerlib/Elements/Three-Phase Transformer (Two Windings)  Winding1Connection=Yg  UNITS=pu  NominalPower=[ 250e6 , 60 ]  Winding1=[220000,0.002,0.08]  Winding2Connection=Yg  Winding2=[220000,0.002,0.08]  SetSaturation=off  Rm=500  Lm=500  Saturation=[ 0,0 ; 0.0024,1.2 ; 1.0,1.52 ]  Hysteresis=off  DataFile='hysteresis'  SetInitialFlux=off  InitialFluxes=[ 0.8 , -0.8 , 0.7 ]  Measurements=None  MoreParameters=off  BreakLoop=off  DataType=off  TransfoNumber=1
  T_94214974__ПС_Нижнекамская : powerlib/Elements/Three-Phase Transformer (Two Windings)  Winding1Connection=Yg  UNITS=pu  NominalPower=[ 250e6 , 60 ]  Winding1=[220000,0.002,0.08]  Winding2Connection=Yg  Winding2=[110000,0.002,0.08]  SetSaturation=off  Rm=500  Lm=500  Saturation=[ 0,0 ; 0.0024,1.2 ; 1.0,1.52 ]  Hysteresis=off  DataFile='hysteresis'  SetInitialFlux=off  InitialFluxes=[ 0.8 , -0.8 , 0.7 ]  Measurements=None  MoreParameters=off  BreakLoop=off  DataType=off  TransfoNumber=1
  T_94242892__Подстанция_№3 : powerlib/Elements/Three-Phase Transformer (Two Windings)  Winding1Connection=Yg  UNITS=pu  NominalPower=[ 250e6 , 60 ]  Winding1=[110000,0.002,0.08]  Winding2Connection=Yg  Winding2=[110000,0.002,0.08]  SetSaturation=off  Rm=500  Lm=500  Saturation=[ 0,0 ; 0.0024,1.2 ; 1.0,1.52 ]  Hysteresis=off  DataFile='hysteresis'  SetInitialFlux=off  InitialFluxes=[ 0.8 , -0.8 , 0.7 ]  Measurements=None  MoreParameters=off  BreakLoop=off  DataType=off  TransfoNumber=1
  T_95488500__ПС_Письмянка : powerlib/Elements/Three-Phase Transformer (Two Windings)  Winding1Connection=Yg  UNITS=pu  NominalPower=[ 250e6 , 60 ]  Winding1=[220000,0.002,0.08]  Winding2Connection=Yg  Winding2=[220000,0.002,0.08]  SetSaturation=off  Rm=500  Lm=500  Saturation=[ 0,0 ; 0.0024,1.2 ; 1.0,1.52 ]  Hysteresis=off  DataFile='hysteresis'  SetInitialFlux=off  InitialFluxes=[ 0.8 , -0.8 , 0.7 ]  Measurements=None  MoreParameters=off  BreakLoop=off  DataType=off  TransfoNumber=1
  T_95488527_220000;110000;35000;6000_ПС_Абдрахманово : powerlib/Elements/Three-Phase Transformer (Two Windings)  Winding1Connection=Yg  UNITS=pu  NominalPower=[ 250e6 , 60 ]  Winding1=[220000,0.002,0.08]  Winding2Connection=Yg  Winding2=[220000,0.002,0.08]  SetSaturation=off  Rm=500  Lm=500  Saturation=[ 0,0 ; 0.0024,1.2 ; 1.0,1.52 ]  Hysteresis=off  DataFile='hysteresis'  SetInitialFlux=off  InitialFluxes=[ 0.8 , -0.8 , 0.7 ]  Measurements=None  MoreParameters=off  BreakLoop=off  DataType=off  TransfoNumber=1
  T_96563667__ : powerlib/Elements/Three-Phase Transformer (Two Windings)  Winding1Connection=Yg  UNITS=pu  NominalPower=[ 250e6 , 60 ]  Winding1=[220000,0.002,0.08]  Winding2Connection=Yg  Winding2=[220000,0.002,0.08]  SetSaturation=off  Rm=500  Lm=500  Saturation=[ 0,0 ; 0.0024,1.2 ; 1.0,1.52 ]  Hysteresis=off  DataFile='hysteresis'  SetInitialFlux=off  InitialFluxes=[ 0.8 , -0.8 , 0.7 ]  Measurements=None  MoreParameters=off  BreakLoop=off  DataType=off  TransfoNumber=1
  T_96826924_220000;110000;10000_ПС_220_кВ_Новотроицкая : powerlib/Elements/Three-Phase Transformer (Two Windings)  Winding1Connection=Yg  UNITS=pu  NominalPower=[ 250e6 , 60 ]  Winding1=[220000,0.002,0.08]  Winding2Connection=Yg  Winding2=[220000,0.002,0.08]  SetSaturation=off  Rm=500  Lm=500  Saturation=[ 0,0 ; 0.0024,1.2 ; 1.0,1.52 ]  Hysteresis=off  DataFile='hysteresis'  SetInitialFlux=off  InitialFluxes=[ 0.8 , -0.8 , 0.7 ]  Measurements=None  MoreParameters=off  BreakLoop=off  DataType=off  TransfoNumber=1
  T_97060032__ : powerlib/Elements/Three-Phase Transformer (Two Windings)  Winding1Connection=Yg  UNITS=pu  NominalPower=[ 250e6 , 60 ]  Winding1=[110000,0.002,0.08]  Winding2Connection=Yg  Winding2=[110000,0.002,0.08]  SetSaturation=off  Rm=500  Lm=500  Saturation=[ 0,0 ; 0.0024,1.2 ; 1.0,1.52 ]  Hysteresis=off  DataFile='hysteresis'  SetInitialFlux=off  InitialFluxes=[ 0.8 , -0.8 , 0.7 ]  Measurements=None  MoreParameters=off  BreakLoop=off  DataType=off  TransfoNumber=1
  T_97060037__ : powerlib/Elements/Three-Phase Transformer (Two Windings)  Winding1Connection=Yg  UNITS=pu  NominalPower=[ 250e6 , 60 ]  Winding1=[110000,0.002,0.08]  Winding2Connection=Yg  Winding2=[110000,0.002,0.08]  SetSaturation=off  Rm=500  Lm=500  Saturation=[ 0,0 ; 0.0024,1.2 ; 1.0,1.52 ]  Hysteresis=off  DataFile='hysteresis'  SetInitialFlux=off  InitialFluxes=[ 0.8 , -0.8 , 0.7 ]  Measurements=None  MoreParameters=off  BreakLoop=off  DataType=off  TransfoNumber=1
  T_97124768__ : powerlib/Elements/Three-Phase Transformer (Two Windings)  Winding1Connection=Yg  UNITS=pu  NominalPower=[ 250e6 , 60 ]  Winding1=[110000,0.002,0.08]  Winding2Connection=Yg  Winding2=[110000,0.002,0.08]  SetSaturation=off  Rm=500  Lm=500  Saturation=[ 0,0 ; 0.0024,1.2 ; 1.0,1.52 ]  Hysteresis=off  DataFile='hysteresis'  SetInitialFlux=off  InitialFluxes=[ 0.8 , -0.8 , 0.7 ]  Measurements=None  MoreParameters=off  BreakLoop=off  DataType=off  TransfoNumber=1
  T_97124903__ : powerlib/Elements/Three-Phase Transformer (Two Windings)  Winding1Connection=Yg  UNITS=pu  NominalPower=[ 250e6 , 60 ]  Winding1=[110000,0.002,0.08]  Winding2Connection=Yg  Winding2=[110000,0.002,0.08]  SetSaturation=off  Rm=500  Lm=500  Saturation=[ 0,0 ; 0.0024,1.2 ; 1.0,1.52 ]  Hysteresis=off  DataFile='hysteresis'  SetInitialFlux=off  InitialFluxes=[ 0.8 , -0.8 , 0.7 ]  Measurements=None  MoreParameters=off  BreakLoop=off  DataType=off  TransfoNumber=1
  T_97145033_220000;110000;10000_ПС_220_кВ_Орская : powerlib/Elements/Three-Phase Transformer (Two Windings)  Winding1Connection=Yg  UNITS=pu  NominalPower=[ 250e6 , 60 ]  Winding1=[220000,0.002,0.08]  Winding2Connection=Yg  Winding2=[110000,0.002,0.08]  SetSaturation=off  Rm=500  Lm=500  Saturation=[ 0,0 ; 0.0024,1.2 ; 1.0,1.52 ]  Hysteresis=off  DataFile='hysteresis'  SetInitialFlux=off  InitialFluxes=[ 0.8 , -0.8 , 0.7 ]  Measurements=None  MoreParameters=off  BreakLoop=off  DataType=off  TransfoNumber=1
  "T_99190583_500000;220000;110000;fixme_\"Смеловская\"_500_кВ" : powerlib/Elements/Three-Phase Transformer (Two Windings)  Winding1Connection=Yg  UNITS=pu  NominalPower=[ 250e6 , 60 ]  Winding1=[500000,0.002,0.08]  Winding2Connection=Yg  Winding2=[500000,0.002,0.08]  SetSaturation=off  Rm=500  Lm=500  Saturation=[ 0,0 ; 0.0024,1.2 ; 1.0,1.52 ]  Hysteresis=off  DataFile='hysteresis'  SetInitialFlux=off  InitialFluxes=[ 0.8 , -0.8 , 0.7 ]  Measurements=None  MoreParameters=off  BreakLoop=off  DataType=off  TransfoNumber=1
  _CN_102447718_110000_CN_308883878_110000 : powerlib/Elements/Distributed Parameters Line  Phases=3  Frequency=60  Resistance=[0.01273 0.3864]  Inductance="[0.9337e-3  4.1264e-3]"  Capacitance=[12.74e-9 7.751e-9]  Length=14.9368  x1=[0 0 0 0; 0.0001244 0 0 0; 0.0002488 0 0 0; 0.0003733 0 0 0; 0.0004977 0 0 0; 0.0006221 0 0 0]  x2=[0 0 0 0; 0.0001244 0 0 0; 0.0002488 0 0 0; 0.0003733 0 0 0; 0.0004977 0 0 0; 0.0006221 0 0 0]  x3=[0 0 0 0; 0.0001244 0 0 0; 0.0002488 0 0 0; 0.0003733 0 0 0; 0.0004977 0 0 0; 0.0006221 0 0 0]  x4=[0 0 0 0; 0.0001244 0 0 0; 0.0002488 0 0 0; 0.0003733 0 0 0; 0.0004977 0 0 0; 0.0006221 0 0 0]  x5=0  V1=ones(3,3)  V2=ones(3,3)  I1=ones(3,3)  I2=ones(3,3)  nHarmo=1  Measurements=None
  _CN_103877395_110000_CN_103877470_110000 : powerlib/Elements/Distributed Parameters Line  Phases=3  Frequency=60  Resistance=[0.01273 0.3864]  Inductance="[0.9337e-3  4.1264e-3]"  Capacitance=[12.74e-9 7.751e-9]  Length=22.0437  x1=[0 0 0 0; 0.0001244 0 0 0; 0.0002488 0 0 0; 0.0003733 0 0 0; 0.0004977 0 0 0; 0.0006221 0 0 0]  x2=[0 0 0 0; 0.0001244 0 0 0; 0.0002488 0 0 0; 0.0003733 0 0 0; 0.0004977 0 0 0; 0.0006221 0 0 0]  x3=[0 0 0 0; 0.0001244 0 0 0; 0.0002488 0 0 0; 0.0003733 0 0 0; 0.0004977 0 0 0; 0.0006221 0 0 0]  x4=[0 0 0 0; 0.0001244 0 0 0; 0.0002488 0 0 0; 0.0003733 0 0 0; 0.0004977 0 0 0; 0.0006221 0 0 0]  x5=0  V1=ones(3,3)  V2=ones(3,3)  I1=ones(3,3)  I2=ones(3,3)  nHarmo=1  Measurements=None
  _CN_104554513_110000_CN_320965592_110000 : powerlib/Elements/Distributed Parameters Line  Phases=3  Frequency=60  Resistance=[0.01273 0.3864]  Inductance="[0.9337e-3  4.1264e-3]"  Capacitance=[12.74e-9 7.751e-9]  Length=18.3334  x1=[0 0 0 0; 0.0001244 0 0 0; 0.0002488 0 0 0; 0.0003733 0 0 0; 0.0004977 0 0 0; 0.0006221 0 0 0]  x2=[0 0 0 0; 0.0001244 0 0 0; 0.0002488 0 0 0; 0.0003733 0 0 0; 0.0004977 0 0 0; 0.0006221 0 0 0]  x3=[0 0 0 0; 0.0001244 0 0 0; 0.0002488 0 0 0; 0.0003733 0 0 0; 0.0004977 0 0 0; 0.0006221 0 0 0]  x4=[0 0 0 0; 0.0001244 0 0 0; 0.0002488 0 0 0; 0.0003733 0 0 0; 0.0004977 0 0 0; 0.0006221 0 0 0]  x5=0  V1=ones(3,3)  V2=ones(3,3)  I1=ones(3,3)  I2=ones(3,3)  nHarmo=1  Measurements=None
  _CN_104554513_110000_CN_67498838_110000 : powerlib/Elements/Distributed Parameters Line  Phases=3  Frequency=60  Resistance=[0.01273 0.3864]  Inductance="[0.9337e-3  4.1264e-3]"  Capacitance=[12.74e-9 7.751e-9]  Length=4.6544  x1=[0 0 0 0; 0.0001244 0 0 0; 0.0002488 0 0 0; 0.0003733 0 0 0; 0.0004977 0 0 0; 0.0006221 0 0 0]  x2=[0 0 0 0; 0.0001244 0 0 0; 0.0002488 0 0 0; 0.0003733 0 0 0; 0.0004977 0 0 0; 0.0006221 0 0 0]  x3=[0 0 0 0; 0.0001244 0 0 0; 0.0002488 0 0 0; 0.0003733 0 0 0; 0.0004977 0 0 0; 0.0006221 0 0 0]  x4=[0 0 0 0; 0.0001244 0 0 0; 0.0002488 0 0 0; 0.0003733 0 0 0; 0.0004977 0 0 0; 0.0006221 0 0 0]  x5=0  V1=ones(3,3)  V2=ones(3,3)  I1=ones(3,3)  I2=ones(3,3)  nHarmo=1  Measurements=None
  _CN_104554513_110000_CN_93482528_110000 : powerlib/Elements/Distributed Parameters Line  Phases=3  Frequency=60  Resistance=[0.01273 0.3864]  Inductance="[0.9337e-3  4.1264e-3]"  Capacitance=[12.74e-9 7.751e-9]  Length=4.7625  x1=[0 0 0 0; 0.0001244 0 0 0; 0.0002488 0 0 0; 0.0003733 0 0 0; 0.0004977 0 0 0; 0.0006221 0 0 0]  x2=[0 0 0 0; 0.0001244 0 0 0; 0.0002488 0 0 0; 0.0003733 0 0 0; 0.0004977 0 0 0; 0.0006221 0 0 0]  x3=[0 0 0 0; 0.0001244 0 0 0; 0.0002488 0 0 0; 0.0003733 0 0 0; 0.0004977 0 0 0; 0.0006221 0 0 0]  x4=[0 0 0 0; 0.0001244 0 0 0; 0.0002488 0 0 0; 0.0003733 0 0 0; 0.0004977 0 0 0; 0.0006221 0 0 0]  x5=0  V1=ones(3,3)  V2=ones(3,3)  I1=ones(3,3)  I2=ones(3,3)  nHarmo=1  Measurements=None
  _CN_106289362_110000_CN_106289442_110000 : powerlib/Elements/Distributed Parameters Line  Phases=3  Frequency=60  Resistance=[0.01273 0.3864]  Inductance="[0.9337e-3  4.1264e-3]"  Capacitance=[12.74e-9 7.751e-9]  Length=59.1626  x1=[0 0 0 0; 0.0001244 0 0 0; 0.0002488 0 0 0; 0.0003733 0 0 0; 0.0004977 0 0 0; 0.0006221 0 0 0]  x2=[0 0 0 0; 0.0001244 0 0 0; 0.0002488 0 0 0; 0.0003733 0 0 0; 0.0004977 0 0 0; 0.0006221 0 0 0]  x3=[0 0 0 0; 0.0001244 0 0 0; 0.0002488 0 0 0; 0.0003733 0 0 0; 0.0004977 0 0 0; 0.0006221 0 0 0]  x4=[0 0 0 0; 0.0001244 0 0 0; 0.0002488 0 0 0; 0.0003733 0 0 0; 0.0004977 0 0 0; 0.0006221 0 0 0]  x5=0  V1=ones(3,3)  V2=ones(3,3)  I1=ones(3,3)  I2=ones(3,3)  nHarmo=1  Measurements=None
  _CN_107692183_110000_CN_107881747_110000 : powerlib/Elements/Distributed Parameters Line  Phases=3  Frequency=60  Resistance=[0.01273 0.3864]  Inductance="[0.9337e-3  4.1264e-3]"  Capacitance=[12.74e-9 7.751e-9]  Length=3.188  x1=[0 0 0 0; 0.0001244 0 0 0; 0.0002488 0 0 0; 0.0003733 0 0 0; 0.0004977 0 0 0; 0.0006221 0 0 0]  x2=[0 0 0 0; 0.0001244 0 0 0; 0.0002488 0 0 0; 0.0003733 0 0 0; 0.0004977 0 0 0; 0.0006221 0 0 0]  x3=[0 0 0 0; 0.0001244 0 0 0; 0.0002488 0 0 0; 0.0003733 0 0 0; 0.0004977 0 0 0; 0.0006221 0 0 0]  x4=[0 0 0 0; 0.0001244 0 0 0; 0.0002488 0 0 0; 0.0003733 0 0 0; 0.0004977 0 0 0; 0.0006221 0 0 0]  x5=0  V1=ones(3,3)  V2=ones(3,3)  I1=ones(3,3)  I2=ones(3,3)  nHarmo=1  Measurements=None
  _CN_107692183_110000_CN_107943661_110000 : powerlib/Elements/Distributed Parameters Line  Phases=3  Frequency=60  Resistance=[0.01273 0.3864]  Inductance="[0.9337e-3  4.1264e-3]"  Capacitance=[12.74e-9 7.751e-9]  Length=12.6061  x1=[0 0 0 0; 0.0001244 0 0 0; 0.0002488 0 0 0; 0.0003733 0 0 0; 0.0004977 0 0 0; 0.0006221 0 0 0]  x2=[0 0 0 0; 0.0001244 0 0 0; 0.0002488 0 0 0; 0.0003733 0 0 0; 0.0004977 0 0 0; 0.0006221 0 0 0]  x3=[0 0 0 0; 0.0001244 0 0 0; 0.0002488 0 0 0; 0.0003733 0 0 0; 0.0004977 0 0 0; 0.0006221 0 0 0]  x4=[0 0 0 0; 0.0001244 0 0 0; 0.0002488 0 0 0; 0.0003733 0 0 0; 0.0004977 0 0 0; 0.0006221 0 0 0]  x5=0  V1=ones(3,3)  V2=ones(3,3)  I1=ones(3,3)  I2=ones(3,3)  nHarmo=1  Measurements=None
  _CN_107942401_110000_CN_107881747_110000 : powerlib/Elements/Distributed Parameters Line  Phases=3  Frequency=60  Resistance=[0.01273 0.3864]  Inductance="[0.9337e-3  4.1264e-3]"  Capacitance=[12.74e-9 7.751e-9]  Length=2.3671  x1=[0 0 0 0; 0.0001244 0 0 0; 0.0002488 0 0 0; 0.0003733 0 0 0; 0.0004977 0 0 0; 0.0006221 0 0 0]  x2=[0 0 0 0; 0.0001244 0 0 0; 0.0002488 0 0 0; 0.0003733 0 0 0; 0.0004977 0 0 0; 0.0006221 0 0 0]  x3=[0 0 0 0; 0.0001244 0 0 0; 0.0002488 0 0 0; 0.0003733 0 0 0; 0.0004977 0 0 0; 0.0006221 0 0 0]  x4=[0 0 0 0; 0.0001244 0 0 0; 0.0002488 0 0 0; 0.0003733 0 0 0; 0.0004977 0 0 0; 0.0006221 0 0 0]  x5=0  V1=ones(3,3)  V2=ones(3,3)  I1=ones(3,3)  I2=ones(3,3)  nHarmo=1  Measurements=None
  _CN_108403292_110000_CN_62191058_110000 : powerlib/Elements/Distributed Parameters Line  Phases=3  Frequency=60  Resistance=[0.01273 0.3864]  Inductance="[0.9337e-3  4.1264e-3]"  Capacitance=[12.74e-9 7.751e-9]  Length=9.0238  x1=[0 0 0 0; 0.0001244 0 0 0; 0.0002488 0 0 0; 0.0003733 0 0 0; 0.0004977 0 0 0; 0.0006221 0 0 0]  x2=[0 0 0 0; 0.0001244 0 0 0; 0.0002488 0 0 0; 0.0003733 0 0 0; 0.0004977 0 0 0; 0.0006221 0 0 0]  x3=[0 0 0 0; 0.0001244 0 0 0; 0.0002488 0 0 0; 0.0003733 0 0 0; 0.0004977 0 0 0; 0.0006221 0 0 0]  x4=[0 0 0 0; 0.0001244 0 0 0; 0.0002488 0 0 0; 0.0003733 0 0 0; 0.0004977 0 0 0; 0.0006221 0 0 0]  x5=0  V1=ones(3,3)  V2=ones(3,3)  I1=ones(3,3)  I2=ones(3,3)  nHarmo=1  Measurements=None
  _CN_108403292_110000_CN_94214974_110000 : powerlib/Elements/Distributed Parameters Line  Phases=3  Frequency=60  Resistance=[0.01273 0.3864]  Inductance="[0.9337e-3  4.1264e-3]"  Capacitance=[12.74e-9 7.751e-9]  Length=54.1725  x1=[0 0 0 0; 0.0001244 0 0 0; 0.0002488 0 0 0; 0.0003733 0 0 0; 0.0004977 0 0 0; 0.0006221 0 0 0]  x2=[0 0 0 0; 0.0001244 0 0 0; 0.0002488 0 0 0; 0.0003733 0 0 0; 0.0004977 0 0 0; 0.0006221 0 0 0]  x3=[0 0 0 0; 0.0001244 0 0 0; 0.0002488 0 0 0; 0.0003733 0 0 0; 0.0004977 0 0 0; 0.0006221 0 0 0]  x4=[0 0 0 0; 0.0001244 0 0 0; 0.0002488 0 0 0; 0.0003733 0 0 0; 0.0004977 0 0 0; 0.0006221 0 0 0]  x5=0  V1=ones(3,3)  V2=ones(3,3)  I1=ones(3,3)  I2=ones(3,3)  nHarmo=1  Measurements=None
  _CN_109525394_110000_CN_109525404_110000 : powerlib/Elements/Distributed Parameters Line  Phases=3  Frequency=60  Resistance=[0.01273 0.3864]  Inductance="[0.9337e-3  4.1264e-3]"  Capacitance=[12.74e-9 7.751e-9]  Length=27.3864  x1=[0 0 0 0; 0.0001244 0 0 0; 0.0002488 0 0 0; 0.0003733 0 0 0; 0.0004977 0 0 0; 0.0006221 0 0 0]  x2=[0 0 0 0; 0.0001244 0 0 0; 0.0002488 0 0 0; 0.0003733 0 0 0; 0.0004977 0 0 0; 0.0006221 0 0 0]  x3=[0 0 0 0; 0.0001244 0 0 0; 0.0002488 0 0 0; 0.0003733 0 0 0; 0.0004977 0 0 0; 0.0006221 0 0 0]  x4=[0 0 0 0; 0.0001244 0 0 0; 0.0002488 0 0 0; 0.0003733 0 0 0; 0.0004977 0 0 0; 0.0006221 0 0 0]  x5=0  V1=ones(3,3)  V2=ones(3,3)  I1=ones(3,3)  I2=ones(3,3)  nHarmo=1  Measurements=None
  _CN_109525394_110000_CN_109525439_110000 : powerlib/Elements/Distributed Parameters Line  Phases=3  Frequency=60  Resistance=[0.01273 0.3864]  Inductance="[0.9337e-3  4.1264e-3]"  Capacitance=[12.74e-9 7.751e-9]  Length=1.6188  x1=[0 0 0 0; 0.0001244 0 0 0; 0.0002488 0 0 0; 0.0003733 0 0 0; 0.0004977 0 0 0; 0.0006221 0 0 0]  x2=[0 0 0 0; 0.0001244 0 0 0; 0.0002488 0 0 0; 0.0003733 0 0 0; 0.0004977 0 0 0; 0.0006221 0 0 0]  x3=[0 0 0 0; 0.0001244 0 0 0; 0.0002488 0 0 0; 0.0003733 0 0 0; 0.0004977 0 0 0; 0.0006221 0 0 0]  x4=[0 0 0 0; 0.0001244 0 0 0; 0.0002488 0 0 0; 0.0003733 0 0 0; 0.0004977 0 0 0; 0.0006221 0 0 0]  x5=0  V1=ones(3,3)  V2=ones(3,3)  I1=ones(3,3)  I2=ones(3,3)  nHarmo=1  Measurements=None
